simulink model "InverseKinematics_DirectionalController2018b"  (R2018b)
settings: Solver=VariableStepAuto  StartTime=0.0  StopTime=inf  RelTol=1e-3
undefined symbols (not defined in the file): f
libraries: instrumentlib x15, dspnetwork x6
(part 2 of 3)

== matlab function InverseKinematics_DirectionalController2018b/Inverse Kinematics ==
  data: p input; q1 output size=[1 1]; R input; q2 output size=[1 1]; q3 output size=[1 1]; q4 output size=[1 1]; q5 output size=[1 1]; q6 output size=[1 1]; t input
function [q1,q2,q3,q4,q5,q6] = ik_jaco(p,R,t)
%%INPUT 

%Position values from Example 7.1 research paper
%p=[x(1);y(1);z(1)];
%R=[1,0,0;0,0,-1;0,1,0]; %in the simulink model input this as a constant orientation

% ik_jaco determines the inverse kinematics of first version the 6-dof Jaco Robot 
%   The input parameters are the vector p and the matrix R. The procedure
%   taken to determine the joint angles q1,q2,q3,q4,q5,q6 is based on the
%   Polynomial Inverse Kinematic Solution of the Jaco Robot presented by
%   Clément Gosselin from the Université Laval.
% Input Arguments:
% p -> the vector position of the end-efector. p = [x,y,z]
% R -> the rotation matrix representing the orientation of the end-efector

%% Jaco Robot parameters based on the Forward Kinematic
% The following parameters are based on the paper Polynomial Inverse
% Kinematic Solution of the Jaco Robot. The below parameters can be
% changed to meet the parameters of the Jaco Robot that we have at the lab.
b__1 = 0.2755;  %Base to shoulder
a__2 = 0.2900;  %Upper arm length (shoulder to elbow)
b__3 = -0.0070; %Joint 3-4 lateral offset
b__4 = -0.1661; %Distance from elbow to first sub-segment of the first wrist 
%semgment
b__5 = -0.0856; %Distance from end of the first sub-segment to of the first
% wrist segment to end of the first sub-segment of the second wrist segment
b__6 = -0.2028; % Distance from the end of the first sub-segment of the 
% second wrist segment to the center of the hand.
s__r4 = sind(60); %55 degrees is the angle of curvature first wrist segment
s__r5 = sind(60); %55 degrees is the angle of curvature first wrist segment
c__r4 = cosd(60); %55 degrees is the angle of curvature second wrist segment
c__r5 = cosd(60); %55 degrees is the angle of curvature second wrist segment
%% Getting the end-efector orientation and position for later substitution

q__11 = R(1,1);
q__12 = R(1,2);
q__13 = R(1,3);
q__21 = R(2,1);
q__22 = R(2,2);
q__23 = R(2,3);
q__31 = R(3,1);
q__32 = R(3,2);
q__33 = R(3,3);
r__1 = p(1)+(b__6)*q__13;
r__2 = p(2)+(b__6)*q__23;
r__3 = p(3)+(b__6)*q__33;

%% V and W equations, only depends on the robot parameters and end-efector position and orientation
v__1 = -0.4e1 * ((c__r4 + 1) ^ 2) * ((q__13 * q__33 * r__1 ^ 4) + ...
    (((b__1 - r__3) * q__13 ^ 2 + 4 * q__33 * q__23 * r__2 + ...
    (b__1 - r__3) * q__23 ^ 2 + 2 * c__r5 * q__33 * b__5 - 2 * ...
    q__33 ^ 2 * b__1 + 2 * q__33 ^ 2 * r__3) * r__1 ^ 3) + ...
    (q__13 * (-6 * q__33 * r__2 ^ 2 - 3 * q__33 * b__1 ^ 2 + ...
    (2 * c__r5 * b__5 + 6 * q__33 * r__3) * b__1 - 3 * q__33 * ...
    r__3 ^ 2 - 2 * c__r5 * b__5 * r__3 + q__33 * (a__2 ^ 2 + ...
    b__3 ^ 2 - b__4 ^ 2 + b__5 ^ 2)) * r__1 ^ 2) + (((b__1 - ...
    r__3) * (a__2 ^ 2 - b__1 ^ 2 + 2 * r__3 * b__1 + b__3 ^ 2 - ...
    b__4 ^ 2 + b__5 ^ 2 - 3 * r__2 ^ 2 - r__3 ^ 2) * q__13 ^ 2 - ...
    4 * q__23 * q__33 * r__2 ^ 3 + ((-3 * b__1 + 3 * r__3) * ...
    q__23 ^ 2 - 6 * c__r5 * q__33 * b__5 + 6 * q__33 ^ 2 * b__1 - ...
    6 * q__33 ^ 2 * r__3) * r__2 ^ 2 - 2 * q__23 * (-3 * q__33 * ...
    b__1 ^ 2 + (2 * c__r5 * b__5 + 6 * q__33 * r__3) * b__1 - 3 *...
    q__33 * r__3 ^ 2 - 2 * c__r5 * b__5 * r__3 + q__33 * (a__2 ^ 2 ...
    + b__3 ^ 2 - b__4 ^ 2 + b__5 ^ 2)) * r__2 - q__23 ^ 2 * (b__1 -...
    r__3) * (a__2 ^ 2 - b__1 ^ 2 + 2 * r__3 * b__1 + b__3 ^ 2 - ...
    b__4 ^ 2 + b__5 ^ 2 - r__3 ^ 2)) * r__1) - 0.2e1 * (-(q__33 * r__2 ^ 3) ...
    / 0.2e1 + (-0.3e1 / 0.2e1 * q__33 * (b__1 ^ 2) + ((c__r5 * b__5 + 3 * q__33 * r__3)...
    * b__1) - 0.3e1 / 0.2e1 * q__33 * (r__3 ^ 2) - (c__r5 * b__5 * r__3) + ...
    (q__33 * (a__2 ^ 2 + b__3 ^ 2 - b__4 ^ 2 + b__5 ^ 2)) / 0.2e1) * r__2 +...
    (q__23 * (b__1 - r__3) * (a__2 ^ 2 - b__1 ^ 2 + 2 * r__3 * b__1 + b__3 ^ 2 -...
    b__4 ^ 2 + b__5 ^ 2 - r__3 ^ 2))) * q__13 * r__2) * b__4 * ((c__r4 - 1) ^ 2) / s__r4 ^ 3 / b__5;

v__2 = -0.4e1 * ((c__r4 + 1) ^ 2) * b__4 * (-(q__23 * q__33 * r__2 ^ 4) + ...
    (((r__3 - b__1) * q__23 ^ 2 - 4 * q__33 * r__1 * q__13 + (r__3 - b__1) ...
    * q__13 ^ 2 - 2 * c__r5 * q__33 * b__5 + 2 * q__33 ^ 2 * b__1 - 2 * ...
    q__33 ^ 2 * r__3) * r__2 ^ 3) - ((-6 * q__33 * r__1 ^ 2 - 3 * q__33 * ...
    b__1 ^ 2 + (2 * c__r5 * b__5 + 6 * q__33 * r__3) * b__1 - 3 * q__33 * ...
    r__3 ^ 2 - 2 * c__r5 * b__5 * r__3 + q__33 * (a__2 ^ 2 + b__3 ^ 2 - ...
    b__4 ^ 2 + b__5 ^ 2)) * q__23 * r__2 ^ 2) + ((-(b__1 - r__3) * ...
    (a__2 ^ 2 - b__1 ^ 2 + 2 * r__3 * b__1 + b__3 ^ 2 - b__4 ^ 2 + ...
    b__5 ^ 2 - 3 * r__1 ^ 2 - r__3 ^ 2) * q__23 ^ 2 + 4 * r__1 ^ 3 * ...
    q__13 * q__33 + ((3 * b__1 - 3 * r__3) * q__13 ^ 2 + 6 * c__r5 * ...
    q__33 * b__5 - 6 * q__33 ^ 2 * b__1 + 6 * q__33 ^ 2 * r__3) * r__1 ^ 2 ...
    + 2 * q__13 * (-3 * q__33 * b__1 ^ 2 + (2 * c__r5 * b__5 + ...
    6 * q__33 * r__3) * b__1 - 3 * q__33 * r__3 ^ 2 - 2 * c__r5 * b__5 * ...
    r__3 + q__33 * (a__2 ^ 2 + b__3 ^ 2 - b__4 ^ 2 + b__5 ^ 2)) * r__1 + ...
    q__13 ^ 2 * (b__1 - r__3) * (a__2 ^ 2 - b__1 ^ 2 + 2 * r__3 * b__1 + ...
    b__3 ^ 2 - b__4 ^ 2 + b__5 ^ 2 - r__3 ^ 2)) * r__2) + 0.2e1 * r__1 * ...
    (-(q__33 * r__1 ^ 3) / 0.2e1 + (-0.3e1 / 0.2e1 * q__33 * (b__1 ^ 2) + ...
    ((c__r5 * b__5 + 3 * q__33 * r__3) * b__1) - 0.3e1 / 0.2e1 * q__33 * ...
    (r__3 ^ 2) - (c__r5 * b__5 * r__3) + (q__33 * (a__2 ^ 2 + b__3 ^ 2 - ...
    b__4 ^ 2 + b__5 ^ 2)) / 0.2e1) * r__1 + (q__13 * (b__1 - r__3) * ...
    (a__2 ^ 2 - b__1 ^ 2 + 2 * r__3 * b__1 + b__3 ^ 2 - b__4 ^ 2 + b__5 ^ 2 ...
    - r__3 ^ 2))) * q__23) * ((c__r4 - 1) ^ 2) / s__r4 ^ 3 / b__5;

v__3 = -0.8e1 * ((c__r4 + 1) ^ 2) * ((2 * r__1 * r__2 * (b__1 - r__3) * ...
    q__13 ^ 2) + (((b__1 - r__3) * (-2 * b__4 * b__5 * c__r4 + a__2 ^ 2 -...
    b__1 ^ 2 + 2 * r__3 * b__1 + b__3 ^ 2 - b__4 ^ 2 - b__5 ^ 2 + r__1 ^ 2 ...
    + r__2 ^ 2 - r__3 ^ 2) * q__23) + (((-2 * b__4 * b__5 * c__r4 + a__2 ^ 2 -...
    5 * b__1 ^ 2 + 10 * r__3 * b__1 + b__3 ^ 2 - b__4 ^ 2 - b__5 ^ 2 + 7 * r__1 ^ 2 ...
    - r__2 ^ 2 - 5 * r__3 ^ 2) * q__33 + 2 * c__r5 * b__5 * (b__1 - r__3)) * ...
    r__2) / 0.2e1) * q__13 + (r__1 * (4 * r__2 * (b__1 - r__3) * q__23 ^ 2 + ...
    ((-2 * b__4 * b__5 * c__r4 + a__2 ^ 2 - 5 * b__1 ^ 2 + 10 * r__3 * b__1 +...
    b__3 ^ 2 - b__4 ^ 2 - b__5 ^ 2 - r__1 ^ 2 + 7 * r__2 ^ 2 - 5 * r__3 ^ 2) ...
    * q__33 + 2 * c__r5 * b__5 * (b__1 - r__3)) * q__23 + 4 * q__33 * ((-2 *...
    b__1 + 2 * r__3) * q__33 + c__r5 * b__5) * r__2)) / 0.2e1) * b__4 * b__3 ...
    * ((c__r4 - 1) ^ 2) / s__r4 ^ 3 / b__5;

v__4 = 4 * (c__r4 + 1) ^ 2 * b__4 * ((b__1 - r__3) * (-2 * b__4 * b__5 *...
    c__r4 + a__2 ^ 2 - b__1 ^ 2 + 2 * r__3 * b__1 + b__3 ^ 2 - b__4 ^ 2 ...
    - b__5 ^ 2 + 3 * r__1 ^ 2 - r__2 ^ 2 - r__3 ^ 2) * q__13 ^ 2 + ...
    (-5 * q__33 * b__1 ^ 2 + (2 * c__r5 * b__5 + 10 * q__33 * r__3) * b__1 ...
    - 5 * q__33 * r__3 ^ 2 - 2 * c__r5 * b__5 * r__3 + q__33 * (-2 * b__4 * ...
    b__5 * c__r4 + a__2 ^ 2 + b__3 ^ 2 - b__4 ^ 2 - b__5 ^ 2 + 3 * r__1 ^ 2 ...
    - 5 * r__2 ^ 2)) * r__1 * q__13 - (b__1 - r__3) * (-2 * b__4 * b__5 * ...
    c__r4 + a__2 ^ 2 - b__1 ^ 2 + 2 * r__3 * b__1 + b__3 ^ 2 - b__4 ^ 2 - ...
    b__5 ^ 2 - r__1 ^ 2 + 3 * r__2 ^ 2 - r__3 ^ 2) * q__23 ^ 2 - ...
    (-5 * q__33 * b__1 ^ 2 + (2 * c__r5 * b__5 + 10 * q__33 * r__3) * b__1 -...
    5 * q__33 * r__3 ^ 2 - 2 * c__r5 * b__5 * r__3 + q__33 * (-2 * b__4 * ...
    b__5 * c__r4 + a__2 ^ 2 + b__3 ^ 2 - b__4 ^ 2 - b__5 ^ 2 - 5 * r__1 ^ 2 + ...
    3 * r__2 ^ 2)) * r__2 * q__23 + 2 * q__33 * (r__1 - r__2) * (r__1 + r__2) ...
    * (-2 * q__33 * b__1 + c__r5 * b__5 + 2 * q__33 * r__3)) * b__3 * ...
    (c__r4 - 1) ^ 2 / s__r4 ^ 3 / b__5;

v__5 = 0.4e1 * ((c__r4 + 1) ^ 2) * ((r__1 * (b__1 - r__3) * (-2 * b__4 * ...
    b__5 * c__r4 + a__2 ^ 2 - b__1 ^ 2 + 2 * r__3 * b__1 + 3 * b__3 ^ 2 - ...
    b__4 ^ 2 - b__5 ^ 2 + r__1 ^ 2 - r__2 ^ 2 - r__3 ^ 2) * q__13 ^ 2) + ...
    ((q__33 * r__1 ^ 4) + ((-3 * q__33 * b__1 ^ 2 + (c__r5 * b__5 - ...
    r__2 * q__23 + 6 * q__33 * r__3) * b__1 - 3 * q__33 * r__3 ^ 2 + ...
    (-c__r5 * b__5 + r__2 * q__23) * r__3 + q__33 * (-2 * b__4 * b__5 ...
    * c__r4 + a__2 ^ 2 + 3 * b__3 ^ 2 - b__4 ^ 2 - b__5 ^ 2 - 4 * r__2 ^ 2))...
    * r__1 ^ 2) + ((-c__r5 * b__5 + r__2 * q__23) * b__1 ^ 3) + ...
    (((3 * c__r5 * b__5 - 3 * r__2 * q__23) * r__3) - 0.2e1 * q__33 * ...
    (-(b__4 * b__5 * c__r4) + (b__3 ^ 2) - (b__5 ^ 2) - (r__2 ^ 2) / 0.2e1)) ...
    * (b__1 ^ 2) + (((-3 * c__r5 * b__5 + 3 * r__2 * q__23) * r__3 ^ 2) + ...
    0.4e1 * q__33 * (-(b__4 * b__5 * c__r4) + (b__3 ^ 2) - (b__5 ^ 2) - ...
    (r__2 ^ 2) / 0.2e1) * r__3 - (c__r5 * b__5 ^ 3) + ((-2 * c__r4 * c__r5 * ...
    b__4 - 3 * r__2 * q__23) * b__5 ^ 2) + ((-c__r5 * r__2 ^ 2 - 2 * q__23 * ...
    b__4 * c__r4 * r__2 + c__r5 * (a__2 ^ 2 + b__3 ^ 2 - b__4 ^ 2)) * b__5) -...
    (q__23 * r__2 * (a__2 ^ 2 - b__3 ^ 2 - b__4 ^ 2 - r__2 ^ 2))) * b__1 + ...
    ((c__r5 * b__5 - r__2 * q__23) * r__3 ^ 3) - 0.2e1 * q__33 * (-(b__4 * ...
    b__5 * c__r4) + (b__3 ^ 2) - (b__5 ^ 2) - (r__2 ^ 2) / 0.2e1) * (r__3 ^ 2) ...
    + ((c__r5 * b__5 ^ 3 + (2 * c__r4 * c__r5 * b__4 + 3 * r__2 * q__23) * ...
    b__5 ^ 2 + (c__r5 * r__2 ^ 2 + 2 * q__23 * b__4 * c__r4 * r__2 - c__r5 * ...
    (a__2 ^ 2 + b__3 ^ 2 - b__4 ^ 2)) * b__5 + q__23 * r__2 * (a__2 ^ 2 - ...
    b__3 ^ 2 - b__4 ^ 2 - r__2 ^ 2)) * r__3) - (q__33 * r__2 ^ 2 * (a__2 ^ 2 ...
    + b__3 ^ 2 - b__4 ^ 2 + b__5 ^ 2 - r__2 ^ 2))) * q__13 + (r__1 * (((q__23 ^ 2 - ...
    2 * q__33 ^ 2) * b__1 + (-q__23 ^ 2 + 2 * q__33 ^ 2) * r__3 + q__33 * ...
    (c__r5 * b__5 + 3 * r__2 * q__23)) * r__1 ^ 2 + q__23 ^ 2 * b__1 ^ 3 + ...
    (-3 * q__23 ^ 2 * r__3 - q__33 * (c__r5 * b__5 - 5 * r__2 * q__23)) * ...
    b__1 ^ 2 + (3 * r__3 ^ 2 * q__23 ^ 2 + 2 * q__33 * (c__r5 * b__5 - 5 * ...
    r__2 * q__23) * r__3 + (2 * b__4 * b__5 * c__r4 - 2 * b__3 ^ 2 + 2 * ...
    b__5 ^ 2 + 4 * r__2 ^ 2) * q__33 ^ 2 - (q__23 * b__5 ^ 2 + 4 * c__r5 * ...
    r__2 * b__5 + q__23 * (a__2 ^ 2 + b__3 ^ 2 - b__4 ^ 2 + 3 * r__2 ^ 2)) ...
    * q__23) * b__1 - q__23 ^ 2 * r__3 ^ 3 - q__33 * (c__r5 * b__5 - 5 * r__2...
    * q__23) * r__3 ^ 2 + ((-2 * b__4 * b__5 * c__r4 + 2 * b__3 ^ 2 - 2 * ...
    b__5 ^ 2 - 4 * r__2 ^ 2) * q__33 ^ 2 + (q__23 * b__5 ^ 2 + 4 * c__r5 *...
    r__2 * b__5 + q__23 * (a__2 ^ 2 + b__3 ^ 2 - b__4 ^ 2 + 3 * r__2 ^ 2))...
    * q__23) * r__3 + (-c__r5 * b__5 ^ 3 + (-2 * c__r4 * c__r5 * b__4 - 3 ...
    * r__2 * q__23) * b__5 ^ 2 + (-5 * c__r5 * r__2 ^ 2 - 2 * q__23 * b__4...
    * c__r4 * r__2 + c__r5 * (a__2 ^ 2 + b__3 ^ 2 - b__4 ^ 2)) * b__5 - ...
    q__23 * r__2 * (a__2 ^ 2 - b__3 ^ 2 - b__4 ^ 2 + 3 * r__2 ^ 2)) * ...
    q__33))) * b__4 * ((c__r4 - 1) ^ 2) / s__r4 ^ 3 / b__5;

v__6 =4 * (c__r4 + 1) ^ 2 * ((b__1 - r__3) * q__23 + q__33 * r__2) * ...
    b__4 * (c__r4 - 1) ^ 2 * (2 * r__2 * (-b__4 * b__5 * c__r4 + b__3 ^ 2 ...
    - b__5 ^ 2 + r__1 ^ 2) * q__23 - c__r5 * b__5 ^ 3 + ((2 * b__1 - 2 * r__3)...
    * q__33 - 2 * c__r4 * c__r5 * b__4 - r__1 * q__13) * b__5 ^ 2 + ...
    (2 * q__33 * c__r4 * (b__1 - r__3) * b__4 - c__r5 * r__2 ^ 2 - c__r5 * ...
    b__1 ^ 2 + 2 * b__1 * c__r5 * r__3 - c__r5 * r__3 ^ 2 + c__r5 * r__1 ^ 2 ...
    - 2 * q__13 * b__4 * r__1 * c__r4 + c__r5 * (a__2 ^ 2 + b__3 ^ 2 - b__4 ^ 2))...
    * b__5 - 2 * (b__3 ^ 2 + r__1 ^ 2) * (b__1 - r__3) * q__33 + q__13 * r__1 * ...
    (a__2 ^ 2 - b__1 ^ 2 + 2 * r__3 * b__1 + 3 * b__3 ^ 2 - b__4 ^ 2 + r__1 ^ 2 ...
    - r__2 ^ 2 - r__3 ^ 2)) / s__r4 ^ 3 / b__5;

v__7 = 4 * (c__r4 + 1) ^ 2 * ((b__1 - r__3) * q__23 + q__33 * r__2) * ...
    ((-2 * b__4 * b__5 * c__r4 + a__2 ^ 2 - b__1 ^ 2 + 2 * r__3 * b__1 + ...
    b__3 ^ 2 - b__4 ^ 2 - b__5 ^ 2 + 3 * r__1 ^ 2 - r__2 ^ 2 - r__3 ^ 2) *...
    q__13 + 2 * r__1 * (2 * r__2 * q__23 + (-2 * b__1 + 2 * r__3) * q__33 +...
    c__r5 * b__5)) * b__4 * b__3 * (c__r4 - 1) ^ 2 / s__r4 ^ 3 / b__5;

w__1 = -(c__r4 + 1) ^ 3 * ((q__13 ^ 2 - q__23 ^ 2) * r__1 ^ 6 + 4 * q__13 ...
    * (-q__33 * b__1 + c__r5 * b__5 + 3 * r__2 * q__23 + q__33 * r__3) * ...
    r__1 ^ 5 + ((-15 * q__13 ^ 2 + 15 * q__23 ^ 2) * r__2 ^ 2 + 20 * q__23 ...
    * (-q__33 * b__1 + c__r5 * b__5 + q__33 * r__3) * r__2 + (-2 * a__2 ^ 2 ...
    - 2 * b__1 ^ 2 + 4 * r__3 * b__1 - 2 * b__3 ^ 2 - 2 * b__4 ^ 2 + 2 * b__5 ^ 2 ...
    - 2 * r__3 ^ 2) * q__13 ^ 2 + (-2 * a__2 ^ 2 - 2 * b__1 ^ 2 + ...
    4 * r__3 * b__1 - 2 * b__3 ^ 2 - 2 * b__4 ^ 2 + 2 * b__5 ^ 2 - ...
    2 * r__3 ^ 2) * q__23 ^ 2 + 4 * b__1 ^ 2 * q__33 ^ 2 + (-8 * ...
    c__r5 * q__33 * b__5 - 8 * q__33 ^ 2 * r__3) * b__1 + 4 * q__33 ^ 2 ...
    * r__3 ^ 2 + 8 * c__r5 * q__33 * b__5 * r__3 + 4 * c__r5 ^ 2 * b__5 ^ 2 ...
    - 4 * q__33 ^ 2 * (a__2 ^ 2 + b__3 ^ 2 - b__4 ^ 2)) * r__1 ^ 4 - 4 * ...
    (10 * r__2 ^ 3 * q__23 + (-10 * q__33 * b__1 + 10 * c__r5 * b__5 + ...
    10 * q__33 * r__3) * r__2 ^ 2 - b__1 ^ 3 * q__33 + (c__r5 * b__5 + 3 ...
    * q__33 * r__3) * b__1 ^ 2 + (-3 * q__33 * r__3 ^ 2 - 2 * c__r5 * b__5 ...
    * r__3 + q__33 * (a__2 ^ 2 + b__3 ^ 2 - 3 * b__4 ^ 2 + b__5 ^ 2)) * ...
    b__1 + q__33 * r__3 ^ 3 + c__r5 * b__5 * r__3 ^ 2 - q__33 * (a__2 ^ 2 ...
    + b__3 ^ 2 - 3 * b__4 ^ 2 + b__5 ^ 2) * r__3 + c__r5 * b__5 * (a__2 ^ 2 ...
    + b__3 ^ 2 + b__4 ^ 2 - b__5 ^ 2)) * q__13 * r__1 ^ 3 + ((15 * q__13 ^ 2 - ...
    15 * q__23 ^ 2) * r__2 ^ 4 - 40 * q__23 * (-q__33 * b__1 + c__r5 * b__5 ...
    + q__33 * r__3) * r__2 ^ 3 + ((12 * a__2 ^ 2 + 12 * b__1 ^ 2 - 24 * ...
    r__3 * b__1 + 12 * b__3 ^ 2 + 12 * b__4 ^ 2 - 12 * b__5 ^ 2 + 12 * ...
    r__3 ^ 2) * q__13 ^ 2 + (12 * a__2 ^ 2 + 12 * b__1 ^ 2 - 24 * r__3 * ...
    b__1 + 12 * b__3 ^ 2 + 12 * b__4 ^ 2 - 12 * b__5 ^ 2 + 12 * r__3 ^ 2) ...
    * q__23 ^ 2 - 24 * b__1 ^ 2 * q__33 ^ 2 + (48 * c__r5 * q__33 * b__5 + ...
    48 * q__33 ^ 2 * r__3) * b__1 - 24 * q__33 ^ 2 * r__3 ^ 2 - 48 * c__r5 ...
    * q__33 * b__5 * r__3 - 24 * c__r5 ^ 2 * b__5 ^ 2 + 24 * q__33 ^ 2 * ...
    (a__2 ^ 2 + b__3 ^ 2 - b__4 ^ 2)) * r__2 ^ 2 + 12 * (-b__1 ^ 3 * q__33 ...
    + (c__r5 * b__5 + 3 * q__33 * r__3) * b__1 ^ 2 + (-3 * q__33 * r__3 ^ 2 ...
    - 2 * c__r5 * b__5 * r__3 + q__33 * (a__2 ^ 2 + b__3 ^ 2 - 3 * b__4 ^ 2 +...
    b__5 ^ 2)) * b__1 + q__33 * r__3 ^ 3 + c__r5 * b__5 * r__3 ^ 2 - q__33 * ...
    (a__2 ^ 2 + b__3 ^ 2 - 3 * b__4 ^ 2 + b__5 ^ 2) * r__3 + c__r5 * b__5 * ...
    (a__2 ^ 2 + b__3 ^ 2 + b__4 ^ 2 - b__5 ^ 2)) * q__23 * r__2 + (b__1 ^ 4 ...
    - 4 * r__3 * b__1 ^ 3 + (-2 * a__2 ^ 2 - 2 * b__3 ^ 2 + 6 * b__4 ^ 2 - ...
    2 * b__5 ^ 2 + 6 * r__3 ^ 2) * b__1 ^ 2 + 4 * r__3 * (a__2 ^ 2 + b__3 ^ ...
    2 - 3 * b__4 ^ 2 + b__5 ^ 2 - r__3 ^ 2) * b__1 + r__3 ^ 4 + (-2 * a__2 ^ ...
    2 - 2 * b__3 ^ 2 + 6 * b__4 ^ 2 - 2 * b__5 ^ 2) * r__3 ^ 2 + (a__2 ^ 2 + ...
    b__3 ^ 2 - b__4 ^ 2 + 2 * b__4 * b__5 - b__5 ^ 2) * (a__2 ^ 2 + b__3 ^ 2 ...
    - b__4 ^ 2 - 2 * b__4 * b__5 - b__5 ^ 2)) * (q__13 - q__23) * (q__13 + ...
    q__23)) * r__1 ^ 2 - 4 * q__13 * (-3 * r__2 ^ 4 * q__23 + (5 * q__33 * ...
    b__1 - 5 * c__r5 * b__5 - 5 * q__33 * r__3) * r__2 ^ 3 + (3 * b__1 ^ 3 ...
    * q__33 + (-3 * c__r5 * b__5 - 9 * q__33 * r__3) * b__1 ^ 2 + (9 * q__33...
    * r__3 ^ 2 + 6 * c__r5 * b__5 * r__3 - 3 * q__33 * (a__2 ^ 2 + b__3 ^ 2 ...
    - 3 * b__4 ^ 2 + b__5 ^ 2)) * b__1 - 3 * q__33 * r__3 ^ 3 - 3 * c__r5 * ...
    b__5 * r__3 ^ 2 + 3 * q__33 * (a__2 ^ 2 + b__3 ^ 2 - 3 * b__4 ^ 2 + ...
    b__5 ^ 2) * r__3 - 3 * c__r5 * b__5 * (a__2 ^ 2 + b__3 ^ 2 + b__4 ^ 2 ...
    - b__5 ^ 2)) * r__2 + (b__1 ^ 4 - 4 * r__3 * b__1 ^ 3 + (-2 * a__2 ^ 2 ...
    - 2 * b__3 ^ 2 + 6 * b__4 ^ 2 - 2 * b__5 ^ 2 + 6 * r__3 ^ 2) * b__1 ^ 2 ...
    + 4 * r__3 * (a__2 ^ 2 + b__3 ^ 2 - 3 * b__4 ^ 2 + b__5 ^ 2 - r__3 ^ 2) ...
    * b__1 + r__3 ^ 4 + (-2 * a__2 ^ 2 - 2 * b__3 ^ 2 + 6 * b__4 ^ 2 - 2 *...
    b__5 ^ 2) * r__3 ^ 2 + (a__2 ^ 2 + b__3 ^ 2 - b__4 ^ 2 + 2 * b__4 * b__5 ...
    - b__5 ^ 2) * (a__2 ^ 2 + b__3 ^ 2 - b__4 ^ 2 - 2 * b__4 * b__5 - b__5 ^ 2))...
    * q__23) * r__2 * r__1 - r__2 ^ 2 * ((q__13 ^ 2 - q__23 ^ 2) * r__2 ^ 4 -...
    4 * q__23 * (-q__33 * b__1 + c__r5 * b__5 + q__33 * r__3) * r__2 ^ 3 + ...
    ((2 * a__2 ^ 2 + 2 * b__1 ^ 2 - 4 * r__3 * b__1 + 2 * b__3 ^ 2 + 2 * ...
    b__4 ^ 2 - 2 * b__5 ^ 2 + 2 * r__3 ^ 2) * q__13 ^ 2 + (2 * a__2 ^ 2 + ...
    2 * b__1 ^ 2 - 4 * r__3 * b__1 + 2 * b__3 ^ 2 + 2 * b__4 ^ 2 - 2 * b__5 ^ 2 ...
    + 2 * r__3 ^ 2) * q__23 ^ 2 - 4 * b__1 ^ 2 * q__33 ^ 2 + (8 * c__r5 * q__33 ...
    * b__5 + 8 * q__33 ^ 2 * r__3) * b__1 - 4 * q__33 ^ 2 * r__3 ^ 2 - 8 * ...
    c__r5 * q__33 * b__5 * r__3 - 4 * c__r5 ^ 2 * b__5 ^ 2 + 4 * q__33 ^ 2 * ...
    (a__2 ^ 2 + b__3 ^ 2 - b__4 ^ 2)) * r__2 ^ 2 + 4 * (-b__1 ^ 3 * q__33 + ...
    (c__r5 * b__5 + 3 * q__33 * r__3) * b__1 ^ 2 + (-3 * q__33 * r__3 ^ 2 - ...
    2 * c__r5 * b__5 * r__3 + q__33 * (a__2 ^ 2 + b__3 ^ 2 - 3 * b__4 ^ 2 + ...
    b__5 ^ 2)) * b__1 + q__33 * r__3 ^ 3 + c__r5 * b__5 * r__3 ^ 2 - q__33 * ...
    (a__2 ^ 2 + b__3 ^ 2 - 3 * b__4 ^ 2 + b__5 ^ 2) * r__3 + c__r5 * b__5 * ...
    (a__2 ^ 2 + b__3 ^ 2 + b__4 ^ 2 - b__5 ^ 2)) * q__23 * r__2 + (b__1 ^ 4 ...
    - 4 * r__3 * b__1 ^ 3 + (-2 * a__2 ^ 2 - 2 * b__3 ^ 2 + 6 * b__4 ^ 2 - 2 ...
    * b__5 ^ 2 + 6 * r__3 ^ 2) * b__1 ^ 2 + 4 * r__3 * (a__2 ^ 2 + b__3 ^ 2 ...
    - 3 * b__4 ^ 2 + b__5 ^ 2 - r__3 ^ 2) * b__1 + r__3 ^ 4 + (-2 * a__2 ^ 2 ...
    - 2 * b__3 ^ 2 + 6 * b__4 ^ 2 - 2 * b__5 ^ 2) * r__3 ^ 2 + (a__2 ^ 2 + ...
    b__3 ^ 2 - b__4 ^ 2 + 2 * b__4 * b__5 - b__5 ^ 2) * (a__2 ^ 2 + b__3 ^ 2 ...
    - b__4 ^ 2 - 2 * b__4 * b__5 - b__5 ^ 2)) * (q__13 - q__23) * (q__13 + q__23)))...
    * (c__r4 - 1) ^ 3 / s__r4 ^ 6 / b__5 ^ 2;

w__2 =-0.2e1 * ((c__r4 + 1) ^ 3) * (-(q__13 * q__23 * r__1 ^ 6) + ...
    (((3 * q__13 ^ 2 - 3 * q__23 ^ 2) * r__2 - 2 * q__23 * (-q__33 *...
    b__1 + c__r5 * b__5 + q__33 * r__3)) * r__1 ^ 5) + 0.10e2 * q__13 * ...
    ((c__r5 * b__5) + 0.3e1 / 0.2e1 * r__2 * q__23 - (q__33 * b__1) + ...
    (q__33 * r__3)) * r__2 * (r__1 ^ 4) + (((-10 * q__13 ^ 2 + 10 * ...
    q__23 ^ 2) * r__2 ^ 3 + 20 * q__23 * (-q__33 * b__1 + c__r5 * b__5 + ...
    q__33 * r__3) * r__2 ^ 2 + ((-4 * a__2 ^ 2 - 4 * b__1 ^ 2 + 8 * r__3 * ...
    b__1 - 4 * b__3 ^ 2 - 4 * b__4 ^ 2 + 4 * b__5 ^ 2 - 4 * r__3 ^ 2) * ...
    q__13 ^ 2 + (-4 * a__2 ^ 2 - 4 * b__1 ^ 2 + 8 * r__3 * b__1 - 4 *...
    b__3 ^ 2 - 4 * b__4 ^ 2 + 4 * b__5 ^ 2 - 4 * r__3 ^ 2) * q__23 ^ 2 + ...
    8 * b__1 ^ 2 * q__33 ^ 2 + (-16 * c__r5 * q__33 * b__5 - 16 * q__33 ^ 2 ...
    * r__3) * b__1 + 8 * q__33 ^ 2 * r__3 ^ 2 + 16 * c__r5 * q__33 * b__5 *...
    r__3 + 8 * c__r5 ^ 2 * b__5 ^ 2 - 8 * q__33 ^ 2 * (a__2 ^ 2 + b__3 ^ 2 ...
    - b__4 ^ 2)) * r__2 - 2 * (-b__1 ^ 3 * q__33 + (c__r5 * b__5 + 3 * ...
    q__33 * r__3) * b__1 ^ 2 + (-3 * q__33 * r__3 ^ 2 - 2 * c__r5 * b__5 * ...
    r__3 + q__33 * (a__2 ^ 2 + b__3 ^ 2 - 3 * b__4 ^ 2 + b__5 ^ 2)) * b__1 +...
    q__33 * r__3 ^ 3 + c__r5 * b__5 * r__3 ^ 2 - q__33 * (a__2 ^ 2 + ...
    b__3 ^ 2 - 3 * b__4 ^ 2 + b__5 ^ 2) * r__3 + c__r5 * b__5 * (a__2 ^ 2 +...
    b__3 ^ 2 + b__4 ^ 2 - b__5 ^ 2)) * q__23) * r__1 ^ 3) + ((-15 * r__2 ^ 4 ...
    * q__23 + (20 * q__33 * b__1 - 20 * c__r5 * b__5 - 20 * q__33 * r__3) * ...
    r__2 ^ 3 + (6 * b__1 ^ 3 * q__33 + (-6 * c__r5 * b__5 - 18 * q__33 * r__3) ...
    * b__1 ^ 2 + (18 * q__33 * r__3 ^ 2 + 12 * c__r5 * b__5 * r__3 - 6 * q__33 ...
    * (a__2 ^ 2 + b__3 ^ 2 - 3 * b__4 ^ 2 + b__5 ^ 2)) * b__1 - 6 * q__33 * ...
    r__3 ^ 3 - 6 * c__r5 * b__5 * r__3 ^ 2 + 6 * q__33 * (a__2 ^ 2 + b__3 ^ 2 ...
    - 3 * b__4 ^ 2 + b__5 ^ 2) * r__3 - 6 * c__r5 * b__5 * (a__2 ^ 2 + b__3 ^ 2 ...
    + b__4 ^ 2 - b__5 ^ 2)) * r__2 + (b__1 ^ 4 - 4 * r__3 * b__1 ^ 3 + ...
    (-2 * a__2 ^ 2 - 2 * b__3 ^ 2 + 6 * b__4 ^ 2 - 2 * b__5 ^ 2 + 6 * r__3 ^ 2)...
    * b__1 ^ 2 + 4 * r__3 * (a__2 ^ 2 + b__3 ^ 2 - 3 * b__4 ^ 2 + b__5 ^ 2 - ...
    r__3 ^ 2) * b__1 + r__3 ^ 4 + (-2 * a__2 ^ 2 - 2 * b__3 ^ 2 + 6 * b__4 ^ 2 ...
    - 2 * b__5 ^ 2) * r__3 ^ 2 + (a__2 ^ 2 + b__3 ^ 2 - b__4 ^ 2 + 2 * b__4 * ...
    b__5 - b__5 ^ 2) * (a__2 ^ 2 + b__3 ^ 2 - b__4 ^ 2 - 2 * b__4 * b__5 - ...
    b__5 ^ 2)) * q__23) * q__13 * r__1 ^ 2) + (r__2 * ((3 * q__13 ^ 2 - 3 * ...
    q__23 ^ 2) * r__2 ^ 4 - 10 * q__23 * (-q__33 * b__1 + c__r5 * b__5 + ...
    q__33 * r__3) * r__2 ^ 3 + ((4 * a__2 ^ 2 + 4 * b__1 ^ 2 - 8 * r__3 * ...
    b__1 + 4 * b__3 ^ 2 + 4 * b__4 ^ 2 - 4 * b__5 ^ 2 + 4 * r__3 ^ 2) * ...
    q__13 ^ 2 + (4 * a__2 ^ 2 + 4 * b__1 ^ 2 - 8 * r__3 * b__1 + 4 * b__3 ^ 2 ...
    + 4 * b__4 ^ 2 - 4 * b__5 ^ 2 + 4 * r__3 ^ 2) * q__23 ^ 2 - 8 * b__1 ^ 2 *...
    q__33 ^ 2 + (16 * c__r5 * q__33 * b__5 + 16 * q__33 ^ 2 * r__3) * b__1 - ...
    8 * q__33 ^ 2 * r__3 ^ 2 - 16 * c__r5 * q__33 * b__5 * r__3 - 8 * c__r5 ^ 2 ...
    * b__5 ^ 2 + 8 * q__33 ^ 2 * (a__2 ^ 2 + b__3 ^ 2 - b__4 ^ 2)) * r__2 ^ 2 + ...
    6 * (-b__1 ^ 3 * q__33 + (c__r5 * b__5 + 3 * q__33 * r__3) * b__1 ^ 2 + ...
    (-3 * q__33 * r__3 ^ 2 - 2 * c__r5 * b__5 * r__3 + q__33 * (a__2 ^ 2 + ...
    b__3 ^ 2 - 3 * b__4 ^ 2 + b__5 ^ 2)) * b__1 + q__33 * r__3 ^ 3 + c__r5 *...
    b__5 * r__3 ^ 2 - q__33 * (a__2 ^ 2 + b__3 ^ 2 - 3 * b__4 ^ 2 + b__5 ^ 2) ...
    * r__3 + c__r5 * b__5 * (a__2 ^ 2 + b__3 ^ 2 + b__4 ^ 2 - b__5 ^ 2)) * ...
    q__23 * r__2 + (b__1 ^ 4 - 4 * r__3 * b__1 ^ 3 + (-2 * a__2 ^ 2 - 2 * ...
    b__3 ^ 2 + 6 * b__4 ^ 2 - 2 * b__5 ^ 2 + 6 * r__3 ^ 2) * b__1 ^ 2 + ...
    4 * r__3 * (a__2 ^ 2 + b__3 ^ 2 - 3 * b__4 ^ 2 + b__5 ^ 2 - r__3 ^ 2) ...
    * b__1 + r__3 ^ 4 + (-2 * a__2 ^ 2 - 2 * b__3 ^ 2 + 6 * b__4 ^ 2 - 2 *...
    b__5 ^ 2) * r__3 ^ 2 + (a__2 ^ 2 + b__3 ^ 2 - b__4 ^ 2 + 2 * b__4 * ...
    b__5 - b__5 ^ 2) * (a__2 ^ 2 + b__3 ^ 2 - b__4 ^ 2 - 2 * b__4 * b__5 -...
    b__5 ^ 2)) * (q__13 - q__23) * (q__13 + q__23)) * r__1) - (q__13 * ...
    (-r__2 ^ 4 * q__23 + (2 * q__33 * b__1 - 2 * c__r5 * b__5 - 2 * ...
    q__33 * r__3) * r__2 ^ 3 + (2 * b__1 ^ 3 * q__33 + (-2 * c__r5 * b__5 ...
    - 6 * q__33 * r__3) * b__1 ^ 2 + (6 * q__33 * r__3 ^ 2 + 4 * c__r5 * ...
    b__5 * r__3 - 2 * q__33 * (a__2 ^ 2 + b__3 ^ 2 - 3 * b__4 ^ 2 + b__5 ^ 2)) ...
    * b__1 - 2 * q__33 * r__3 ^ 3 - 2 * c__r5 * b__5 * r__3 ^ 2 + 2 * q__33 * ...
    (a__2 ^ 2 + b__3 ^ 2 - 3 * b__4 ^ 2 + b__5 ^ 2) * r__3 - 2 * c__r5 * b__5 *...
    (a__2 ^ 2 + b__3 ^ 2 + b__4 ^ 2 - b__5 ^ 2)) * r__2 + (b__1 ^ 4 - 4 * r__3 *...
    b__1 ^ 3 + (-2 * a__2 ^ 2 - 2 * b__3 ^ 2 + 6 * b__4 ^ 2 - 2 * b__5 ^ 2 + 6 *...
    r__3 ^ 2) * b__1 ^ 2 + 4 * r__3 * (a__2 ^ 2 + b__3 ^ 2 - 3 * b__4 ^ 2 + b__5 ^ 2 ...
    - r__3 ^ 2) * b__1 + r__3 ^ 4 + (-2 * a__2 ^ 2 - 2 * b__3 ^ 2 + 6 * b__4 ^ 2 - ...
    2 * b__5 ^ 2) * r__3 ^ 2 + (a__2 ^ 2 + b__3 ^ 2 - b__4 ^ 2 + 2 * b__4 * b__5 - ...
    b__5 ^ 2) * (a__2 ^ 2 + b__3 ^ 2 - b__4 ^ 2 - 2 * b__4 * b__5 - b__5 ^ 2)) *...
    q__23) * r__2 ^ 2)) * ((c__r4 - 1) ^ 3) / s__r4 ^ 6 / (b__5 ^ 2);

w__3 =-0.2e1 * ((c__r4 + 1) ^ 3) * b__3 * ((c__r4 - 1) ^ 3) * (((3 * q__13 ^ 2 - q__23 ^ 2 + 2 * q__33 ^ 2) * r__2 ^ 5) - 0.4e1 * ((5 * r__1 * q__13) + c__r5 * b__5 - 0.5e1 / 0.2e1 * q__33 * (b__1 - r__3)) * q__23 * (r__2 ^ 4) + ((-0.2e1 * b__4 * b__5 * c__r4 + (2 * a__2 ^ 2) + (6 * b__1 ^ 2) - (12 * r__3 * b__1) + (2 * b__3 ^ 2) + 0.2e1 * b__4 ^ 2 - 0.2e1 * b__5 ^ 2 + (18 * r__1 ^ 2) + (6 * r__3 ^ 2)) * (q__23 ^ 2) + ((-22 * q__13 ^ 2 - 4 * q__33 ^ 2) * r__1 ^ 2) - 0.28e2 * q__13 * (c__r5 * b__5 - (q__33 * (b__1 - r__3))) * r__1 + (-0.2e1 * b__4 * b__5 * c__r4 + (4 * a__2 ^ 2) + (4 * b__1 ^ 2) - (8 * r__3 * b__1) + (4 * b__3 ^ 2) - 0.4e1 * b__5 ^ 2 + (4 * r__3 ^ 2)) * (q__13 ^ 2) + (-0.4e1 * c__r5 ^ 2 - (2 * q__33 ^ 2)) * b__5 ^ 2 + 0.12e2 * q__33 * (-c__r4 * q__33 * b__4 / 0.3e1 + c__r5 * b__1 - c__r5 * r__3) * b__5 + 0.6e1 * (q__33 ^ 2) * ((a__2 ^ 2) - (b__1 ^ 2) + (2 * r__3 * b__1) + (b__3 ^ 2) - b__4 ^ 2 - (r__3 ^ 2))) * (r__2 ^ 3) + 0.4e1 * ((10 * q__13 * r__1 ^ 3) + (0.9e1 * c__r5 * b__5 - (12 * q__33 * (b__1 - r__3))) * (r__1 ^ 2) + q__13 * ((a__2 ^ 2) - (b__1 ^ 2) + (2 * r__3 * b__1) + (b__3 ^ 2) - b__4 ^ 2 - b__5 ^ 2 - (r__3 ^ 2)) * r__1 / 0.2e1 - c__r5 * b__5 ^ 3 + ((q__33 * b__1) / 0.2e1 - (q__33 * r__3) / 0.2e1 - c__r4 * c__r5 * b__4) * b__5 ^ 2 + (0.2e1 * c__r5 * (b__1 ^ 2) + (-c__r4 * q__33 * b__4 - 0.4e1 * c__r5 * r__3) * b__1 + 0.2e1 * c__r5 * (r__3 ^ 2) + q__33 * b__4 * r__3 * c__r4 + c__r5 * (a__2 ^ 2 + b__3 ^ 2)) * b__5 + 0.3e1 / 0.2e1 * q__33 * ((a__2 ^ 2) - (b__1 ^ 2) + (2 * r__3 * b__1) + (b__3 ^ 2) - 0.7e1 / 0.3e1 * b__4 ^ 2 - (r__3 ^ 2)) * (b__1 - r__3)) * q__23 * (r__2 ^ 2) + ((-(13 * r__1 ^ 4) + (0.6e1 * b__4 * b__5 * c__r4 - (10 * a__2 ^ 2) - (14 * b__1 ^ 2) + (28 * r__3 * b__1) - (10 * b__3 ^ 2) - 0.2e1 * b__4 ^ 2 + 0.10e2 * b__5 ^ 2 - (14 * r__3 ^ 2)) * (r__1 ^ 2) - b__5 ^ 4 - 0.2e1 * b__4 * c__r4 * b__5 ^ 3 + ((2 * a__2 ^ 2) + (2 * b__1 ^ 2) - (4 * r__3 * b__1) + (2 * b__3 ^ 2) - 0.2e1 * b__4 ^ 2 + (2 * r__3 ^ 2)) * b__5 ^ 2 + 0.2e1 * b__4 * c__r4 * ((a__2 ^ 2) - (b__1 ^ 2) + (2 * r__3 * b__1) + (b__3 ^ 2) - b__4 ^ 2 - (r__3 ^ 2)) * b__5 - (b__1 ^ 4) + (4 * r__3 * b__1 ^ 3) + ((2 * a__2 ^ 2) + (2 * b__3 ^ 2) - 0.6e1 * b__4 ^ 2 - (6 * r__3 ^ 2)) * (b__1 ^ 2) - 0.4e1 * r__3 * ((a__2 ^ 2) + (b__3 ^ 2) - 0.3e1 * b__4 ^ 2 - (r__3 ^ 2)) * b__1 - (r__3 ^ 4) + ((2 * a__2 ^ 2) + (2 * b__3 ^ 2) - 0.6e1 * b__4 ^ 2) * (r__3 ^ 2) - ((a__2 ^ 2) + (b__3 ^ 2) - b__4 ^ 2) ^ 2) * (q__23 ^ 2) + ((7 * q__13 ^ 2 - 6 * q__33 ^ 2) * r__1 ^ 4) + 0.20e2 * q__13 * (c__r5 * b__5 - 0.9e1 / 0.5e1 * q__33 * (b__1 - r__3)) * (r__1 ^ 3) + ((0.6e1 * b__4 * b__5 * c__r4 - (8 * a__2 ^ 2) - (16 * b__1 ^ 2) + (32 * r__3 * b__1) - (8 * b__3 ^ 2) - 0.4e1 * b__4 ^ 2 + 0.8e1 * b__5 ^ 2 - (16 * r__3 ^ 2)) * (q__13 ^ 2) + (0.12e2 * c__r5 ^ 2 + (6 * q__33 ^ 2)) * b__5 ^ 2 - 0.36e2 * q__33 * (-c__r4 * q__33 * b__4 / 0.3e1 + c__r5 * b__1 - c__r5 * r__3) * b__5 - 0.18e2 * (q__33 ^ 2) * ((a__2 ^ 2) - (b__1 ^ 2) + (2 * r__3 * b__1) + (b__3 ^ 2) - b__4 ^ 2 - (r__3 ^ 2))) * (r__1 ^ 2) - 0.8e1 * q__13 * (-c__r5 * b__5 ^ 3 + ((q__33 * b__1) / 0.2e1 - (q__33 * r__3) / 0.2e1 - c__r4 * c__r5 * b__4) * b__5 ^ 2 + (0.2e1 * c__r5 * (b__1 ^ 2) + (-c__r4 * q__33 * b__4 - 0.4e1 * c__r5 * r__3) * b__1 + 0.2e1 * c__r5 * (r__3 ^ 2) + q__33 * b__4 * r__3 * c__r4 + c__r5 * (a__2 ^ 2 + b__3 ^ 2)) * b__5 + 0.3e1 / 0.2e1 * q__33 * ((a__2 ^ 2) - (b__1 ^ 2) + (2 * r__3 * b__1) + (b__3 ^ 2) - 0.7e1 / 0.3e1 * b__4 ^ 2 - (r__3 ^ 2)) * (b__1 - r__3)) * r__1 + (q__13 ^ 2) * (b__5 ^ 4 + 0.2e1 * b__4 * c__r4 * b__5 ^ 3 + (-(2 * a__2 ^ 2) - (2 * b__1 ^ 2) + (4 * r__3 * b__1) - (2 * b__3 ^ 2) + 0.2e1 * b__4 ^ 2 - (2 * r__3 ^ 2)) * b__5 ^ 2 - 0.2e1 * b__4 * c__r4 * ((a__2 ^ 2) - (b__1 ^ 2) + (2 * r__3 * b__1) + (b__3 ^ 2) - b__4 ^ 2 - (r__3 ^ 2)) * b__5 + (b__1 ^ 4) - (4 * r__3 * b__1 ^ 3) + (-(2 * a__2 ^ 2) - (2 * b__3 ^ 2) + 0.6e1 * b__4 ^ 2 + (6 * r__3 ^ 2)) * (b__1 ^ 2) + 0.4e1 * r__3 * ((a__2 ^ 2) + (b__3 ^ 2) - 0.3e1 * b__4 ^ 2 - (r__3 ^ 2)) * b__1 + (r__3 ^ 4) + (-(2 * a__2 ^ 2) - (2 * b__3 ^ 2) + 0.6e1 * b__4 ^ 2) * (r__3 ^ 2) + ((a__2 ^ 2) + (b__3 ^ 2) - b__4 ^ 2) ^ 2)) * r__2 + 0.2e1 * r__1 * (-(2 * q__13 * r__1 ^ 4) + (-0.4e1 * c__r5 * b__5 + (3 * q__33 * (b__1 - r__3))) * (r__1 ^ 3) + q__13 * ((a__2 ^ 2) - (b__1 ^ 2) + (2 * r__3 * b__1) + (b__3 ^ 2) - b__4 ^ 2 - b__5 ^ 2 - (r__3 ^ 2)) * (r__1 ^ 2) + (0.2e1 * c__r5 * b__5 ^ 3 + (0.2e1 * c__r4 * c__r5 * b__4 - (q__33 * b__1) + (q__33 * r__3)) * b__5 ^ 2 + (-0.4e1 * c__r5 * (b__1 ^ 2) + (0.2e1 * c__r4 * q__33 * b__4 + 0.8e1 * c__r5 * r__3) * b__1 - 0.4e1 * c__r5 * (r__3 ^ 2) - 0.2e1 * q__33 * b__4 * r__3 * c__r4 - 0.2e1 * c__r5 * (a__2 ^ 2 + b__3 ^ 2)) * b__5 - 0.3e1 * q__33 * ((a__2 ^ 2) - (b__1 ^ 2) + (2 * r__3 * b__1) + (b__3 ^ 2) - 0.7e1 / 0.3e1 * b__4 ^ 2 - (r__3 ^ 2)) * (b__1 - r__3)) * r__1 + q__13 * (b__5 ^ 4 + 0.2e1 * b__4 * c__r4 * b__5 ^ 3 + (-(2 * a__2 ^ 2) - (2 * b__1 ^ 2) + (4 * r__3 * b__1) - (2 * b__3 ^ 2) + 0.2e1 * b__4 ^ 2 - (2 * r__3 ^ 2)) * b__5 ^ 2 - 0.2e1 * b__4 * c__r4 * ((a__2 ^ 2) - (b__1 ^ 2) + (2 * r__3 * b__1) + (b__3 ^ 2) - b__4 ^ 2 - (r__3 ^ 2)) * b__5 + (b__1 ^ 4) - (4 * r__3 * b__1 ^ 3) + (-(2 * a__2 ^ 2) - (2 * b__3 ^ 2) + 0.6e1 * b__4 ^ 2 + (6 * r__3 ^ 2)) * (b__1 ^ 2) + 0.4e1 * r__3 * ((a__2 ^ 2) + (b__3 ^ 2) - 0.3e1 * b__4 ^ 2 - (r__3 ^ 2)) * b__1 + (r__3 ^ 4) + (-(2 * a__2 ^ 2) - (2 * b__3 ^ 2) + 0.6e1 * b__4 ^ 2) * (r__3 ^ 2) + ((a__2 ^ 2) + (b__3 ^ 2) - b__4 ^ 2) ^ 2)) * q__23) / s__r4 ^ 6 / b__5 ^ 2;

w__4 =0.2e1 * ((c__r4 + 1) ^ 3) * (((q__13 ^ 2 - 3 * q__23 ^ 2 - 2 * q__33 ^ 2) * r__1 ^ 5) + 0.4e1 * q__13 * ((5 * r__2 * q__23) + c__r5 * b__5 - 0.5e1 / 0.2e1 * q__33 * (b__1 - r__3)) * (r__1 ^ 4) + ((0.2e1 * b__4 * b__5 * c__r4 - (2 * a__2 ^ 2) - (6 * b__1 ^ 2) + (12 * r__3 * b__1) - (2 * b__3 ^ 2) - 0.2e1 * b__4 ^ 2 + 0.2e1 * b__5 ^ 2 - (18 * r__2 ^ 2) - (6 * r__3 ^ 2)) * (q__13 ^ 2) + ((22 * q__23 ^ 2 + 4 * q__33 ^ 2) * r__2 ^ 2) + 0.28e2 * (c__r5 * b__5 - (q__33 * (b__1 - r__3))) * q__23 * r__2 + (0.2e1 * b__4 * b__5 * c__r4 - (4 * a__2 ^ 2) - (4 * b__1 ^ 2) + (8 * r__3 * b__1) - (4 * b__3 ^ 2) + 0.4e1 * b__5 ^ 2 - (4 * r__3 ^ 2)) * (q__23 ^ 2) + (0.4e1 * c__r5 ^ 2 + (2 * q__33 ^ 2)) * b__5 ^ 2 - 0.12e2 * q__33 * (-c__r4 * q__33 * b__4 / 0.3e1 + c__r5 * b__1 - c__r5 * r__3) * b__5 - 0.6e1 * (q__33 ^ 2) * ((a__2 ^ 2) - (b__1 ^ 2) + (2 * r__3 * b__1) + (b__3 ^ 2) - b__4 ^ 2 - (r__3 ^ 2))) * (r__1 ^ 3) - 0.4e1 * ((10 * r__2 ^ 3 * q__23) + (0.9e1 * c__r5 * b__5 - (12 * q__33 * (b__1 - r__3))) * (r__2 ^ 2) + q__23 * ((a__2 ^ 2) - (b__1 ^ 2) + (2 * r__3 * b__1) + (b__3 ^ 2) - b__4 ^ 2 - b__5 ^ 2 - (r__3 ^ 2)) * r__2 / 0.2e1 - c__r5 * b__5 ^ 3 + ((q__33 * b__1) / 0.2e1 - (q__33 * r__3) / 0.2e1 - c__r4 * c__r5 * b__4) * b__5 ^ 2 + (0.2e1 * c__r5 * (b__1 ^ 2) + (-c__r4 * q__33 * b__4 - 0.4e1 * c__r5 * r__3) * b__1 + 0.2e1 * c__r5 * (r__3 ^ 2) + q__33 * b__4 * r__3 * c__r4 + c__r5 * (a__2 ^ 2 + b__3 ^ 2)) * b__5 + 0.3e1 / 0.2e1 * q__33 * ((a__2 ^ 2) - (b__1 ^ 2) + (2 * r__3 * b__1) + (b__3 ^ 2) - 0.7e1 / 0.3e1 * b__4 ^ 2 - (r__3 ^ 2)) * (b__1 - r__3)) * q__13 * (r__1 ^ 2) + (((13 * r__2 ^ 4) + (-0.6e1 * b__4 * b__5 * c__r4 + (10 * a__2 ^ 2) + (14 * b__1 ^ 2) - (28 * r__3 * b__1) + (10 * b__3 ^ 2) + 0.2e1 * b__4 ^ 2 - 0.10e2 * b__5 ^ 2 + (14 * r__3 ^ 2)) * (r__2 ^ 2) + b__5 ^ 4 + 0.2e1 * b__4 * c__r4 * b__5 ^ 3 + (-(2 * a__2 ^ 2) - (2 * b__1 ^ 2) + (4 * r__3 * b__1) - (2 * b__3 ^ 2) + 0.2e1 * b__4 ^ 2 - (2 * r__3 ^ 2)) * b__5 ^ 2 - 0.2e1 * b__4 * c__r4 * ((a__2 ^ 2) - (b__1 ^ 2) + (2 * r__3 * b__1) + (b__3 ^ 2) - b__4 ^ 2 - (r__3 ^ 2)) * b__5 + (b__1 ^ 4) - (4 * r__3 * b__1 ^ 3) + (-(2 * a__2 ^ 2) - (2 * b__3 ^ 2) + 0.6e1 * b__4 ^ 2 + (6 * r__3 ^ 2)) * (b__1 ^ 2) + 0.4e1 * r__3 * ((a__2 ^ 2) + (b__3 ^ 2) - 0.3e1 * b__4 ^ 2 - (r__3 ^ 2)) * b__1 + (r__3 ^ 4) + (-(2 * a__2 ^ 2) - (2 * b__3 ^ 2) + 0.6e1 * b__4 ^ 2) * (r__3 ^ 2) + ((a__2 ^ 2) + (b__3 ^ 2) - b__4 ^ 2) ^ 2) * (q__13 ^ 2) + ((-7 * q__23 ^ 2 + 6 * q__33 ^ 2) * r__2 ^ 4) - 0.20e2 * (c__r5 * b__5 - 0.9e1 / 0.5e1 * q__33 * (b__1 - r__3)) * q__23 * (r__2 ^ 3) + ((-0.6e1 * b__4 * b__5 * c__r4 + (8 * a__2 ^ 2) + (16 * b__1 ^ 2) - (32 * r__3 * b__1) + (8 * b__3 ^ 2) + 0.4e1 * b__4 ^ 2 - 0.8e1 * b__5 ^ 2 + (16 * r__3 ^ 2)) * (q__23 ^ 2) + (-0.12e2 * c__r5 ^ 2 - (6 * q__33 ^ 2)) * b__5 ^ 2 + 0.36e2 * q__33 * (-c__r4 * q__33 * b__4 / 0.3e1 + c__r5 * b__1 - c__r5 * r__3) * b__5 + 0.18e2 * (q__33 ^ 2) * ((a__2 ^ 2) - (b__1 ^ 2) + (2 * r__3 * b__1) + (b__3 ^ 2) - b__4 ^ 2 - (r__3 ^ 2))) * (r__2 ^ 2) + 0.8e1 * (-c__r5 * b__5 ^ 3 + ((q__33 * b__1) / 0.2e1 - (q__33 * r__3) / 0.2e1 - c__r4 * c__r5 * b__4) * b__5 ^ 2 + (0.2e1 * c__r5 * (b__1 ^ 2) + (-c__r4 * q__33 * b__4 - 0.4e1 * c__r5 * r__3) * b__1 + 0.2e1 * c__r5 * (r__3 ^ 2) + q__33 * b__4 * r__3 * c__r4 + c__r5 * (a__2 ^ 2 + b__3 ^ 2)) * b__5 + 0.3e1 / 0.2e1 * q__33 * ((a__2 ^ 2) - (b__1 ^ 2) + (2 * r__3 * b__1) + (b__3 ^ 2) - 0.7e1 / 0.3e1 * b__4 ^ 2 - (r__3 ^ 2)) * (b__1 - r__3)) * q__23 * r__2 - (b__5 ^ 4 + 0.2e1 * b__4 * c__r4 * b__5 ^ 3 + (-(2 * a__2 ^ 2) - (2 * b__1 ^ 2) + (4 * r__3 * b__1) - (2 * b__3 ^ 2) + 0.2e1 * b__4 ^ 2 - (2 * r__3 ^ 2)) * b__5 ^ 2 - 0.2e1 * b__4 * c__r4 * ((a__2 ^ 2) - (b__1 ^ 2) + (2 * r__3 * b__1) + (b__3 ^ 2) - b__4 ^ 2 - (r__3 ^ 2)) * b__5 + (b__1 ^ 4) - (4 * r__3 * b__1 ^ 3) + (-(2 * a__2 ^ 2) - (2 * b__3 ^ 2) + 0.6e1 * b__4 ^ 2 + (6 * r__3 ^ 2)) * (b__1 ^ 2) + 0.4e1 * r__3 * ((a__2 ^ 2) + (b__3 ^ 2) - 0.3e1 * b__4 ^ 2 - (r__3 ^ 2)) * b__1 + (r__3 ^ 4) + (-(2 * a__2 ^ 2) - (2 * b__3 ^ 2) + 0.6e1 * b__4 ^ 2) * (r__3 ^ 2) + ((a__2 ^ 2) + (b__3 ^ 2) - b__4 ^ 2) ^ 2) * (q__23 ^ 2)) * r__1 - 0.2e1 * q__13 * r__2 * (-(2 * r__2 ^ 4 * q__23) + (-0.4e1 * c__r5 * b__5 + (3 * q__33 * (b__1 - r__3))) * (r__2 ^ 3) + q__23 * ((a__2 ^ 2) - (b__1 ^ 2) + (2 * r__3 * b__1) + (b__3 ^ 2) - b__4 ^ 2 - b__5 ^ 2 - (r__3 ^ 2)) * (r__2 ^ 2) + (0.2e1 * c__r5 * b__5 ^ 3 + (0.2e1 * c__r4 * c__r5 * b__4 - (q__33 * b__1) + (q__33 * r__3)) * b__5 ^ 2 + (-0.4e1 * c__r5 * (b__1 ^ 2) + (0.2e1 * c__r4 * q__33 * b__4 + 0.8e1 * c__r5 * r__3) * b__1 - 0.4e1 * c__r5 * (r__3 ^ 2) - 0.2e1 * q__33 * b__4 * r__3 * c__r4 - 0.2e1 * c__r5 * (a__2 ^ 2 + b__3 ^ 2)) * b__5 - 0.3e1 * q__33 * ((a__2 ^ 2) - (b__1 ^ 2) + (2 * r__3 * b__1) + (b__3 ^ 2) - 0.7e1 / 0.3e1 * b__4 ^ 2 - (r__3 ^ 2)) * (b__1 - r__3)) * r__2 + (b__5 ^ 4 + 0.2e1 * b__4 * c__r4 * b__5 ^ 3 + (-(2 * a__2 ^ 2) - (2 * b__1 ^ 2) + (4 * r__3 * b__1) - (2 * b__3 ^ 2) + 0.2e1 * b__4 ^ 2 - (2 * r__3 ^ 2)) * b__5 ^ 2 - 0.2e1 * b__4 * c__r4 * ((a__2 ^ 2) - (b__1 ^ 2) + (2 * r__3 * b__1) + (b__3 ^ 2) - b__4 ^ 2 - (r__3 ^ 2)) * b__5 + (b__1 ^ 4) - (4 * r__3 * b__1 ^ 3) + (-(2 * a__2 ^ 2) - (2 * b__3 ^ 2) + 0.6e1 * b__4 ^ 2 + (6 * r__3 ^ 2)) * (b__1 ^ 2) + 0.4e1 * r__3 * ((a__2 ^ 2) + (b__3 ^ 2) - 0.3e1 * b__4 ^ 2 - (r__3 ^ 2)) * b__1 + (r__3 ^ 4) + (-(2 * a__2 ^ 2) - (2 * b__3 ^ 2) + 0.6e1 * b__4 ^ 2) * (r__3 ^ 2) + ((a__2 ^ 2) + (b__3 ^ 2) - b__4 ^ 2) ^ 2) * q__23)) * b__3 * ((c__r4 - 1) ^ 3) / s__r4 ^ 6 / b__5 ^ 2;

w__5 =((c__r4 + 1) ^ 3) * (((-q__13 ^ 2 + q__23 ^ 2) * b__5 ^ 6) + ((-4 * q__13 ^ 2 * b__4 * c__r4 + 4 * b__4 * c__r4 * q__23 ^ 2 - 4 * c__r5 * q__13 * r__1 + 4 * c__r5 * q__23 * r__2) * b__5 ^ 5) + (((-4 * c__r5 ^ 2 - q__13 ^ 2 - 4 * q__23 ^ 2 - q__33 ^ 2) * r__1 ^ 2) - 0.12e2 * q__13 * ((c__r4 * c__r5 * b__4) + (r__2 * q__23) / 0.3e1 - (q__33 * b__1) / 0.3e1 + (q__33 * r__3) / 0.3e1) * r__1 + ((4 * c__r5 ^ 2 + 2 * q__13 ^ 2 + 3 * q__23 ^ 2 + q__33 ^ 2) * r__2 ^ 2) + 0.12e2 * ((c__r4 * c__r5 * b__4) - (q__33 * b__1) / 0.3e1 + (q__33 * r__3) / 0.3e1) * q__23 * r__2 + 0.2e1 * ((b__1 ^ 2) - (2 * r__3 * b__1) + (r__3 ^ 2) + ((-2 * c__r4 ^ 2 - 1) * b__4 ^ 2) + a__2 ^ 2 + 0.3e1 / 0.2e1 * b__3 ^ 2) * (q__13 - q__23) * (q__13 + q__23)) * (b__5 ^ 4) + ((-(28 * c__r5 * q__23 * r__2) - (8 * b__4 * c__r4 * q__23 ^ 2) - (4 * q__13 ^ 2 * b__4 * c__r4) + (12 * c__r5 * q__33 * b__1) - (12 * c__r5 * q__33 * r__3) - 0.8e1 * b__4 * c__r4 * ((c__r5 ^ 2) + (q__33 ^ 2) / 0.2e1)) * (r__1 ^ 2) + 0.4e1 * q__13 * ((c__r5 * r__2 ^ 2) + (c__r5 * b__1 ^ 2) + ((c__r4 * q__33 * b__4 - 2 * c__r5 * r__3) * b__1) + (c__r5 * r__3 ^ 2) - (q__33 * b__4 * r__3 * c__r4) + (((-2 * c__r4 ^ 2 - 1) * b__4 ^ 2) + a__2 ^ 2 + 0.2e1 * b__3 ^ 2) * c__r5) * r__1 + (8 * c__r5 * q__23 * r__2 ^ 3) + ((4 * b__4 * c__r4 * q__23 ^ 2) + (8 * q__13 ^ 2 * b__4 * c__r4) - (12 * c__r5 * q__33 * b__1) + (12 * c__r5 * q__33 * r__3) + 0.8e1 * b__4 * c__r4 * ((c__r5 ^ 2) + (q__33 ^ 2) / 0.2e1)) * (r__2 ^ 2) - 0.4e1 * ((c__r5 * b__1 ^ 2) + ((c__r4 * q__33 * b__4 - 2 * c__r5 * r__3) * b__1) + (c__r5 * r__3 ^ 2) - (q__33 * b__4 * r__3 * c__r4) + (((-2 * c__r4 ^ 2 - 1) * b__4 ^ 2) + a__2 ^ 2 + 0.2e1 * b__3 ^ 2) * c__r5) * q__23 * r__2 + 0.4e1 * b__4 * c__r4 * (q__13 - q__23) * (q__13 + q__23) * (a__2 ^ 2 + (b__1 ^ 2) - (2 * r__3 * b__1) + 0.2e1 * b__3 ^ 2 - (b__4 ^ 2) + (r__3 ^ 2))) * (b__5 ^ 3) + (((4 * c__r5 ^ 2 + q__13 ^ 2 + 5 * q__23 ^ 2 + 2 * q__33 ^ 2) * r__1 ^ 4) - (4 * q__13 * (c__r4 * c__r5 * b__4 - q__33 * b__1 + 3 * r__2 * q__23 + q__33 * r__3) * r__1 ^ 3) + (((-24 * c__r5 ^ 2 - 4 * q__13 ^ 2 - 20 * q__23 ^ 2) * r__2 ^ 2) - 0.28e2 * ((c__r4 * c__r5 * b__4) - 0.8e1 / 0.7e1 * q__33 * b__1 + 0.8e1 / 0.7e1 * q__33 * r__3) * q__23 * r__2 + ((6 * b__1 ^ 2) - (12 * r__3 * b__1) + (6 * r__3 ^ 2) + ((-4 * c__r4 ^ 2 - 2) * b__4 ^ 2) + 0.6e1 * a__2 ^ 2 + 0.16e2 * b__3 ^ 2) * (q__23 ^ 2) + (-(4 * b__4 ^ 2 * c__r4 ^ 2) + 0.2e1 * b__3 ^ 2) * (q__13 ^ 2) + ((-4 * c__r5 ^ 2 - 6 * q__33 ^ 2) * b__1 ^ 2) + (((8 * c__r5 ^ 2 + 12 * q__33 ^ 2) * r__3 + 16 * c__r5 * q__33 * b__4 * c__r4) * b__1) + ((-4 * c__r5 ^ 2 - 6 * q__33 ^ 2) * r__3 ^ 2) - (16 * c__r5 * q__33 * b__4 * r__3 * c__r4) + ((-4 * c__r5 ^ 2 - 6 * q__33 ^ 2) * b__4 ^ 2) + (0.6e1 * a__2 ^ 2 + 0.14e2 * b__3 ^ 2) * (q__33 ^ 2) + 0.4e1 * (c__r5 ^ 2) * b__3 ^ 2) * (r__1 ^ 2) + 0.4e1 * q__13 * ((3 * r__2 ^ 3 * q__23) + ((7 * c__r4 * c__r5 * b__4 - 2 * q__33 * b__1 + 2 * q__33 * r__3) * r__2 ^ 2) + 0.2e1 * q__23 * (a__2 ^ 2 + (b__1 ^ 2) - (2 * r__3 * b__1) + b__3 ^ 2 + (b__4 ^ 2) + (r__3 ^ 2)) * r__2 - (b__1 ^ 3 * q__33) + ((3 * c__r4 * c__r5 * b__4 + 3 * q__33 * r__3) * b__1 ^ 2) + (-(3 * q__33 * r__3 ^ 2) - (6 * c__r5 * b__4 * c__r4 * r__3) + q__33 * (((2 * c__r4 ^ 2 - 3) * b__4 ^ 2) + a__2 ^ 2 + 0.2e1 * b__3 ^ 2)) * b__1 + (q__33 * r__3 ^ 3) + (3 * c__r5 * b__4 * c__r4 * r__3 ^ 2) - q__33 * (((2 * c__r4 ^ 2 - 3) * b__4 ^ 2) + a__2 ^ 2 + 0.2e1 * b__3 ^ 2) * r__3 + c__r5 * b__4 * c__r4 * (a__2 ^ 2 + 0.3e1 * b__3 ^ 2 - (b__4 ^ 2))) * r__1 + ((4 * c__r5 ^ 2 - q__13 ^ 2 + 3 * q__23 ^ 2 - 2 * q__33 ^ 2) * r__2 ^ 4) + (4 * q__23 * (c__r4 * c__r5 * b__4 - 3 * q__33 * b__1 + 3 * q__33 * r__3) * r__2 ^ 3) + ((-(4 * b__1 ^ 2) + (8 * r__3 * b__1) - (4 * r__3 ^ 2) + ((4 * c__r4 ^ 2 - 4) * b__4 ^ 2) - 0.4e1 * a__2 ^ 2 - 0.6e1 * b__3 ^ 2) * (q__23 ^ 2) + (-(2 * b__1 ^ 2) + (4 * r__3 * b__1) - (2 * r__3 ^ 2) + ((4 * c__r4 ^ 2 + 6) * b__4 ^ 2) - 0.2e1 * a__2 ^ 2 - 0.12e2 * b__3 ^ 2) * (q__13 ^ 2) + ((4 * c__r5 ^ 2 + 6 * q__33 ^ 2) * b__1 ^ 2) + (((-8 * c__r5 ^ 2 - 12 * q__33 ^ 2) * r__3 - 16 * c__r5 * q__33 * b__4 * c__r4) * b__1) + ((4 * c__r5 ^ 2 + 6 * q__33 ^ 2) * r__3 ^ 2) + (16 * c__r5 * q__33 * b__4 * r__3 * c__r4) + ((4 * c__r5 ^ 2 + 6 * q__33 ^ 2) * b__4 ^ 2) + (-0.6e1 * a__2 ^ 2 - 0.14e2 * b__3 ^ 2) * (q__33 ^ 2) - 0.4e1 * (c__r5 ^ 2) * b__3 ^ 2) * (r__2 ^ 2) - 0.4e1 * (-(b__1 ^ 3 * q__33) + ((3 * c__r4 * c__r5 * b__4 + 3 * q__33 * r__3) * b__1 ^ 2) + (-(3 * q__33 * r__3 ^ 2) - (6 * c__r5 * b__4 * c__r4 * r__3) + q__33 * (((2 * c__r4 ^ 2 - 3) * b__4 ^ 2) + a__2 ^ 2 + 0.2e1 * b__3 ^ 2)) * b__1 + (q__33 * r__3 ^ 3) + (3 * c__r5 * b__4 * c__r4 * r__3 ^ 2) - q__33 * (((2 * c__r4 ^ 2 - 3) * b__4 ^ 2) + a__2 ^ 2 + 0.2e1 * b__3 ^ 2) * r__3 + c__r5 * b__4 * c__r4 * (a__2 ^ 2 + 0.3e1 * b__3 ^ 2 - (b__4 ^ 2))) * q__23 * r__2 - ((b__1 ^ 4) - (4 * r__3 * b__1 ^ 3) + ((6 * r__3 ^ 2) + ((-4 * c__r4 ^ 2 + 2) * b__4 ^ 2) - 0.2e1 * a__2 ^ 2) * (b__1 ^ 2) + 0.4e1 * r__3 * (-(r__3 ^ 2) + ((2 * c__r4 ^ 2 - 1) * b__4 ^ 2) + a__2 ^ 2) * b__1 + (r__3 ^ 4) + (((-4 * c__r4 ^ 2 + 2) * b__4 ^ 2) - 0.2e1 * a__2 ^ 2) * (r__3 ^ 2) + (b__4 ^ 4) + ((-4 * c__r4 ^ 2 - 4) * b__3 ^ 2 - 0.2e1 * a__2 ^ 2) * (b__4 ^ 2) + a__2 ^ 4 + 0.4e1 * a__2 ^ 2 * b__3 ^ 2 + 0.3e1 * b__3 ^ 4) * (q__13 - q__23) * (q__13 + q__23)) * (b__5 ^ 2) + ((4 * c__r5 * q__13 * r__1 ^ 5) + ((24 * c__r5 * q__23 * r__2) + (4 * b__4 * c__r4 * q__23 ^ 2) - 0.12e2 * q__33 * (-(c__r4 * q__33 * b__4) / 0.3e1 + (c__r5 * b__1) - (c__r5 * r__3))) * (r__1 ^ 4) - 0.4e1 * q__13 * ((11 * c__r5 * r__2 ^ 2) + (4 * q__23 * b__4 * c__r4 * r__2) + (3 * c__r5 * b__1 ^ 2) + ((-3 * c__r4 * q__33 * b__4 - 6 * c__r5 * r__3) * b__1) + (3 * c__r5 * r__3 ^ 2) + (3 * q__33 * b__4 * r__3 * c__r4) + c__r5 * (a__2 ^ 2 + (b__4 ^ 2))) * (r__1 ^ 3) + (-(36 * c__r5 * q__23 * r__2 ^ 3) + ((-12 * b__4 * c__r4 * q__23 ^ 2 + 12 * q__13 ^ 2 * b__4 * c__r4 + 48 * c__r5 * q__33 * (b__1 - r__3)) * r__2 ^ 2) + 0.16e2 * ((c__r5 * b__1 ^ 2) / 0.2e1 + (0.5e1 / 0.4e1 * c__r4 * q__33 * b__4 - (c__r5 * r__3)) * b__1 + (c__r5 * r__3 ^ 2) / 0.2e1 - 0.5e1 / 0.4e1 * q__33 * b__4 * r__3 * c__r4 + c__r5 * (a__2 ^ 2 + 0.15e2 / 0.4e1 * b__3 ^ 2)) * q__23 * r__2 + 0.4e1 * b__4 * c__r4 * (a__2 ^ 2 + (b__1 ^ 2) - (2 * r__3 * b__1) + 0.4e1 * b__3 ^ 2 - (b__4 ^ 2) + (r__3 ^ 2)) * (q__23 ^ 2) + 0.8e1 * ((b__1 ^ 2) - (2 * r__3 * b__1) + b__3 ^ 2 / 0.2e1 + (r__3 ^ 2)) * b__4 * c__r4 * (q__13 ^ 2) - 0.4e1 * (-(c__r5 * b__1 ^ 3) + ((c__r4 * q__33 * b__4 + 3 * c__r5 * r__3) * b__1 ^ 2) + (-(3 * c__r5 * r__3 ^ 2) - (2 * q__33 * b__4 * r__3 * c__r4) + c__r5 * (a__2 ^ 2 + 0.7e1 * b__3 ^ 2 - (b__4 ^ 2))) * b__1 + (c__r5 * r__3 ^ 3) + (q__33 * b__4 * c__r4 * r__3 ^ 2) - c__r5 * (a__2 ^ 2 + 0.7e1 * b__3 ^ 2 - (b__4 ^ 2)) * r__3 - q__33 * b__4 * c__r4 * (a__2 ^ 2 + 0.5e1 * b__3 ^ 2 - (b__4 ^ 2))) * q__33) * (r__1 ^ 2) - 0.4e1 * q__13 * (-(4 * c__r5 * r__2 ^ 4) - (4 * q__23 * b__4 * c__r4 * r__2 ^ 3) + (-(4 * c__r5 * b__1 ^ 2) + ((5 * c__r4 * q__33 * b__4 + 8 * c__r5 * r__3) * b__1) - (4 * c__r5 * r__3 ^ 2) - (5 * q__33 * b__4 * r__3 * c__r4) - 0.2e1 * (a__2 ^ 2 - 0.9e1 / 0.2e1 * b__3 ^ 2 + (3 * b__4 ^ 2)) * c__r5) * (r__2 ^ 2) + (q__33 * b__4 * c__r4 * b__1 ^ 3) + (-(3 * q__33 * b__4 * r__3 * c__r4) + 0.5e1 * b__3 ^ 2 * c__r5 - (2 * b__4 ^ 2 * c__r5)) * (b__1 ^ 2) + ((3 * q__33 * b__4 * c__r4 * r__3 ^ 2) + (-0.10e2 * b__3 ^ 2 * c__r5 + (4 * b__4 ^ 2 * c__r5)) * r__3 - q__33 * b__4 * c__r4 * (a__2 ^ 2 + 0.5e1 * b__3 ^ 2 - (b__4 ^ 2))) * b__1 - (q__33 * b__4 * c__r4 * r__3 ^ 3) + (0.5e1 * b__3 ^ 2 * c__r5 - (2 * b__4 ^ 2 * c__r5)) * (r__3 ^ 2) + q__33 * b__4 * c__r4 * (a__2 ^ 2 + 0.5e1 * b__3 ^ 2 - (b__4 ^ 2)) * r__3 + c__r5 * b__3 ^ 2 * (a__2 ^ 2 + b__3 ^ 2 - (b__4 ^ 2))) * r__1 + (4 * c__r5 * q__23 * r__2 ^ 5) + ((-4 * q__13 ^ 2 * b__4 * c__r4 - 4 * q__33 * (c__r4 * q__33 * b__4 + c__r5 * b__1 - c__r5 * r__3)) * r__2 ^ 4) - 0.4e1 * (-(c__r5 * b__1 ^ 2) + ((3 * c__r4 * q__33 * b__4 + 2 * c__r5 * r__3) * b__1) - (c__r5 * r__3 ^ 2) - (3 * q__33 * b__4 * r__3 * c__r4) + c__r5 * (a__2 ^ 2 + 0.2e1 * b__3 ^ 2 + (b__4 ^ 2))) * q__23 * (r__2 ^ 3) + (-0.8e1 * ((b__1 ^ 2) - (2 * r__3 * b__1) + b__3 ^ 2 / 0.2e1 + (r__3 ^ 2)) * b__4 * c__r4 * (q__23 ^ 2) - 0.4e1 * b__4 * c__r4 * (a__2 ^ 2 + (b__1 ^ 2) - (2 * r__3 * b__1) + 0.4e1 * b__3 ^ 2 - (b__4 ^ 2) + (r__3 ^ 2)) * (q__13 ^ 2) + 0.4e1 * (-(c__r5 * b__1 ^ 3) + ((c__r4 * q__33 * b__4 + 3 * c__r5 * r__3) * b__1 ^ 2) + (-(3 * c__r5 * r__3 ^ 2) - (2 * q__33 * b__4 * r__3 * c__r4) + c__r5 * (a__2 ^ 2 + 0.7e1 * b__3 ^ 2 - (b__4 ^ 2))) * b__1 + (c__r5 * r__3 ^ 3) + (q__33 * b__4 * c__r4 * r__3 ^ 2) - c__r5 * (a__2 ^ 2 + 0.7e1 * b__3 ^ 2 - (b__4 ^ 2)) * r__3 - q__33 * b__4 * c__r4 * (a__2 ^ 2 + 0.5e1 * b__3 ^ 2 - (b__4 ^ 2))) * q__33) * (r__2 ^ 2) + 0.4e1 * ((q__33 * b__4 * c__r4 * b__1 ^ 3) + (-(3 * q__33 * b__4 * r__3 * c__r4) + 0.5e1 * b__3 ^ 2 * c__r5 - (2 * b__4 ^ 2 * c__r5)) * (b__1 ^ 2) + ((3 * q__33 * b__4 * c__r4 * r__3 ^ 2) + (-0.10e2 * b__3 ^ 2 * c__r5 + (4 * b__4 ^ 2 * c__r5)) * r__3 - q__33 * b__4 * c__r4 * (a__2 ^ 2 + 0.5e1 * b__3 ^ 2 - (b__4 ^ 2))) * b__1 - (q__33 * b__4 * c__r4 * r__3 ^ 3) + (0.5e1 * b__3 ^ 2 * c__r5 - (2 * b__4 ^ 2 * c__r5)) * (r__3 ^ 2) + q__33 * b__4 * c__r4 * (a__2 ^ 2 + 0.5e1 * b__3 ^ 2 - (b__4 ^ 2)) * r__3 + c__r5 * b__3 ^ 2 * (a__2 ^ 2 + b__3 ^ 2 - (b__4 ^ 2))) * q__23 * r__2 - 0.4e1 * b__3 ^ 2 * b__4 * c__r4 * (q__13 - q__23) * (q__13 + q__23) * (a__2 ^ 2 - (b__1 ^ 2) + (2 * r__3 * b__1) + b__3 ^ 2 - (b__4 ^ 2) - (r__3 ^ 2))) * b__5 + ((q__13 ^ 2 - 2 * q__23 ^ 2 - q__33 ^ 2) * r__1 ^ 6) + 0.16e2 * q__13 * ((r__2 * q__23) - (q__33 * (b__1 - r__3)) / 0.2e1) * (r__1 ^ 5) + (((-18 * q__13 ^ 2 + 17 * q__23 ^ 2 - q__33 ^ 2) * r__2 ^ 2) - (28 * q__23 * q__33 * (b__1 - r__3) * r__2) + (-0.4e1 * a__2 ^ 2 - (4 * b__1 ^ 2) + (8 * r__3 * b__1) - 0.17e2 * b__3 ^ 2 - (4 * r__3 ^ 2)) * (q__23 ^ 2) + (-0.2e1 * a__2 ^ 2 - (6 * b__1 ^ 2) + (12 * r__3 * b__1) - b__3 ^ 2 - (2 * b__4 ^ 2) - (6 * r__3 ^ 2)) * (q__13 ^ 2) - 0.6e1 * (q__33 ^ 2) * (a__2 ^ 2 - (b__1 ^ 2) + (2 * r__3 * b__1) + 0.3e1 * b__3 ^ 2 - (b__4 ^ 2) - (r__3 ^ 2))) * (r__1 ^ 4) + 0.4e1 * (-(10 * r__2 ^ 3 * q__23) + (11 * q__33 * (b__1 - r__3) * r__2 ^ 2) + q__23 * (a__2 ^ 2 - (b__1 ^ 2) + (2 * r__3 * b__1) + 0.13e2 * b__3 ^ 2 - (b__4 ^ 2) - (r__3 ^ 2)) * r__2 - 0.2e1 * q__33 * (a__2 ^ 2 - (b__1 ^ 2) + (2 * r__3 * b__1) + 0.11e2 / 0.2e1 * b__3 ^ 2 - (2 * b__4 ^ 2) - (r__3 ^ 2)) * (b__1 - r__3)) * q__13 * (r__1 ^ 3) + (((13 * q__13 ^ 2 - 12 * q__23 ^ 2 + q__33 ^ 2) * r__2 ^ 4) + (36 * q__23 * q__33 * (b__1 - r__3) * r__2 ^ 3) + ((0.14e2 * a__2 ^ 2 + (10 * b__1 ^ 2) - (20 * r__3 * b__1) + 0.48e2 * b__3 ^ 2 + (10 * b__4 ^ 2) + (10 * r__3 ^ 2)) * (q__23 ^ 2) + (0.10e2 * a__2 ^ 2 + (14 * b__1 ^ 2) - (28 * r__3 * b__1) - 0.24e2 * b__3 ^ 2 + (14 * b__4 ^ 2) + (14 * r__3 ^ 2)) * (q__13 ^ 2) + 0.24e2 * (q__33 ^ 2) * (a__2 ^ 2 - (b__1 ^ 2) + (2 * r__3 * b__1) + b__3 ^ 2 - (b__4 ^ 2) - (r__3 ^ 2))) * (r__2 ^ 2) + 0.12e2 * q__33 * (a__2 ^ 2 - (b__1 ^ 2) + (2 * r__3 * b__1) - 0.4e1 * b__3 ^ 2 - 0.11e2 / 0.3e1 * (b__4 ^ 2) - (r__3 ^ 2)) * (b__1 - r__3) * q__23 * r__2 + (-(2 * b__1 ^ 4) + (8 * r__3 * b__1 ^ 3) + (0.4e1 * a__2 ^ 2 - 0.10e2 * b__3 ^ 2 - (8 * b__4 ^ 2) - (12 * r__3 ^ 2)) * (b__1 ^ 2) - 0.8e1 * r__3 * (a__2 ^ 2 - 0.5e1 / 0.2e1 * b__3 ^ 2 - (2 * b__4 ^ 2) - (r__3 ^ 2)) * b__1 - (2 * r__3 ^ 4) + (0.4e1 * a__2 ^ 2 - 0.10e2 * b__3 ^ 2 - (8 * b__4 ^ 2)) * (r__3 ^ 2) - (2 * b__4 ^ 4) + (0.4e1 * a__2 ^ 2 + 0.10e2 * b__3 ^ 2) * (b__4 ^ 2) - 0.2e1 * a__2 ^ 4 - 0.14e2 * a__2 ^ 2 * b__3 ^ 2 - 0.12e2 * b__3 ^ 4) * (q__23 ^ 2) + ((b__1 ^ 4) - (4 * r__3 * b__1 ^ 3) + (-0.2e1 * a__2 ^ 2 - 0.24e2 * b__3 ^ 2 + (10 * b__4 ^ 2) + (6 * r__3 ^ 2)) * (b__1 ^ 2) + 0.4e1 * r__3 * (a__2 ^ 2 + 0.12e2 * b__3 ^ 2 - (5 * b__4 ^ 2) - (r__3 ^ 2)) * b__1 + (r__3 ^ 4) + (-0.2e1 * a__2 ^ 2 - 0.24e2 * b__3 ^ 2 + (10 * b__4 ^ 2)) * (r__3 ^ 2) + (b__4 ^ 4) + (-0.2e1 * a__2 ^ 2 - 0.4e1 * b__3 ^ 2) * (b__4 ^ 2) + a__2 ^ 4 - b__3 ^ 4) * (q__13 ^ 2) - (q__33 ^ 2) * ((b__1 ^ 4) - (4 * r__3 * b__1 ^ 3) + (-0.2e1 * a__2 ^ 2 - 0.14e2 * b__3 ^ 2 - (2 * b__4 ^ 2) + (6 * r__3 ^ 2)) * (b__1 ^ 2) + 0.4e1 * r__3 * (a__2 ^ 2 + 0.7e1 * b__3 ^ 2 + (b__4 ^ 2) - (r__3 ^ 2)) * b__1 + (r__3 ^ 4) + (-0.2e1 * a__2 ^ 2 - 0.14e2 * b__3 ^ 2 - (2 * b__4 ^ 2)) * (r__3 ^ 2) + (a__2 ^ 2 + 0.13e2 * b__3 ^ 2 - (b__4 ^ 2)) * (a__2 ^ 2 + b__3 ^ 2 - (b__4 ^ 2)))) * (r__1 ^ 2) - 0.4e1 * q__13 * (-(2 * q__23 * r__2 ^ 5) + (3 * q__33 * (b__1 - r__3) * r__2 ^ 4) + q__23 * (a__2 ^ 2 - (b__1 ^ 2) + (2 * r__3 * b__1) + 0.13e2 * b__3 ^ 2 - (b__4 ^ 2) - (r__3 ^ 2)) * (r__2 ^ 3) - 0.3e1 * q__33 * (a__2 ^ 2 - (b__1 ^ 2) + (2 * r__3 * b__1) + 0.6e1 * b__3 ^ 2 - 0.7e1 / 0.3e1 * (b__4 ^ 2) - (r__3 ^ 2)) * (b__1 - r__3) * (r__2 ^ 2) + q__23 * ((b__1 ^ 4) - (4 * r__3 * b__1 ^ 3) + (-0.2e1 * a__2 ^ 2 - 0.2e1 * b__3 ^ 2 + (6 * b__4 ^ 2) + (6 * r__3 ^ 2)) * (b__1 ^ 2) + 0.4e1 * r__3 * (a__2 ^ 2 + b__3 ^ 2 - (3 * b__4 ^ 2) - (r__3 ^ 2)) * b__1 + (r__3 ^ 4) + (-0.2e1 * a__2 ^ 2 - 0.2e1 * b__3 ^ 2 + (6 * b__4 ^ 2)) * (r__3 ^ 2) + (a__2 ^ 2 + b__3 ^ 2 - (b__4 ^ 2)) ^ 2) * r__2 + 0.3e1 * q__33 * (a__2 ^ 2 - (b__1 ^ 2) + (2 * r__3 * b__1) + b__3 ^ 2 - 0.5e1 / 0.3e1 * (b__4 ^ 2) - (r__3 ^ 2)) * (b__1 - r__3) * b__3 ^ 2) * r__1 + ((q__23 ^ 2 + q__33 ^ 2) * r__2 ^ 6) + ((-0.2e1 * a__2 ^ 2 + (2 * b__1 ^ 2) - (4 * r__3 * b__1) - 0.3e1 * b__3 ^ 2 - (2 * b__4 ^ 2) + (2 * r__3 ^ 2)) * (q__23 ^ 2) + (0.13e2 * b__3 ^ 2 - (4 * b__4 ^ 2)) * (q__13 ^ 2) - 0.2e1 * (q__33 ^ 2) * (a__2 ^ 2 - (b__1 ^ 2) + (2 * r__3 * b__1) - 0.5e1 * b__3 ^ 2 - (b__4 ^ 2) - (r__3 ^ 2))) * (r__2 ^ 4) + 0.36e2 * (b__3 ^ 2 + 0.2e1 / 0.9e1 * (b__4 ^ 2)) * q__33 * (b__1 - r__3) * q__23 * (r__2 ^ 3) + (((b__1 ^ 4) - (4 * r__3 * b__1 ^ 3) + (-0.2e1 * a__2 ^ 2 + 0.20e2 * b__3 ^ 2 + (2 * b__4 ^ 2) + (6 * r__3 ^ 2)) * (b__1 ^ 2) + 0.4e1 * r__3 * (a__2 ^ 2 - 0.10e2 * b__3 ^ 2 - (b__4 ^ 2) - (r__3 ^ 2)) * b__1 + (r__3 ^ 4) + (-0.2e1 * a__2 ^ 2 + 0.20e2 * b__3 ^ 2 + (2 * b__4 ^ 2)) * (r__3 ^ 2) + a__2 ^ 4 + 0.4e1 * a__2 ^ 2 * b__3 ^ 2 - 0.2e1 * a__2 ^ 2 * (b__4 ^ 2) + 0.3e1 * b__3 ^ 4 + (b__4 ^ 4)) * (q__23 ^ 2) + ((0.14e2 * b__3 ^ 2 - (4 * b__4 ^ 2)) * (b__1 ^ 2) + (-0.28e2 * b__3 ^ 2 + (8 * b__4 ^ 2)) * r__3 * b__1 + (0.14e2 * b__3 ^ 2 - (4 * b__4 ^ 2)) * (r__3 ^ 2) + 0.10e2 * a__2 ^ 2 * b__3 ^ 2 + 0.10e2 * b__3 ^ 4 - 0.6e1 * b__3 ^ 2 * (b__4 ^ 2)) * (q__13 ^ 2) + (q__33 ^ 2) * ((b__1 ^ 4) - (4 * r__3 * b__1 ^ 3) + (-0.2e1 * a__2 ^ 2 - 0.14e2 * b__3 ^ 2 - (2 * b__4 ^ 2) + (6 * r__3 ^ 2)) * (b__1 ^ 2) + 0.4e1 * r__3 * (a__2 ^ 2 + 0.7e1 * b__3 ^ 2 + (b__4 ^ 2) - (r__3 ^ 2)) * b__1 + (r__3 ^ 4) + (-0.2e1 * a__2 ^ 2 - 0.14e2 * b__3 ^ 2 - (2 * b__4 ^ 2)) * (r__3 ^ 2) + (a__2 ^ 2 + 0.13e2 * b__3 ^ 2 - (b__4 ^ 2)) * (a__2 ^ 2 + b__3 ^ 2 - (b__4 ^ 2)))) * (r__2 ^ 2) + 0.12e2 * q__33 * (a__2 ^ 2 - (b__1 ^ 2) + (2 * r__3 * b__1) + b__3 ^ 2 - 0.5e1 / 0.3e1 * (b__4 ^ 2) - (r__3 ^ 2)) * (b__1 - r__3) * b__3 ^ 2 * q__23 * r__2 + (q__13 - q__23) * b__3 ^ 2 * ((b__1 ^ 4) - (4 * r__3 * b__1 ^ 3) + (-0.2e1 * a__2 ^ 2 - 0.2e1 * b__3 ^ 2 + (6 * b__4 ^ 2) + (6 * r__3 ^ 2)) * (b__1 ^ 2) + 0.4e1 * r__3 * (a__2 ^ 2 + b__3 ^ 2 - (3 * b__4 ^ 2) - (r__3 ^ 2)) * b__1 + (r__3 ^ 4) + (-0.2e1 * a__2 ^ 2 - 0.2e1 * b__3 ^ 2 + (6 * b__4 ^ 2)) * (r__3 ^ 2) + (a__2 ^ 2 + b__3 ^ 2 - (b__4 ^ 2)) ^ 2) * (q__13 + q__23)) * ((c__r4 - 1) ^ 3) / s__r4 ^ 6 / (b__5 ^ 2);

w__6 =0.2e1 * ((c__r4 + 1) ^ 3) * (-(q__13 * q__23 * r__1 ^ 6) + (((2 * q__13 ^ 2 - 3 * q__23 ^ 2 - q__33 ^ 2) * r__2 - 2 * (c__r5 * b__5 - q__33 * (b__1 - r__3)) * q__23) * r__1 ^ 5) + 0.6e1 * q__13 * (0.5e1 / 0.3e1 * q__23 * (r__2 ^ 2) + ((c__r5 * b__5) - 0.5e1 / 0.3e1 * q__33 * (b__1 - r__3)) * r__2 - 0.5e1 / 0.6e1 * (-0.2e1 / 0.5e1 * b__4 * b__5 * c__r4 + b__3 ^ 2 - (b__5 ^ 2) / 0.5e1) * q__23) * (r__1 ^ 4) + (((-6 * q__13 ^ 2 + 4 * q__23 ^ 2 - 2 * q__33 ^ 2) * r__2 ^ 3) + 0.10e2 * q__23 * ((c__r5 * b__5) - 0.7e1 / 0.5e1 * q__33 * (b__1 - r__3)) * (r__2 ^ 2) + (((4 * c__r5 ^ 2 + 6 * q__23 ^ 2 + 2 * q__33 ^ 2) * b__5 ^ 2) + ((6 * b__4 * c__r4 * q__23 ^ 2) - (2 * q__13 ^ 2 * b__4 * c__r4) - 0.12e2 * q__33 * (-(c__r4 * q__33 * b__4) / 0.3e1 + (c__r5 * (b__1 - r__3)))) * b__5 + (-(4 * a__2 ^ 2) - (4 * b__1 ^ 2) + (8 * r__3 * b__1) - 0.22e2 * b__3 ^ 2 - (4 * r__3 ^ 2)) * (q__23 ^ 2) + (-(2 * a__2 ^ 2) - (6 * b__1 ^ 2) + (12 * r__3 * b__1) + 0.4e1 * b__3 ^ 2 - (2 * b__4 ^ 2) - (6 * r__3 ^ 2)) * (q__13 ^ 2) - 0.6e1 * (q__33 ^ 2) * ((a__2 ^ 2) - (b__1 ^ 2) + (2 * r__3 * b__1) + 0.3e1 * b__3 ^ 2 - (b__4 ^ 2) - (r__3 ^ 2))) * r__2 - 0.2e1 * (-(2 * c__r5 * b__5 ^ 3) + ((-3 * c__r4 * c__r5 * b__4 + 2 * q__33 * (b__1 - r__3)) * b__5 ^ 2) + (-(b__4 ^ 2 * c__r5) + (q__33 * c__r4 * (b__1 - r__3) * b__4) + c__r5 * ((a__2 ^ 2) + (b__1 ^ 2) - (2 * r__3 * b__1) + 0.6e1 * b__3 ^ 2 + (r__3 ^ 2))) * b__5 + q__33 * (b__1 - r__3) * ((a__2 ^ 2) - (b__1 ^ 2) + (2 * r__3 * b__1) - 0.2e1 * b__3 ^ 2 - (3 * b__4 ^ 2) - (r__3 ^ 2))) * q__23) * (r__1 ^ 3) + q__13 * (-(5 * r__2 ^ 4 * q__23) + ((-10 * c__r5 * b__5 + 6 * q__33 * (b__1 - r__3)) * r__2 ^ 3) + 0.4e1 * (-(3 * b__4 * b__5 * c__r4) + (a__2 ^ 2) - (b__1 ^ 2) + (2 * r__3 * b__1) + 0.21e2 / 0.2e1 * b__3 ^ 2 - (b__4 ^ 2) - 0.5e1 / 0.2e1 * (b__5 ^ 2) - (r__3 ^ 2)) * q__23 * (r__2 ^ 2) + (-(4 * c__r5 * b__5 ^ 3) + ((-10 * c__r4 * c__r5 * b__4 + 8 * q__33 * (b__1 - r__3)) * b__5 ^ 2) + (-(6 * b__4 ^ 2 * c__r5) + (14 * q__33 * c__r4 * (b__1 - r__3) * b__4) - 0.2e1 * c__r5 * ((a__2 ^ 2) + (5 * b__1 ^ 2) - (10 * r__3 * b__1) - 0.6e1 * b__3 ^ 2 + (5 * r__3 ^ 2))) * b__5 - 0.6e1 * q__33 * ((a__2 ^ 2) - (b__1 ^ 2) + (2 * r__3 * b__1) + 0.8e1 * b__3 ^ 2 - 0.5e1 / 0.3e1 * (b__4 ^ 2) - (r__3 ^ 2)) * (b__1 - r__3)) * r__2 + ((b__5 ^ 4) + (2 * b__4 * c__r4 * b__5 ^ 3) + (-(2 * a__2 ^ 2) - (2 * b__1 ^ 2) + (4 * r__3 * b__1) - 0.6e1 * b__3 ^ 2 + (2 * b__4 ^ 2) - (2 * r__3 ^ 2)) * (b__5 ^ 2) - 0.2e1 * b__4 * c__r4 * ((a__2 ^ 2) - (b__1 ^ 2) + (2 * r__3 * b__1) + 0.3e1 * b__3 ^ 2 - (b__4 ^ 2) - (r__3 ^ 2)) * b__5 + (b__4 ^ 4) + (-(2 * a__2 ^ 2) + (6 * b__1 ^ 2) - (12 * r__3 * b__1) - 0.6e1 * b__3 ^ 2 + (6 * r__3 ^ 2)) * (b__4 ^ 2) + ((a__2 ^ 2) - (b__1 ^ 2) + (2 * r__3 * b__1) + 0.5e1 * b__3 ^ 2 - (r__3 ^ 2)) * ((a__2 ^ 2) - (b__1 ^ 2) + (2 * r__3 * b__1) + b__3 ^ 2 - (r__3 ^ 2))) * q__23) * (r__1 ^ 2) + (((-q__23 ^ 2 - q__33 ^ 2) * r__2 ^ 5) - (4 * b__5 * c__r5 * q__23 * r__2 ^ 4) + (((-4 * c__r5 ^ 2 + 2 * q__13 ^ 2 - 4 * q__23 ^ 2 + 2 * q__33 ^ 2) * b__5 ^ 2) + ((-2 * b__4 * c__r4 * q__23 ^ 2 + 6 * q__13 ^ 2 * b__4 * c__r4 + 4 * q__33 * (c__r4 * q__33 * b__4 + c__r5 * (b__1 - r__3))) * b__5) + ((2 * a__2 ^ 2) - (2 * b__1 ^ 2) + (4 * r__3 * b__1) + 0.8e1 * b__3 ^ 2 + (2 * b__4 ^ 2) - (2 * r__3 ^ 2)) * (q__23 ^ 2) + (-0.18e2 * b__3 ^ 2 + (4 * b__4 ^ 2)) * (q__13 ^ 2) + 0.2e1 * (q__33 ^ 2) * ((a__2 ^ 2) - (b__1 ^ 2) + (2 * r__3 * b__1) - 0.5e1 * b__3 ^ 2 - (b__4 ^ 2) - (r__3 ^ 2))) * (r__2 ^ 3) + 0.4e1 * (-0.5e1 / 0.2e1 * c__r5 * (b__5 ^ 3) + (-0.5e1 / 0.2e1 * c__r4 * c__r5 * b__4 + 0.7e1 / 0.2e1 * q__33 * (b__1 - r__3)) * (b__5 ^ 2) + (0.7e1 / 0.2e1 * q__33 * c__r4 * (b__1 - r__3) * b__4 + c__r5 * ((a__2 ^ 2) - (b__1 ^ 2) + (2 * r__3 * b__1) + 0.9e1 / 0.2e1 * b__3 ^ 2 - (r__3 ^ 2))) * b__5 - 0.21e2 / 0.2e1 * (b__3 ^ 2 + 0.4e1 / 0.21e2 * (b__4 ^ 2)) * q__33 * (b__1 - r__3)) * q__23 * (r__2 ^ 2) + (((-4 * c__r5 ^ 2 - 2 * q__13 ^ 2 - 3 * q__23 ^ 2 - q__33 ^ 2) * b__5 ^ 4) + ((-6 * b__4 * c__r4 * q__23 ^ 2 - 6 * q__13 ^ 2 * b__4 * c__r4 + (-8 * c__r4 * c__r5 ^ 2 - 4 * c__r4 * q__33 ^ 2) * b__4 + 12 * c__r5 * q__33 * (b__1 - r__3)) * b__5 ^ 3) + ((-(4 * b__4 ^ 2 * c__r4 ^ 2) + (4 * a__2 ^ 2) + (4 * b__1 ^ 2) - (8 * r__3 * b__1) + 0.10e2 * b__3 ^ 2 + (4 * r__3 ^ 2)) * (q__23 ^ 2) + (((-4 * c__r4 ^ 2 - 2) * b__4 ^ 2) + (2 * a__2 ^ 2) + (2 * b__1 ^ 2) - (4 * r__3 * b__1) + 0.8e1 * b__3 ^ 2 + (2 * r__3 ^ 2)) * (q__13 ^ 2) + ((-4 * c__r5 ^ 2 - 6 * q__33 ^ 2) * b__4 ^ 2) + (16 * c__r5 * q__33 * c__r4 * (b__1 - r__3) * b__4) + ((-4 * c__r5 ^ 2 - 6 * q__33 ^ 2) * b__1 ^ 2) + ((8 * c__r5 ^ 2 + 12 * q__33 ^ 2) * r__3 * b__1) + ((-4 * c__r5 ^ 2 - 6 * q__33 ^ 2) * r__3 ^ 2) + ((6 * a__2 ^ 2) + 0.14e2 * b__3 ^ 2) * (q__33 ^ 2) + 0.4e1 * (c__r5 ^ 2) * b__3 ^ 2) * (b__5 ^ 2) + (0.2e1 * b__4 * c__r4 * ((a__2 ^ 2) + (3 * b__1 ^ 2) - (6 * r__3 * b__1) + 0.5e1 * b__3 ^ 2 - (b__4 ^ 2) + (3 * r__3 ^ 2)) * (q__23 ^ 2) + 0.2e1 * b__4 * c__r4 * ((a__2 ^ 2) + (3 * b__1 ^ 2) - (6 * r__3 * b__1) + 0.5e1 * b__3 ^ 2 - (b__4 ^ 2) + (3 * r__3 ^ 2)) * (q__13 ^ 2) - 0.4e1 * ((q__33 * c__r4 * b__4 ^ 3) - (c__r5 * b__4 ^ 2 * (b__1 - r__3)) - q__33 * c__r4 * ((a__2 ^ 2) - (b__1 ^ 2) + (2 * r__3 * b__1) + 0.5e1 * b__3 ^ 2 - (r__3 ^ 2)) * b__4 + c__r5 * (b__1 - r__3) * ((a__2 ^ 2) - (b__1 ^ 2) + (2 * r__3 * b__1) + 0.7e1 * b__3 ^ 2 - (r__3 ^ 2))) * q__33) * b__5 + (-(b__4 ^ 4) + ((2 * a__2 ^ 2) - (2 * b__1 ^ 2) + (4 * r__3 * b__1) + 0.4e1 * b__3 ^ 2 - (2 * r__3 ^ 2)) * (b__4 ^ 2) - (b__1 ^ 4) + (4 * r__3 * b__1 ^ 3) + ((2 * a__2 ^ 2) - 0.16e2 * b__3 ^ 2 - (6 * r__3 ^ 2)) * (b__1 ^ 2) - 0.4e1 * r__3 * ((a__2 ^ 2) - 0.8e1 * b__3 ^ 2 - (r__3 ^ 2)) * b__1 - (r__3 ^ 4) + ((2 * a__2 ^ 2) - 0.16e2 * b__3 ^ 2) * (r__3 ^ 2) - (a__2 ^ 4) - 0.8e1 * (a__2 ^ 2) * b__3 ^ 2 - 0.7e1 * b__3 ^ 4) * (q__23 ^ 2) + (((4 * b__1 ^ 2) - (8 * r__3 * b__1) + 0.2e1 * b__3 ^ 2 + (4 * r__3 ^ 2)) * (b__4 ^ 2) - 0.6e1 * b__3 ^ 2 * ((a__2 ^ 2) + (3 * b__1 ^ 2) - (6 * r__3 * b__1) + b__3 ^ 2 + (3 * r__3 ^ 2))) * (q__13 ^ 2) - (q__33 ^ 2) * ((b__4 ^ 4) + (-(2 * a__2 ^ 2) - (2 * b__1 ^ 2) + (4 * r__3 * b__1) - 0.14e2 * b__3 ^ 2 - (2 * r__3 ^ 2)) * (b__4 ^ 2) + ((a__2 ^ 2) - (b__1 ^ 2) + (2 * r__3 * b__1) + 0.13e2 * b__3 ^ 2 - (r__3 ^ 2)) * ((a__2 ^ 2) - (b__1 ^ 2) + (2 * r__3 * b__1) + b__3 ^ 2 - (r__3 ^ 2)))) * r__2 - 0.2e1 * q__23 * ((c__r5 * b__5 ^ 5) + ((3 * c__r4 * c__r5 * b__4 - q__33 * (b__1 - r__3)) * b__5 ^ 4) + (((2 * c__r4 ^ 2 * c__r5 + c__r5) * b__4 ^ 2) - (q__33 * c__r4 * (b__1 - r__3) * b__4) - c__r5 * ((a__2 ^ 2) + (b__1 ^ 2) - (2 * r__3 * b__1) + 0.2e1 * b__3 ^ 2 + (r__3 ^ 2))) * (b__5 ^ 3) + ((c__r4 * c__r5 * b__4 ^ 3) - 0.2e1 * q__33 * (b__1 - r__3) * ((c__r4 ^ 2) - 0.3e1 / 0.2e1) * (b__4 ^ 2) - c__r5 * c__r4 * ((a__2 ^ 2) + (3 * b__1 ^ 2) - (6 * r__3 * b__1) + 0.3e1 * b__3 ^ 2 + (3 * r__3 ^ 2)) * b__4 - q__33 * (b__1 - r__3) * ((a__2 ^ 2) - (b__1 ^ 2) + (2 * r__3 * b__1) + 0.2e1 * b__3 ^ 2 - (r__3 ^ 2))) * (b__5 ^ 2) + ((c__r4 * q__33 * (b__1 - r__3) * b__4 ^ 3) - 0.2e1 * ((b__1 ^ 2) - (2 * r__3 * b__1) + b__3 ^ 2 / 0.2e1 + (r__3 ^ 2)) * c__r5 * (b__4 ^ 2) - q__33 * c__r4 * (b__1 - r__3) * ((a__2 ^ 2) - (b__1 ^ 2) + (2 * r__3 * b__1) + 0.5e1 * b__3 ^ 2 - (r__3 ^ 2)) * b__4 + c__r5 * b__3 ^ 2 * ((a__2 ^ 2) + (5 * b__1 ^ 2) - (10 * r__3 * b__1) + b__3 ^ 2 + (5 * r__3 ^ 2))) * b__5 + 0.3e1 * q__33 * ((a__2 ^ 2) - (b__1 ^ 2) + (2 * r__3 * b__1) + b__3 ^ 2 - 0.5e1 / 0.3e1 * (b__4 ^ 2) - (r__3 ^ 2)) * (b__1 - r__3) * b__3 ^ 2)) * r__1 + (-0.5e1 * (-0.2e1 / 0.5e1 * b__4 * b__5 * c__r4 + b__3 ^ 2 - (b__5 ^ 2) / 0.5e1) * q__23 * (r__2 ^ 4) + ((2 * c__r5 * b__5 ^ 3) + ((6 * c__r4 * c__r5 * b__4 - 2 * q__33 * (b__1 - r__3)) * b__5 ^ 2) + ((4 * b__4 ^ 2 * c__r5) - (2 * q__33 * c__r4 * (b__1 - r__3) * b__4) - 0.10e2 * b__3 ^ 2 * c__r5) * b__5 + 0.6e1 * q__33 * b__3 ^ 2 * (b__1 - r__3)) * (r__2 ^ 3) + 0.4e1 * ((b__4 * c__r4 * b__5 ^ 3) / 0.2e1 + (-b__3 ^ 2 + (b__4 ^ 2)) * (b__5 ^ 2) - b__4 * c__r4 * ((a__2 ^ 2) - (b__1 ^ 2) + (2 * r__3 * b__1) + 0.3e1 * b__3 ^ 2 - (b__4 ^ 2) - (r__3 ^ 2)) * b__5 / 0.2e1 + b__3 ^ 2 * ((a__2 ^ 2) - (b__1 ^ 2) + (2 * r__3 * b__1) + b__3 ^ 2 - (b__4 ^ 2) - (r__3 ^ 2))) * q__23 * (r__2 ^ 2) + (-(2 * c__r5 * b__5 ^ 5) + ((-6 * c__r4 * c__r5 * b__4 + 2 * q__33 * (b__1 - r__3)) * b__5 ^ 4) + (((-4 * c__r4 ^ 2 * c__r5 - 2 * c__r5) * b__4 ^ 2) + (2 * q__33 * c__r4 * (b__1 - r__3) * b__4) + 0.2e1 * c__r5 * ((a__2 ^ 2) + (b__1 ^ 2) - (2 * r__3 * b__1) + 0.2e1 * b__3 ^ 2 + (r__3 ^ 2))) * (b__5 ^ 3) + (-(2 * c__r4 * c__r5 * b__4 ^ 3) + 0.4e1 * q__33 * (b__1 - r__3) * ((c__r4 ^ 2) - 0.3e1 / 0.2e1) * (b__4 ^ 2) + 0.2e1 * c__r5 * c__r4 * ((a__2 ^ 2) + (3 * b__1 ^ 2) - (6 * r__3 * b__1) + 0.3e1 * b__3 ^ 2 + (3 * r__3 ^ 2)) * b__4 + 0.2e1 * q__33 * (b__1 - r__3) * ((a__2 ^ 2) - (b__1 ^ 2) + (2 * r__3 * b__1) + 0.2e1 * b__3 ^ 2 - (r__3 ^ 2))) * (b__5 ^ 2) + (-(2 * c__r4 * q__33 * (b__1 - r__3) * b__4 ^ 3) + 0.4e1 * ((b__1 ^ 2) - (2 * r__3 * b__1) + b__3 ^ 2 / 0.2e1 + (r__3 ^ 2)) * c__r5 * (b__4 ^ 2) + 0.2e1 * q__33 * c__r4 * (b__1 - r__3) * ((a__2 ^ 2) - (b__1 ^ 2) + (2 * r__3 * b__1) + 0.5e1 * b__3 ^ 2 - (r__3 ^ 2)) * b__4 - 0.2e1 * c__r5 * b__3 ^ 2 * ((a__2 ^ 2) + (5 * b__1 ^ 2) - (10 * r__3 * b__1) + b__3 ^ 2 + (5 * r__3 ^ 2))) * b__5 - 0.6e1 * q__33 * ((a__2 ^ 2) - (b__1 ^ 2) + (2 * r__3 * b__1) + b__3 ^ 2 - 0.5e1 / 0.3e1 * (b__4 ^ 2) - (r__3 ^ 2)) * (b__1 - r__3) * b__3 ^ 2) * r__2 + (-(b__5 ^ 6) - (4 * b__4 * b__5 ^ 5 * c__r4) + (((-4 * c__r4 ^ 2 - 2) * b__4 ^ 2) + (2 * a__2 ^ 2) + (2 * b__1 ^ 2) - (4 * r__3 * b__1) + 0.3e1 * b__3 ^ 2 + (2 * r__3 ^ 2)) * (b__5 ^ 4) + 0.4e1 * b__4 * c__r4 * ((a__2 ^ 2) + (b__1 ^ 2) - (2 * r__3 * b__1) + 0.2e1 * b__3 ^ 2 - (b__4 ^ 2) + (r__3 ^ 2)) * (b__5 ^ 3) + (-(b__4 ^ 4) + (((4 * c__r4 ^ 2 - 2) * b__1 ^ 2) + ((-8 * c__r4 ^ 2 + 4) * r__3 * b__1) + ((4 * c__r4 ^ 2 - 2) * r__3 ^ 2) + (4 * c__r4 ^ 2 + 4) * b__3 ^ 2 + (2 * a__2 ^ 2)) * (b__4 ^ 2) - (b__1 ^ 4) + (4 * r__3 * b__1 ^ 3) + ((2 * a__2 ^ 2 - 6 * r__3 ^ 2) * b__1 ^ 2) + ((-4 * a__2 ^ 2 * r__3 + 4 * r__3 ^ 3) * b__1) - (a__2 ^ 4) - 0.4e1 * (a__2 ^ 2) * b__3 ^ 2 + (2 * a__2 ^ 2 * r__3 ^ 2) - 0.3e1 * b__3 ^ 4 - (r__3 ^ 4)) * (b__5 ^ 2) - 0.4e1 * b__3 ^ 2 * b__4 * c__r4 * ((a__2 ^ 2) - (b__1 ^ 2) + (2 * r__3 * b__1) + b__3 ^ 2 - (b__4 ^ 2) - (r__3 ^ 2)) * b__5 + b__3 ^ 2 * ((b__4 ^ 4) + (-(2 * a__2 ^ 2) + (6 * b__1 ^ 2) - (12 * r__3 * b__1) - 0.2e1 * b__3 ^ 2 + (6 * r__3 ^ 2)) * (b__4 ^ 2) + ((a__2 ^ 2) - (b__1 ^ 2) + (2 * r__3 * b__1) + b__3 ^ 2 - (r__3 ^ 2)) ^ 2)) * q__23) * q__13) * ((c__r4 - 1) ^ 3) / s__r4 ^ 6 / (b__5 ^ 2);

w__7 =0.4e1 * ((c__r4 + 1) ^ 3) * ((-q__23 ^ 2 / 0.2e1 - q__33 ^ 2 / 0.2e1) * r__2 ^ 5 + (-2 * c__r5 * b__5 - 5 * r__1 * q__13) * q__23 * r__2 ^ 4 + ((-b__4 * b__5 * c__r4 + a__2 ^ 2 - b__1 ^ 2 + 2 * r__3 * b__1 + b__3 ^ 2 + b__4 ^ 2 - b__5 ^ 2 + 5 * r__1 ^ 2 - r__3 ^ 2) * q__23 ^ 2 + (-(2 * c__r5 ^ 2) + (q__13 ^ 2) + 0.2e1 * q__33 ^ 2) * (b__5 ^ 2) + (0.2e1 * c__r4 * b__4 * q__33 ^ 2 + 0.2e1 * c__r5 * q__33 * (b__1 - r__3) + (3 * q__13 ^ 2 * b__4 * c__r4) - (10 * c__r5 * q__13 * r__1)) * b__5 + (a__2 ^ 2 - b__1 ^ 2 + 2 * r__3 * b__1 - 2 * b__3 ^ 2 - b__4 ^ 2 - 4 * r__1 ^ 2 - r__3 ^ 2) * q__33 ^ 2 + 0.6e1 * q__33 * r__1 * (b__1 - r__3) * q__13 - 0.3e1 * ((b__3 ^ 2) - 0.2e1 / 0.3e1 * (b__4 ^ 2) + (3 * r__1 ^ 2)) * (q__13 ^ 2)) * r__2 ^ 3 + 0.2e1 * (-(c__r5 * b__5 ^ 3) + (q__33 * (0.7e1 / 0.2e1 * b__1 - 0.7e1 / 0.2e1 * r__3) - 0.7e1 / 0.2e1 * r__1 * q__13 - (c__r4 * c__r5 * b__4)) * (b__5 ^ 2) + (0.7e1 / 0.2e1 * q__33 * c__r4 * (b__1 - r__3) * b__4 + (6 * c__r5 * r__1 ^ 2) - 0.9e1 / 0.2e1 * q__13 * b__4 * r__1 * c__r4 + (c__r5 * (a__2 ^ 2 - b__1 ^ 2 + 2 * r__3 * b__1 + b__3 ^ 2 - r__3 ^ 2))) * b__5 - 0.7e1 / 0.2e1 * ((b__3 ^ 2) + 0.4e1 / 0.7e1 * (b__4 ^ 2) + (3 * r__1 ^ 2)) * (b__1 - r__3) * q__33 + 0.2e1 * r__1 * ((a__2 ^ 2) - (b__1 ^ 2) + (2 * r__3 * b__1) + 0.11e2 / 0.4e1 * (b__3 ^ 2) - (b__4 ^ 2) + 0.17e2 / 0.4e1 * (r__1 ^ 2) - (r__3 ^ 2)) * q__13) * q__23 * r__2 ^ 2 + ((-(b__5 ^ 4) / 0.2e1 - (b__4 * c__r4 * b__5 ^ 3) + ((a__2 ^ 2 + 3 * b__1 ^ 2 - 6 * r__3 * b__1 + b__3 ^ 2 - b__4 ^ 2 + 7 * r__1 ^ 2 + 3 * r__3 ^ 2) * b__5 ^ 2) + (b__4 * c__r4 * (a__2 ^ 2 + 3 * b__1 ^ 2 - 6 * r__3 * b__1 + b__3 ^ 2 - b__4 ^ 2 + 7 * r__1 ^ 2 + 3 * r__3 ^ 2) * b__5) - 0.13e2 / 0.2e1 * (r__1 ^ 4) + ((-5 * a__2 ^ 2 - 7 * b__1 ^ 2 + 14 * r__3 * b__1 - 9 * b__3 ^ 2 + b__4 ^ 2 - 7 * r__3 ^ 2) * r__1 ^ 2) - (b__1 ^ 4) / 0.2e1 + (2 * r__3 * b__1 ^ 3) + ((a__2 ^ 2 - 3 * b__3 ^ 2 - b__4 ^ 2 - 3 * r__3 ^ 2) * b__1 ^ 2) - (2 * r__3 * (a__2 ^ 2 - 3 * b__3 ^ 2 - b__4 ^ 2 - r__3 ^ 2) * b__1) - (r__3 ^ 4) / 0.2e1 + ((a__2 ^ 2 - 3 * b__3 ^ 2 - b__4 ^ 2) * r__3 ^ 2) - ((a__2 ^ 2 + b__3 ^ 2 - b__4 ^ 2) ^ 2) / 0.2e1) * q__23 ^ 2 + (-(q__13 ^ 2) - 0.3e1 / 0.2e1 * q__33 ^ 2) * (b__5 ^ 4) + (-0.4e1 * c__r4 * b__4 * q__33 ^ 2 + 0.4e1 * c__r5 * q__33 * (b__1 - r__3) - (3 * q__13 ^ 2 * b__4 * c__r4)) * (b__5 ^ 3) + ((5 * r__1 ^ 2 - 2 * b__1 ^ 2 + 4 * r__3 * b__1 - 2 * r__3 ^ 2 + (-2 * c__r4 ^ 2 - 2) * b__4 ^ 2 + 2 * a__2 ^ 2 + 3 * b__3 ^ 2) * q__33 ^ 2 + 0.6e1 * (b__1 - r__3) * (c__r4 * c__r5 * b__4 + r__1 * q__13) * q__33 + ((4 * c__r5 ^ 2 + 2 * q__13 ^ 2) * r__1 ^ 2) - (2 * r__1 * q__13 * c__r4 * c__r5 * b__4) + ((-2 * c__r5 ^ 2 + q__13 ^ 2) * b__1 ^ 2) + ((4 * c__r5 ^ 2 - 2 * q__13 ^ 2) * r__3 * b__1) + ((-2 * c__r5 ^ 2 + q__13 ^ 2) * r__3 ^ 2) + (q__13 ^ 2 * ((-2 * c__r4 ^ 2 - 1) * b__4 ^ 2 + a__2 ^ 2 + 2 * b__3 ^ 2))) * (b__5 ^ 2) + (0.2e1 * b__4 * c__r4 * (a__2 ^ 2 - b__1 ^ 2 + 2 * r__3 * b__1 + 2 * b__3 ^ 2 - b__4 ^ 2 + 4 * r__1 ^ 2 - r__3 ^ 2) * q__33 ^ 2 - 0.2e1 * (b__1 - r__3) * (8 * c__r5 * r__1 ^ 2 - 6 * q__13 * b__4 * r__1 * c__r4 + c__r5 * (a__2 ^ 2 - b__1 ^ 2 + 2 * r__3 * b__1 + 2 * b__3 ^ 2 - b__4 ^ 2 - r__3 ^ 2)) * q__33 - 0.2e1 * q__13 * (-(4 * c__r5 * r__1 ^ 3) - (q__13 * b__4 * r__1 ^ 2 * c__r4) / 0.2e1 + (c__r5 * (a__2 ^ 2 + 5 * b__1 ^ 2 - 10 * r__3 * b__1 + b__4 ^ 2 + 5 * r__3 ^ 2) * r__1) - (q__13 * b__4 * c__r4 * (a__2 ^ 2 + 3 * b__1 ^ 2 - 6 * r__3 * b__1 + 3 * b__3 ^ 2 - b__4 ^ 2 + 3 * r__3 ^ 2)) / 0.2e1)) * b__5 + (-0.7e1 / 0.2e1 * (r__1 ^ 4) + ((-8 * a__2 ^ 2 + 8 * b__1 ^ 2 - 16 * r__3 * b__1 - 11 * b__3 ^ 2 + 8 * b__4 ^ 2 + 8 * r__3 ^ 2) * r__1 ^ 2) - (b__1 ^ 4) / 0.2e1 + (2 * r__3 * b__1 ^ 3) + ((a__2 ^ 2 + 2 * b__3 ^ 2 + b__4 ^ 2 - 3 * r__3 ^ 2) * b__1 ^ 2) - (2 * r__3 * (a__2 ^ 2 + 2 * b__3 ^ 2 + b__4 ^ 2 - r__3 ^ 2) * b__1) - (r__3 ^ 4) / 0.2e1 + ((a__2 ^ 2 + 2 * b__3 ^ 2 + b__4 ^ 2) * r__3 ^ 2) - ((a__2 ^ 2 + 3 * b__3 ^ 2 - b__4 ^ 2) * (a__2 ^ 2 + b__3 ^ 2 - b__4 ^ 2)) / 0.2e1) * q__33 ^ 2 - 0.6e1 * r__1 * q__13 * (b__1 - r__3) * ((a__2 ^ 2) - (b__1 ^ 2) + (2 * r__3 * b__1) + 0.7e1 / 0.3e1 * (b__3 ^ 2) - 0.5e1 / 0.3e1 * (b__4 ^ 2) + (3 * r__1 ^ 2) - (r__3 ^ 2)) * q__33 - (q__13 ^ 2 * (-3 * r__1 ^ 4 + (3 * a__2 ^ 2 + 9 * b__1 ^ 2 - 18 * r__3 * b__1 + 2 * b__3 ^ 2 + b__4 ^ 2 + 9 * r__3 ^ 2) * r__1 ^ 2 + (3 * b__3 ^ 2 - 2 * b__4 ^ 2) * b__1 ^ 2 + (-6 * b__3 ^ 2 + 4 * b__4 ^ 2) * r__3 * b__1 + (3 * b__3 ^ 2 - 2 * b__4 ^ 2) * r__3 ^ 2 + b__3 ^ 2 * (a__2 ^ 2 + b__3 ^ 2 - b__4 ^ 2)))) * r__2 + (((r__3 - b__1) * q__33 + (2 * r__1 * q__13)) * (b__5 ^ 4) + (-0.3e1 * q__33 * c__r4 * (b__1 - r__3) * b__4 + (4 * c__r5 * r__1 ^ 2) + (5 * q__13 * b__4 * r__1 * c__r4) + (2 * c__r5 * (b__1 - r__3) ^ 2)) * (b__5 ^ 3) + ((b__1 - r__3) * (-2 * r__1 ^ 2 - b__1 ^ 2 + 2 * r__3 * b__1 - r__3 ^ 2 + (-2 * c__r4 ^ 2 - 1) * b__4 ^ 2 + a__2 ^ 2 + 2 * b__3 ^ 2) * q__33 + (6 * c__r5 * b__4 * r__1 ^ 2 * c__r4) - 0.3e1 * q__13 * ((b__1 ^ 2) / 0.3e1 - 0.2e1 / 0.3e1 * r__3 * b__1 + (r__3 ^ 2) / 0.3e1 + (-0.2e1 / 0.3e1 * (c__r4 ^ 2) - 0.1e1) * (b__4 ^ 2) + (a__2 ^ 2) + 0.4e1 / 0.3e1 * (b__3 ^ 2)) * r__1 + (4 * c__r5 * b__4 * c__r4 * (b__1 - r__3) ^ 2)) * (b__5 ^ 2) + (b__4 * c__r4 * (b__1 - r__3) * (a__2 ^ 2 - b__1 ^ 2 + 2 * r__3 * b__1 + 3 * b__3 ^ 2 - b__4 ^ 2 + r__1 ^ 2 - r__3 ^ 2) * q__33 - (4 * c__r5 * r__1 ^ 4) + (q__13 * b__4 * r__1 ^ 3 * c__r4) - (2 * c__r5 * (a__2 ^ 2 + 2 * b__1 ^ 2 - 4 * r__3 * b__1 + 2 * b__3 ^ 2 - b__4 ^ 2 + 2 * r__3 ^ 2) * r__1 ^ 2) - 0.3e1 * q__13 * b__4 * ((a__2 ^ 2) - (b__1 ^ 2) + (2 * r__3 * b__1) + 0.5e1 / 0.3e1 * (b__3 ^ 2) - (b__4 ^ 2) - (r__3 ^ 2)) * c__r4 * r__1 - (2 * c__r5 * (b__3 - b__4) * (b__3 + b__4) * (b__1 - r__3) ^ 2)) * b__5 - (-3 * r__1 ^ 4 + (3 * a__2 ^ 2 - 3 * b__1 ^ 2 + 6 * r__3 * b__1 + 2 * b__3 ^ 2 - 7 * b__4 ^ 2 - 3 * r__3 ^ 2) * r__1 ^ 2 + b__3 ^ 2 * (a__2 ^ 2 - b__1 ^ 2 + 2 * r__3 * b__1 + b__3 ^ 2 - b__4 ^ 2 - r__3 ^ 2)) * (b__1 - r__3) * q__33 + r__1 * q__13 * (-(2 * r__1 ^ 4) + ((a__2 ^ 2 - b__1 ^ 2 + 2 * r__3 * b__1 - b__4 ^ 2 - r__3 ^ 2) * r__1 ^ 2) + (b__1 ^ 4) - (4 * r__3 * b__1 ^ 3) + ((-2 * a__2 ^ 2 - 3 * b__3 ^ 2 + 6 * b__4 ^ 2 + 6 * r__3 ^ 2) * b__1 ^ 2) + 0.4e1 * r__3 * ((a__2 ^ 2) + 0.3e1 / 0.2e1 * (b__3 ^ 2) - (3 * b__4 ^ 2) - (r__3 ^ 2)) * b__1 + (r__3 ^ 4) + ((-2 * a__2 ^ 2 - 3 * b__3 ^ 2 + 6 * b__4 ^ 2) * r__3 ^ 2) + ((a__2 ^ 2 + 2 * b__3 ^ 2 - b__4 ^ 2) * (a__2 ^ 2 + b__3 ^ 2 - b__4 ^ 2)))) * q__23) * b__3 * ((c__r4 - 1) ^ 3) / s__r4 ^ 6 / (b__5 ^ 2);

w__8 =0.2e1 * ((c__r4 + 1) ^ 3) * (((3 * q__23 ^ 2 + 3 * q__33 ^ 2) * r__1 ^ 5) - (10 * ((r__3 - b__1) * q__33 + r__2 * q__23) * q__13 * r__1 ^ 4) + (((-6 * q__23 ^ 2 - 6 * q__33 ^ 2) * b__5 ^ 2) + ((-8 * c__r4 * b__4 * q__33 ^ 2 + 8 * c__r5 * q__33 * (b__1 - r__3) - 8 * b__4 * c__r4 * q__23 ^ 2 - 8 * c__r5 * q__23 * r__2) * b__5) + ((4 * a__2 ^ 2 - 4 * b__1 ^ 2 + 8 * r__3 * b__1 + 10 * b__3 ^ 2 - 4 * b__4 ^ 2 + 4 * r__2 ^ 2 - 4 * r__3 ^ 2) * q__33 ^ 2) + (16 * q__23 * q__33 * (b__1 - r__3) * r__2) + ((8 * b__1 ^ 2 - 16 * r__3 * b__1 + 8 * r__2 ^ 2 + 8 * r__3 ^ 2) * q__13 ^ 2) + 0.4e1 * ((a__2 ^ 2) + (b__1 ^ 2) - (2 * r__3 * b__1) + 0.5e1 / 0.2e1 * (b__3 ^ 2) - (b__4 ^ 2) - (r__2 ^ 2) + (r__3 ^ 2)) * (q__23 ^ 2)) * (r__1 ^ 3) - 0.6e1 * q__13 * ((((2 * b__1 - 2 * r__3) * q__33 - 2 * r__2 * q__23) * b__5 ^ 2) + ((3 * q__33 * c__r4 * (b__1 - r__3) * b__4 - 3 * q__23 * b__4 * c__r4 * r__2 - 2 * c__r5 * b__1 ^ 2 + 4 * b__1 * c__r5 * r__3 - 2 * c__r5 * r__2 ^ 2 - 2 * c__r5 * r__3 ^ 2) * b__5) + ((r__3 - b__1) * q__33 + r__2 * q__23) * ((a__2 ^ 2) - (b__1 ^ 2) + (2 * r__3 * b__1) + 0.10e2 / 0.3e1 * (b__3 ^ 2) - (b__4 ^ 2) - (r__2 ^ 2) - (r__3 ^ 2))) * (r__1 ^ 2) + (((3 * q__23 ^ 2 + 3 * q__33 ^ 2) * b__5 ^ 4) + ((8 * c__r4 * b__4 * q__33 ^ 2 - 8 * c__r5 * q__33 * (b__1 - r__3) + 8 * b__4 * c__r4 * q__23 ^ 2 + 8 * c__r5 * q__23 * r__2) * b__5 ^ 3) + (((4 * b__1 ^ 2 - 8 * r__3 * b__1 + 4 * r__3 ^ 2 + (4 * c__r4 ^ 2 + 4) * b__4 ^ 2 - 4 * a__2 ^ 2 - 6 * b__3 ^ 2 - 4 * r__2 ^ 2) * q__33 ^ 2) - 0.12e2 * ((c__r4 * c__r5 * b__4) + 0.4e1 / 0.3e1 * r__2 * q__23) * (b__1 - r__3) * q__33 + ((-4 * b__1 ^ 2 + 8 * r__3 * b__1 - 4 * r__2 ^ 2 - 4 * r__3 ^ 2) * q__13 ^ 2) + ((4 * c__r5 ^ 2 - 4 * q__23 ^ 2) * b__1 ^ 2) + ((-8 * c__r5 ^ 2 + 8 * q__23 ^ 2) * r__3 * b__1) + ((4 * c__r5 ^ 2 - 4 * q__23 ^ 2) * r__3 ^ 2) + (((4 * c__r4 ^ 2 + 4) * b__4 ^ 2 - 4 * a__2 ^ 2 - 6 * b__3 ^ 2 + 4 * r__2 ^ 2) * q__23 ^ 2) + (12 * r__2 * q__23 * c__r4 * c__r5 * b__4) + (4 * c__r5 ^ 2 * r__2 ^ 2)) * (b__5 ^ 2) + ((-4 * b__4 * c__r4 * (a__2 ^ 2 - b__1 ^ 2 + 2 * r__3 * b__1 + 2 * b__3 ^ 2 - b__4 ^ 2 + r__2 ^ 2 - r__3 ^ 2) * q__33 ^ 2 + 4 * (-c__r5 * b__1 ^ 2 + 2 * b__1 * c__r5 * r__3 - c__r5 * r__3 ^ 2 - 4 * q__23 * b__4 * c__r4 * r__2 + c__r5 * (a__2 ^ 2 + 2 * b__3 ^ 2 - b__4 ^ 2 - r__2 ^ 2)) * (b__1 - r__3) * q__33 - 8 * b__4 * c__r4 * (b__1 ^ 2 - 2 * r__3 * b__1 + r__2 ^ 2 + r__3 ^ 2) * q__13 ^ 2 - 4 * ((b__4 * c__r4 * q__23 - c__r5 * r__2) * b__1 ^ 2 + 2 * r__3 * (-b__4 * c__r4 * q__23 + c__r5 * r__2) * b__1 + (b__4 * c__r4 * q__23 - c__r5 * r__2) * r__3 ^ 2 + (a__2 ^ 2 + 2 * b__3 ^ 2 - b__4 ^ 2 - r__2 ^ 2) * (b__4 * c__r4 * q__23 + c__r5 * r__2)) * q__23) * b__5) + ((b__1 ^ 4 - 4 * r__3 * b__1 ^ 3 + (-2 * a__2 ^ 2 - 4 * b__3 ^ 2 - 2 * b__4 ^ 2 + 2 * r__2 ^ 2 + 6 * r__3 ^ 2) * b__1 ^ 2 + 4 * r__3 * (a__2 ^ 2 + 2 * b__3 ^ 2 + b__4 ^ 2 - r__2 ^ 2 - r__3 ^ 2) * b__1 + r__3 ^ 4 + (-2 * a__2 ^ 2 - 4 * b__3 ^ 2 - 2 * b__4 ^ 2 + 2 * r__2 ^ 2) * r__3 ^ 2 + b__4 ^ 4 + (-2 * a__2 ^ 2 - 4 * b__3 ^ 2 + 2 * r__2 ^ 2) * b__4 ^ 2 + r__2 ^ 4 + (-2 * a__2 ^ 2 + 4 * b__3 ^ 2) * r__2 ^ 2 + a__2 ^ 4 + 4 * a__2 ^ 2 * b__3 ^ 2 + 3 * b__3 ^ 4) * q__33 ^ 2) + 0.16e2 * r__2 * ((b__3 ^ 2) + (b__4 ^ 2) / 0.2e1) * (b__1 - r__3) * q__23 * q__33 + 0.8e1 * (b__1 ^ 2 - 2 * r__3 * b__1 + r__2 ^ 2 + r__3 ^ 2) * ((b__3 ^ 2) - (b__4 ^ 2) / 0.2e1) * (q__13 ^ 2) + (q__23 ^ 2 * (b__1 ^ 4 - 4 * r__3 * b__1 ^ 3 + (-2 * a__2 ^ 2 + 4 * b__3 ^ 2 + 2 * b__4 ^ 2 + 2 * r__2 ^ 2 + 6 * r__3 ^ 2) * b__1 ^ 2 + 4 * r__3 * (a__2 ^ 2 - 2 * b__3 ^ 2 - b__4 ^ 2 - r__2 ^ 2 - r__3 ^ 2) * b__1 + r__3 ^ 4 + (-2 * a__2 ^ 2 + 4 * b__3 ^ 2 + 2 * b__4 ^ 2 + 2 * r__2 ^ 2) * r__3 ^ 2 + b__4 ^ 4 + (-2 * a__2 ^ 2 - 4 * b__3 ^ 2 - 2 * r__2 ^ 2) * b__4 ^ 2 + (a__2 ^ 2 + 3 * b__3 ^ 2 - r__2 ^ 2) * (a__2 ^ 2 + b__3 ^ 2 - r__2 ^ 2)))) * r__1 - 0.2e1 * ((((r__3 - b__1) * q__33 + r__2 * q__23) * b__5 ^ 4) + ((-3 * q__33 * c__r4 * (b__1 - r__3) * b__4 + 3 * q__23 * b__4 * c__r4 * r__2 + 2 * c__r5 * b__1 ^ 2 - 4 * b__1 * c__r5 * r__3 + 2 * c__r5 * r__2 ^ 2 + 2 * c__r5 * r__3 ^ 2) * b__5 ^ 3) + (((b__1 - r__3) * (-b__1 ^ 2 + 2 * r__3 * b__1 - r__3 ^ 2 + (-2 * c__r4 ^ 2 - 1) * b__4 ^ 2 + a__2 ^ 2 + 2 * b__3 ^ 2 - r__2 ^ 2) * q__33 + (4 * c__r4 * c__r5 * b__4 + r__2 * q__23) * b__1 ^ 2 + (-8 * c__r4 * c__r5 * b__4 - 2 * r__2 * q__23) * r__3 * b__1 + (4 * c__r4 * c__r5 * b__4 + r__2 * q__23) * r__3 ^ 2 - (((-2 * c__r4 ^ 2 - 1) * b__4 ^ 2 + a__2 ^ 2 + 2 * b__3 ^ 2 - r__2 ^ 2) * q__23 - 4 * c__r5 * b__4 * r__2 * c__r4) * r__2) * b__5 ^ 2) + ((b__4 * c__r4 * (b__1 - r__3) * (a__2 ^ 2 - b__1 ^ 2 + 2 * r__3 * b__1 + 3 * b__3 ^ 2 - b__4 ^ 2 - r__2 ^ 2 - r__3 ^ 2) * q__33) + ((q__23 * b__4 * c__r4 * r__2 - 2 * b__3 ^ 2 * c__r5 + 2 * b__4 ^ 2 * c__r5) * b__1 ^ 2) + 0.4e1 * (-(q__23 * b__4 * c__r4 * r__2) / 0.2e1 + (b__3 ^ 2 * c__r5) - (b__4 ^ 2 * c__r5)) * r__3 * b__1 + ((q__23 * b__4 * c__r4 * r__2 - 2 * b__3 ^ 2 * c__r5 + 2 * b__4 ^ 2 * c__r5) * r__3 ^ 2) - (r__2 * (b__4 * c__r4 * (a__2 ^ 2 + 3 * b__3 ^ 2 - b__4 ^ 2 - r__2 ^ 2) * q__23 + 2 * c__r5 * r__2 * (b__3 - b__4) * (b__3 + b__4)))) * b__5 + (((r__3 - b__1) * q__33 + r__2 * q__23) * (a__2 ^ 2 - b__1 ^ 2 + 2 * r__3 * b__1 + b__3 ^ 2 - b__4 ^ 2 - r__2 ^ 2 - r__3 ^ 2) * b__3 ^ 2)) * q__13) * b__3 * ((c__r4 - 1) ^ 3) / s__r4 ^ 6 / (b__5 ^ 2);

w__9 =((c__r4 + 1) ^ 3) * (((-q__23 ^ 2 - q__33 ^ 2) * b__5 ^ 6) + ((-4 * c__r4 * b__4 * q__33 ^ 2 + 4 * c__r5 * q__33 * (b__1 - r__3) - 4 * b__4 * c__r4 * q__23 ^ 2 - 4 * c__r5 * q__23 * r__2) * b__5 ^ 5) + (((3 * q__23 ^ 2 + 3 * q__33 ^ 2) * r__1 ^ 2) - (4 * ((r__3 - b__1) * q__33 + r__2 * q__23) * q__13 * r__1) + ((-2 * b__1 ^ 2 + 4 * r__3 * b__1 - 2 * r__3 ^ 2 + (-4 * c__r4 ^ 2 - 2) * b__4 ^ 2 + 2 * a__2 ^ 2 + 3 * b__3 ^ 2 + 2 * r__2 ^ 2) * q__33 ^ 2) + 0.12e2 * ((c__r4 * c__r5 * b__4) + 0.2e1 / 0.3e1 * r__2 * q__23) * (b__1 - r__3) * q__33 + ((-4 * c__r5 ^ 2 + 2 * q__23 ^ 2) * b__1 ^ 2) + ((8 * c__r5 ^ 2 - 4 * q__23 ^ 2) * r__3 * b__1) + ((-4 * c__r5 ^ 2 + 2 * q__23 ^ 2) * r__3 ^ 2) + (((-4 * c__r4 ^ 2 - 2) * b__4 ^ 2 + 2 * a__2 ^ 2 + 3 * b__3 ^ 2 - 2 * r__2 ^ 2) * q__23 ^ 2) - (12 * r__2 * q__23 * c__r4 * c__r5 * b__4) - (4 * c__r5 ^ 2 * r__2 ^ 2)) * (b__5 ^ 4) + (((8 * c__r4 * b__4 * q__33 ^ 2 - 8 * c__r5 * q__33 * (b__1 - r__3) + 8 * b__4 * c__r4 * q__23 ^ 2 + 8 * c__r5 * q__23 * r__2) * r__1 ^ 2) - 0.8e1 * q__13 * (-0.3e1 / 0.2e1 * q__33 * c__r4 * (b__1 - r__3) * b__4 + 0.3e1 / 0.2e1 * q__23 * b__4 * c__r4 * r__2 + (c__r5 * b__1 ^ 2) - (2 * b__1 * c__r5 * r__3) + (c__r5 * r__2 ^ 2) + (c__r5 * r__3 ^ 2)) * r__1 + (4 * b__4 * c__r4 * (a__2 ^ 2 - b__1 ^ 2 + 2 * r__3 * b__1 + 2 * b__3 ^ 2 - b__4 ^ 2 + r__2 ^ 2 - r__3 ^ 2) * q__33 ^ 2) - (4 * (-c__r5 * b__1 ^ 2 + 2 * b__1 * c__r5 * r__3 - c__r5 * r__3 ^ 2 - 4 * q__23 * b__4 * c__r4 * r__2 + ((-2 * c__r4 ^ 2 - 1) * b__4 ^ 2 + a__2 ^ 2 + 2 * b__3 ^ 2 - r__2 ^ 2) * c__r5) * (b__1 - r__3) * q__33) + ((-8 * c__r4 * b__4 * c__r5 ^ 2 + 4 * b__4 * c__r4 * q__23 ^ 2 - 4 * c__r5 * q__23 * r__2) * b__1 ^ 2) + 0.16e2 * r__3 * ((c__r4 * b__4 * c__r5 ^ 2) - (b__4 * c__r4 * q__23 ^ 2) / 0.2e1 + (c__r5 * q__23 * r__2) / 0.2e1) * b__1 + ((-8 * c__r4 * b__4 * c__r5 ^ 2 + 4 * b__4 * c__r4 * q__23 ^ 2 - 4 * c__r5 * q__23 * r__2) * r__3 ^ 2) + (4 * (b__4 * c__r4 * q__23 + c__r5 * r__2) * ((a__2 ^ 2 + 2 * b__3 ^ 2 - b__4 ^ 2 - r__2 ^ 2) * q__23 - 2 * c__r5 * b__4 * r__2 * c__r4))) * (b__5 ^ 3) + (((-3 * q__23 ^ 2 - 3 * q__33 ^ 2) * r__1 ^ 4) + (8 * ((r__3 - b__1) * q__33 + r__2 * q__23) * q__13 * r__1 ^ 3) + (((4 * b__1 ^ 2 - 8 * r__3 * b__1 + 4 * r__3 ^ 2 + (4 * c__r4 ^ 2 + 4) * b__4 ^ 2 - 4 * a__2 ^ 2 - 18 * b__3 ^ 2 - 4 * r__2 ^ 2) * q__33 ^ 2) - 0.12e2 * ((c__r4 * c__r5 * b__4) + 0.4e1 / 0.3e1 * r__2 * q__23) * (b__1 - r__3) * q__33 + ((4 * c__r5 ^ 2 - 4 * q__13 ^ 2 - 4 * q__23 ^ 2) * b__1 ^ 2) - (8 * r__3 * (c__r5 ^ 2 - q__13 ^ 2 - q__23 ^ 2) * b__1) + ((4 * c__r5 ^ 2 - 4 * q__13 ^ 2 - 4 * q__23 ^ 2) * r__3 ^ 2) + (((4 * c__r4 ^ 2 + 4) * b__4 ^ 2 - 4 * a__2 ^ 2 - 18 * b__3 ^ 2 + 4 * r__2 ^ 2) * q__23 ^ 2) + (12 * r__2 * q__23 * c__r4 * c__r5 * b__4) + ((4 * c__r5 ^ 2 - 4 * q__13 ^ 2) * r__2 ^ 2)) * (r__1 ^ 2) + (4 * (-(b__1 - r__3) * (-b__1 ^ 2 + 2 * r__3 * b__1 - r__3 ^ 2 + (-2 * c__r4 ^ 2 - 1) * b__4 ^ 2 + a__2 ^ 2 + 6 * b__3 ^ 2 - r__2 ^ 2) * q__33 + (-4 * c__r4 * c__r5 * b__4 - r__2 * q__23) * b__1 ^ 2 + (8 * c__r4 * c__r5 * b__4 + 2 * r__2 * q__23) * r__3 * b__1 + (-4 * c__r4 * c__r5 * b__4 - r__2 * q__23) * r__3 ^ 2 + r__2 * (((-2 * c__r4 ^ 2 - 1) * b__4 ^ 2 + a__2 ^ 2 + 6 * b__3 ^ 2 - r__2 ^ 2) * q__23 - 4 * c__r5 * b__4 * r__2 * c__r4)) * q__13 * r__1) + ((-b__1 ^ 4 + 4 * r__3 * b__1 ^ 3 + (-6 * r__3 ^ 2 + (-4 * c__r4 ^ 2 + 2) * b__4 ^ 2 + 2 * a__2 ^ 2 + 4 * b__3 ^ 2 - 2 * r__2 ^ 2) * b__1 ^ 2 - 4 * r__3 * (-r__3 ^ 2 + (-2 * c__r4 ^ 2 + 1) * b__4 ^ 2 + a__2 ^ 2 + 2 * b__3 ^ 2 - r__2 ^ 2) * b__1 - r__3 ^ 4 + ((-4 * c__r4 ^ 2 + 2) * b__4 ^ 2 + 2 * a__2 ^ 2 + 4 * b__3 ^ 2 - 2 * r__2 ^ 2) * r__3 ^ 2 - b__4 ^ 4 + ((4 * c__r4 ^ 2 + 4) * b__3 ^ 2 + (4 * c__r4 ^ 2 - 2) * r__2 ^ 2 + 2 * a__2 ^ 2) * b__4 ^ 2 - 3 * b__3 ^ 4 + (-4 * a__2 ^ 2 - 4 * r__2 ^ 2) * b__3 ^ 2 - (a__2 - r__2) ^ 2 * (a__2 + r__2) ^ 2) * q__33 ^ 2) - 0.4e1 * (-(c__r5 * b__1 ^ 2 * b__4 * c__r4) + (2 * c__r5 * b__1 * b__4 * r__3 * c__r4) - (c__r5 * b__4 * c__r4 * r__3 ^ 2) + 0.4e1 * ((-(c__r4 ^ 2) + 0.1e1 / 0.2e1) * (b__4 ^ 2) + (b__3 ^ 2)) * r__2 * q__23 + (c__r5 * b__4 * c__r4 * (a__2 ^ 2 + 3 * b__3 ^ 2 - b__4 ^ 2 - r__2 ^ 2))) * (b__1 - r__3) * q__33 - (q__23 ^ 2 * b__1 ^ 4) + (4 * q__23 ^ 2 * r__3 * b__1 ^ 3) + ((-6 * r__3 ^ 2 * q__23 ^ 2 + ((4 * c__r4 ^ 2 - 2) * b__4 ^ 2 + 2 * a__2 ^ 2 - 4 * b__3 ^ 2 - 2 * r__2 ^ 2) * q__23 ^ 2 - 4 * r__2 * q__23 * c__r4 * c__r5 * b__4 - 4 * c__r5 ^ 2 * b__4 ^ 2 + (4 * c__r5 ^ 2 - 4 * q__13 ^ 2) * b__3 ^ 2) * b__1 ^ 2) - (4 * r__3 * (-r__3 ^ 2 * q__23 ^ 2 + ((2 * c__r4 ^ 2 - 1) * b__4 ^ 2 + a__2 ^ 2 - 2 * b__3 ^ 2 - r__2 ^ 2) * q__23 ^ 2 - 2 * r__2 * q__23 * c__r4 * c__r5 * b__4 - 2 * c__r5 ^ 2 * b__4 ^ 2 + (2 * c__r5 ^ 2 - 2 * q__13 ^ 2) * b__3 ^ 2) * b__1) - (q__23 ^ 2 * r__3 ^ 4) + ((((4 * c__r4 ^ 2 - 2) * b__4 ^ 2 + 2 * a__2 ^ 2 - 4 * b__3 ^ 2 - 2 * r__2 ^ 2) * q__23 ^ 2 - 4 * r__2 * q__23 * c__r4 * c__r5 * b__4 - 4 * c__r5 ^ 2 * b__4 ^ 2 + (4 * c__r5 ^ 2 - 4 * q__13 ^ 2) * b__3 ^ 2) * r__3 ^ 2) + ((-b__4 ^ 4 + ((4 * c__r4 ^ 2 + 4) * b__3 ^ 2 + (-4 * c__r4 ^ 2 + 2) * r__2 ^ 2 + 2 * a__2 ^ 2) * b__4 ^ 2 - (a__2 ^ 2 + 3 * b__3 ^ 2 - r__2 ^ 2) * (a__2 ^ 2 + b__3 ^ 2 - r__2 ^ 2)) * q__23 ^ 2) + (4 * c__r5 * b__4 * r__2 * c__r4 * (a__2 ^ 2 + 3 * b__3 ^ 2 - b__4 ^ 2 - r__2 ^ 2) * q__23) + (4 * (-c__r5 ^ 2 * b__4 ^ 2 + b__3 ^ 2 * (c__r5 ^ 2 - q__13 ^ 2)) * r__2 ^ 2)) * (b__5 ^ 2) + (((-4 * c__r4 * b__4 * q__33 ^ 2 + 4 * c__r5 * q__33 * (b__1 - r__3) - 4 * b__4 * c__r4 * q__23 ^ 2 - 4 * c__r5 * q__23 * r__2) * r__1 ^ 4) + 0.8e1 * q__13 * (-0.3e1 / 0.2e1 * q__33 * c__r4 * (b__1 - r__3) * b__4 + 0.3e1 / 0.2e1 * q__23 * b__4 * c__r4 * r__2 + (c__r5 * b__1 ^ 2) - (2 * b__1 * c__r5 * r__3) + (c__r5 * r__2 ^ 2) + (c__r5 * r__3 ^ 2)) * (r__1 ^ 3) + ((-4 * b__4 * c__r4 * (a__2 ^ 2 - b__1 ^ 2 + 2 * r__3 * b__1 + 6 * b__3 ^ 2 - b__4 ^ 2 + r__2 ^ 2 - r__3 ^ 2) * q__33 ^ 2 + 4 * (b__1 - r__3) * (-c__r5 * b__1 ^ 2 + 2 * b__1 * c__r5 * r__3 - c__r5 * r__3 ^ 2 - 4 * q__23 * b__4 * c__r4 * r__2 + c__r5 * (a__2 ^ 2 + 6 * b__3 ^ 2 - b__4 ^ 2 - r__2 ^ 2)) * q__33 + (-8 * q__13 ^ 2 * b__4 * c__r4 - 4 * b__4 * c__r4 * q__23 ^ 2 + 4 * c__r5 * q__23 * r__2) * b__1 ^ 2 - 8 * r__3 * (-2 * q__13 ^ 2 * b__4 * c__r4 - b__4 * c__r4 * q__23 ^ 2 + c__r5 * q__23 * r__2) * b__1 + (-8 * q__13 ^ 2 * b__4 * c__r4 - 4 * b__4 * c__r4 * q__23 ^ 2 + 4 * c__r5 * q__23 * r__2) * r__3 ^ 2 - 4 * b__4 * c__r4 * (a__2 ^ 2 + 6 * b__3 ^ 2 - b__4 ^ 2 - r__2 ^ 2) * q__23 ^ 2 - 4 * c__r5 * r__2 * (a__2 ^ 2 + 6 * b__3 ^ 2 - b__4 ^ 2 - r__2 ^ 2) * q__23 - 8 * q__13 ^ 2 * b__4 * r__2 ^ 2 * c__r4) * r__1 ^ 2) + 0.4e1 * q__13 * (-(b__4 * c__r4 * (b__1 - r__3) * (a__2 ^ 2 - b__1 ^ 2 + 2 * r__3 * b__1 + 9 * b__3 ^ 2 - b__4 ^ 2 - r__2 ^ 2 - r__3 ^ 2) * q__33) + ((-q__23 * b__4 * c__r4 * r__2 + 6 * b__3 ^ 2 * c__r5 - 2 * b__4 ^ 2 * c__r5) * b__1 ^ 2) - 0.12e2 * r__3 * (-(q__23 * b__4 * c__r4 * r__2) / 0.6e1 + ((b__3 ^ 2) - (b__4 ^ 2) / 0.3e1) * c__r5) * b__1 + ((-q__23 * b__4 * c__r4 * r__2 + 6 * b__3 ^ 2 * c__r5 - 2 * b__4 ^ 2 * c__r5) * r__3 ^ 2) + r__2 * ((b__4 * c__r4 * (a__2 ^ 2 + 9 * b__3 ^ 2 - b__4 ^ 2 - r__2 ^ 2) * q__23) + 0.6e1 * r__2 * ((b__3 ^ 2) - (b__4 ^ 2) / 0.3e1) * c__r5)) * r__1 - (4 * (b__4 * c__r4 * (a__2 ^ 2 - b__1 ^ 2 + 2 * r__3 * b__1 + b__3 ^ 2 - b__4 ^ 2 + r__2 ^ 2 - r__3 ^ 2) * q__33 ^ 2 - (-c__r5 * b__1 ^ 2 + 2 * b__1 * c__r5 * r__3 - c__r5 * r__3 ^ 2 - 4 * q__23 * b__4 * c__r4 * r__2 + c__r5 * (a__2 ^ 2 + b__3 ^ 2 - b__4 ^ 2 - r__2 ^ 2)) * (b__1 - r__3) * q__33 + (2 * q__13 ^ 2 * b__4 * c__r4 + b__4 * c__r4 * q__23 ^ 2 - c__r5 * q__23 * r__2) * b__1 ^ 2 + 2 * r__3 * (-2 * q__13 ^ 2 * b__4 * c__r4 - b__4 * c__r4 * q__23 ^ 2 + c__r5 * q__23 * r__2) * b__1 + (2 * q__13 ^ 2 * b__4 * c__r4 + b__4 * c__r4 * q__23 ^ 2 - c__r5 * q__23 * r__2) * r__3 ^ 2 + b__4 * c__r4 * (a__2 ^ 2 + b__3 ^ 2 - b__4 ^ 2 - r__2 ^ 2) * q__23 ^ 2 + c__r5 * r__2 * (a__2 ^ 2 + b__3 ^ 2 - b__4 ^ 2 - r__2 ^ 2) * q__23 + 2 * q__13 ^ 2 * b__4 * r__2 ^ 2 * c__r4) * b__3 ^ 2)) * b__5 + ((q__23 ^ 2 + q__33 ^ 2) * r__1 ^ 6) - (4 * ((r__3 - b__1) * q__33 + r__2 * q__23) * q__13 * r__1 ^ 5) + (((2 * a__2 ^ 2 - 2 * b__1 ^ 2 + 4 * r__3 * b__1 + 15 * b__3 ^ 2 - 2 * b__4 ^ 2 + 2 * r__2 ^ 2 - 2 * r__3 ^ 2) * q__33 ^ 2 + 8 * q__23 * q__33 * (b__1 - r__3) * r__2 + (4 * q__13 ^ 2 + 2 * q__23 ^ 2) * b__1 ^ 2 + (-8 * q__13 ^ 2 - 4 * q__23 ^ 2) * r__3 * b__1 + (4 * q__13 ^ 2 + 2 * q__23 ^ 2) * r__3 ^ 2 + (2 * a__2 ^ 2 + 15 * b__3 ^ 2 - 2 * b__4 ^ 2 - 2 * r__2 ^ 2) * q__23 ^ 2 + 4 * q__13 ^ 2 * r__2 ^ 2) * r__1 ^ 4) - (4 * ((r__3 - b__1) * q__33 + r__2 * q__23) * (a__2 ^ 2 - b__1 ^ 2 + 2 * r__3 * b__1 + 10 * b__3 ^ 2 - b__4 ^ 2 - r__2 ^ 2 - r__3 ^ 2) * q__13 * r__1 ^ 3) + (((b__1 ^ 4 - 4 * r__3 * b__1 ^ 3 + (-2 * a__2 ^ 2 - 12 * b__3 ^ 2 - 2 * b__4 ^ 2 + 2 * r__2 ^ 2 + 6 * r__3 ^ 2) * b__1 ^ 2 + 4 * r__3 * (a__2 ^ 2 + 6 * b__3 ^ 2 + b__4 ^ 2 - r__2 ^ 2 - r__3 ^ 2) * b__1 + r__3 ^ 4 + (-2 * a__2 ^ 2 - 12 * b__3 ^ 2 - 2 * b__4 ^ 2 + 2 * r__2 ^ 2) * r__3 ^ 2 + b__4 ^ 4 + (-2 * a__2 ^ 2 - 12 * b__3 ^ 2 + 2 * r__2 ^ 2) * b__4 ^ 2 + 15 * b__3 ^ 4 + (12 * a__2 ^ 2 + 12 * r__2 ^ 2) * b__3 ^ 2 + (a__2 - r__2) ^ 2 * (a__2 + r__2) ^ 2) * q__33 ^ 2) + 0.48e2 * r__2 * (b__1 - r__3) * q__23 * ((b__3 ^ 2) + (b__4 ^ 2) / 0.6e1) * q__33 + (q__23 ^ 2 * b__1 ^ 4) - (4 * q__23 ^ 2 * r__3 * b__1 ^ 3) + ((6 * r__3 ^ 2 * q__23 ^ 2 + (-2 * a__2 ^ 2 + 12 * b__3 ^ 2 + 2 * b__4 ^ 2 + 2 * r__2 ^ 2) * q__23 ^ 2 + 24 * b__3 ^ 2 * q__13 ^ 2 - 4 * q__13 ^ 2 * b__4 ^ 2) * b__1 ^ 2) + (4 * r__3 * (-r__3 ^ 2 * q__23 ^ 2 + (a__2 ^ 2 - 6 * b__3 ^ 2 - b__4 ^ 2 - r__2 ^ 2) * q__23 ^ 2 - 12 * b__3 ^ 2 * q__13 ^ 2 + 2 * q__13 ^ 2 * b__4 ^ 2) * b__1) + (q__23 ^ 2 * r__3 ^ 4) + (((-2 * a__2 ^ 2 + 12 * b__3 ^ 2 + 2 * b__4 ^ 2 + 2 * r__2 ^ 2) * q__23 ^ 2 + 24 * b__3 ^ 2 * q__13 ^ 2 - 4 * q__13 ^ 2 * b__4 ^ 2) * r__3 ^ 2) + ((b__4 ^ 4 + (-2 * a__2 ^ 2 - 12 * b__3 ^ 2 - 2 * r__2 ^ 2) * b__4 ^ 2 + 15 * b__3 ^ 4 + (12 * a__2 ^ 2 - 12 * r__2 ^ 2) * b__3 ^ 2 + (a__2 - r__2) ^ 2 * (a__2 + r__2) ^ 2) * q__23 ^ 2) + 0.24e2 * ((b__3 ^ 2) - (b__4 ^ 2) / 0.6e1) * (q__13 ^ 2) * (r__2 ^ 2)) * (r__1 ^ 2) - 0.12e2 * ((r__3 - b__1) * q__33 + r__2 * q__23) * ((a__2 ^ 2) - (b__1 ^ 2) + (2 * r__3 * b__1) + 0.5e1 / 0.3e1 * (b__3 ^ 2) - (b__4 ^ 2) - (r__2 ^ 2) - (r__3 ^ 2)) * q__13 * (b__3 ^ 2) * r__1 + (b__3 ^ 2 * ((b__1 ^ 4 - 4 * r__3 * b__1 ^ 3 + (-2 * a__2 ^ 2 - 2 * b__3 ^ 2 - 2 * b__4 ^ 2 + 2 * r__2 ^ 2 + 6 * r__3 ^ 2) * b__1 ^ 2 + 4 * r__3 * (a__2 ^ 2 + b__3 ^ 2 + b__4 ^ 2 - r__2 ^ 2 - r__3 ^ 2) * b__1 + r__3 ^ 4 + (-2 * a__2 ^ 2 - 2 * b__3 ^ 2 - 2 * b__4 ^ 2 + 2 * r__2 ^ 2) * r__3 ^ 2 + b__4 ^ 4 + (-2 * a__2 ^ 2 - 2 * b__3 ^ 2 + 2 * r__2 ^ 2) * b__4 ^ 2 + (b__3 ^ 2 + (a__2 - r__2) ^ 2) * (b__3 ^ 2 + (a__2 + r__2) ^ 2)) * q__33 ^ 2 + 8 * q__23 * r__2 * (b__3 ^ 2 + b__4 ^ 2) * (b__1 - r__3) * q__33 + q__23 ^ 2 * b__1 ^ 4 - 4 * q__23 ^ 2 * r__3 * b__1 ^ 3 + (6 * r__3 ^ 2 * q__23 ^ 2 + (-2 * a__2 ^ 2 + 2 * b__3 ^ 2 + 2 * b__4 ^ 2 + 2 * r__2 ^ 2) * q__23 ^ 2 + 4 * b__3 ^ 2 * q__13 ^ 2 - 4 * q__13 ^ 2 * b__4 ^ 2) * b__1 ^ 2 + 4 * r__3 * (-r__3 ^ 2 * q__23 ^ 2 + (a__2 ^ 2 - b__3 ^ 2 - b__4 ^ 2 - r__2 ^ 2) * q__23 ^ 2 - 2 * b__3 ^ 2 * q__13 ^ 2 + 2 * q__13 ^ 2 * b__4 ^ 2) * b__1 + q__23 ^ 2 * r__3 ^ 4 + ((-2 * a__2 ^ 2 + 2 * b__3 ^ 2 + 2 * b__4 ^ 2 + 2 * r__2 ^ 2) * q__23 ^ 2 + 4 * b__3 ^ 2 * q__13 ^ 2 - 4 * q__13 ^ 2 * b__4 ^ 2) * r__3 ^ 2 + (a__2 ^ 2 + b__3 ^ 2 - b__4 ^ 2 + 2 * b__4 * r__2 - r__2 ^ 2) * (a__2 ^ 2 + b__3 ^ 2 - b__4 ^ 2 - 2 * b__4 * r__2 - r__2 ^ 2) * q__23 ^ 2 + 4 * q__13 ^ 2 * r__2 ^ 2 * (b__3 - b__4) * (b__3 + b__4)))) * ((c__r4 - 1) ^ 3) / s__r4 ^ 6 / (b__5 ^ 2);



%% Equations from maple for the 16-degree poly


e_0 = b__5 ^ 2 * (w__5 + w__7 + w__9 + v__1 + v__3 + v__5 + v__7 +...
    w__1 + w__3) * (w__5 + w__7 + w__9 - v__1 - v__3 - v__5 - v__7 +...
    w__1 + w__3) * s__r4 ^ 2 + (v__7 + v__1 + v__3 + v__5) ^ 2 *...
    (b__3 - r__2) ^ 2;

e_1 = (4 * (v__7 + v__1 + v__3 + v__5) * (v__6 + v__2 + v__4) * b__3 ^ 2)...
    - 0.8e1 * (((v__6 + v__2 + v__4) * r__2) - (r__1 * (v__7 + v__1 + v__3...
    + v__5)) / 0.2e1) * (v__7 + v__1 + v__3 + v__5) * b__3 + (4 * (v__7 +...
    v__1 + v__3 + v__5) * (v__6 + v__2 + v__4) * r__2 ^ 2) - (4 * r__1 *...
    (v__7 + v__1 + v__3 + v__5) ^ 2 * r__2) - (4 * ((v__6 + v__2 + v__4) *...
    v__1 + (v__6 + v__2 + v__4) * v__3 + (v__6 + v__2 + v__4) * v__5 +...
    (v__6 + v__2 + v__4) * v__7 - (w__2 + w__4 + w__6 + w__8) *...
    (w__1 + w__3 + w__5 + w__7 + w__9)) * b__5 ^ 2 * s__r4 ^ 2);

e_2 = (8 * v__7 ^ 2 + (4 * v__1 + 8 * v__3 + 12 * v__5) * v__7...
    - 4 * v__1 ^ 2 - 4 * v__1 * v__3 + 4 * v__3 * v__5 + 4 *...
    v__5 ^ 2 + 4 * (v__6 + v__2 + v__4) ^ 2) * b__3 ^ 2 +...
    ((-12 * v__7 ^ 2 + (-8 * v__3 - 16 * v__5) * v__7 +...
    12 * v__1 ^ 2 + (16 * v__3 + 8 * v__5) * v__1 + 4 * v__3 ^ 2 ...
    - 4 * v__5 ^ 2 - 8 * (v__6 + v__2 + v__4) ^ 2) * r__2 + ...
    16 * r__1 * (v__7 + v__1 + v__3 + v__5) * (v__6 + v__2 + v__4))...
    * b__3 + (4 * v__7 ^ 2 + (-4 * v__1 + 4 * v__5) * v__7 -...
    8 * v__1 ^ 2 + (-12 * v__3 - 8 * v__5) * v__1 - 4 * v__3 ^ 2 -...
    4 * v__3 * v__5 + 4 * (v__6 + v__2 + v__4) ^ 2) * r__2 ^ 2 -...
    16 * r__1 * (v__7 + v__1 + v__3 + v__5) * (v__6 + v__2 + v__4) * r__2...
    - 4 * (-v__1 * v__3 - v__1 ^ 2 + v__2 ^ 2 + v__6 ^ 2 - w__8 ^ 2 +...
    v__3 * v__5 - w__4 ^ 2 - w__6 ^ 2 + v__4 ^ 2 + w__3 ^ 2 - w__7 ^ 2 ...
    - 2 * w__9 ^ 2 + v__5 ^ 2 + 2 * v__7 ^ 2 + 2 * w__1 ^ 2 - w__2 ^ 2 +...
    (-w__7 - 2 * w__9) * w__5 + (-2 * w__4 - 2 * w__6 - 2 * w__8) * w__2...
    + (w__5 - w__9) * w__3 + (-2 * w__6 - 2 * w__8) * w__4 + (3 * w__3 +...
    2 * w__5 + w__7) * w__1 + (v__1 + 2 * v__3 + 3 * v__5) * v__7 - 2 *...
    w__6 * w__8 + 2 * v__6 * v__4 + (2 * v__6 + 2 * v__4) * v__2 - 3 * ...
    w__7 * w__9) * b__5 ^ 2 * s__r4 ^ 2 + 4 * r__1 ^ 2 * (v__7 + v__1 + v__3 + v__5) ^ 2;

e_3 = (16 * (v__7 + v__1 + v__3 + v__5) * (v__6 + v__2 + v__4) * r__1 ^ 2)...
    + (((16 * v__2 ^ 2) + ((32 * v__6 + 32 * v__4) * v__2) + (16 * v__4 ^ 2)...
    + (32 * v__6 * v__4) + (16 * v__6 ^ 2) + 0.28e2 * (v__7 - 0.5e1 / 0.7e1 * v__1...
    - v__3 / 0.7e1 + 0.3e1 / 0.7e1 * v__5) * (v__7 + v__1 + v__3 + v__5)) * b__3 -...
    0.16e2 * ((v__2 ^ 2) + ((2 * v__6 + 2 * v__4) * v__2) + (v__4 ^ 2) +...
    (2 * v__6 * v__4) + (v__6 ^ 2) + 0.5e1 / 0.4e1 * (v__7 - 0.7e1 / 0.5e1 *...
    v__1 - 0.3e1 / 0.5e1 * v__3 + v__5 / 0.5e1) * (v__7 + v__1 + v__3 + v__5))...
    * r__2) * r__1 + (((12 * v__7 - 12 * v__1 - 4 * v__3 + 4 * v__5) * v__2)...
    + ((20 * v__7 - 4 * v__1 + 4 * v__3 + 12 * v__5) * v__4) + 0.28e2 *...
    (v__7 + v__1 / 0.7e1 + 0.3e1 / 0.7e1 * v__3 + 0.5e1 / 0.7e1 * v__5) *...
    v__6) * b__3 ^ 2 - 0.40e2 * r__2 * ((v__7 / 0.5e1 - v__1 - 0.3e1 / 0.5e1...
    * v__3 - v__5 / 0.5e1) * v__2 + (0.3e1 / 0.5e1 * v__7 - 0.3e1 / 0.5e1 *...
    v__1 - v__3 / 0.5e1 + v__5 / 0.5e1) * v__4 + (v__7 - v__1 / 0.5e1 + ...
    v__3 / 0.5e1 + 0.3e1 / 0.5e1 * v__5) * v__6) * b__3 + (((-4 * v__7 -...
    28 * v__1 - 20 * v__3 - 12 * v__5) * v__2) + ((4 * v__7 - 20 * v__1 -...
    12 * v__3 - 4 * v__5) * v__4) + 0.12e2 * v__6 * (v__7 - v__1 - v__3 / 0.3e1...
    + v__5 / 0.3e1)) * r__2 ^ 2 - 0.28e2 * b__5 ^ 2 * ((-v__3 / 0.7e1 - ...
    0.3e1 / 0.7e1 * v__1 + v__5 / 0.7e1 + 0.3e1 / 0.7e1 * v__7) * v__2 +...
    (-v__1 / 0.7e1 + v__3 / 0.7e1 + 0.5e1 / 0.7e1 * v__7 + 0.3e1 / 0.7e1 * v__5)...
    * v__4 + (v__7 + v__1 / 0.7e1 + 0.3e1 / 0.7e1 * v__3 + 0.5e1 / 0.7e1 * v__5)...
    * v__6 + (0.5e1 / 0.7e1 * w__3 + 0.3e1 / 0.7e1 * w__5 + w__7 / 0.7e1 -...
    w__9 / 0.7e1 + w__1) * w__2 + (-0.3e1 / 0.7e1 * w__9 + 0.5e1 / 0.7e1 * w__1...
    + 0.3e1 / 0.7e1 * w__3 + w__5 / 0.7e1 - w__7 / 0.7e1) * w__4 + ...
    (-0.3e1 / 0.7e1 * w__7 - 0.5e1 / 0.7e1 * w__9 + 0.3e1 / 0.7e1 * w__1 +...
    w__3 / 0.7e1 - w__5 / 0.7e1) * w__6 + w__8 * (-0.5e1 * w__7 - 0.7e1 *...
    w__9 + w__1 - w__3 - 0.3e1 * w__5) / 0.7e1) * s__r4 ^ 2;

e_4 = -0.24e2 * (v__1 ^ 2 / 0.6e1 + (-v__5 / 0.3e1 - v__3 / 0.6e1 -...
    v__7 / 0.6e1) * v__1 + 0.7e1 / 0.6e1 * v__7 ^ 2 + (v__3 / 0.3e1 +...
    0.7e1 / 0.6e1 * v__5) * v__7 - v__3 ^ 2 / 0.6e1 - v__3 * v__5 / 0.6e1...
    + v__5 ^ 2 / 0.6e1 + v__6 ^ 2 + (0.2e1 / 0.3e1 * v__2 + 0.4e1 / 0.3e1 * v__4)...
    * v__6 - v__2 ^ 2 / 0.3e1 + v__4 ^ 2 / 0.3e1 - 0.7e1 / 0.6e1 * w__1 ^ 2 ...
    + (w__9 / 0.3e1 - 0.7e1 / 0.6e1 * w__3 - w__5 / 0.3e1 + w__7 / 0.6e1) * w__1 ...
    - w__3 ^ 2 / 0.6e1 + (w__7 / 0.3e1 + w__5 / 0.6e1 + w__9 / 0.6e1) * w__3 + ...
    w__5 ^ 2 / 0.6e1 + (w__7 / 0.6e1 - w__9 / 0.3e1) * w__5 - w__7 ^ 2 / 0.6e1 -...
    0.7e1 / 0.6e1 * w__7 * w__9 - 0.7e1 / 0.6e1 * w__9 ^ 2 + (w__2 + w__4 + w__6 + w__8) ...
    * (w__2 + w__4 / 0.3e1 - w__6 / 0.3e1 - w__8)) * b__5 ^ 2 * s__r4 ^ 2 + ...
    (0.4e1 * v__1 ^ 2 + (-0.4e1 * v__7 - 0.4e1 * v__3 - 0.8e1 * v__5) * v__1 + ...
    0.28e2 * v__7 ^ 2 + (0.8e1 * v__3 + 0.28e2 * v__5) * v__7 - 0.4e1 * v__3 ^ 2 ...
    - 0.4e1 * v__3 * v__5 + 0.4e1 * v__5 ^ 2 + 0.24e2 * (v__6 - v__2 / 0.3e1 + ...
    v__4 / 0.3e1) * (v__6 + v__2 + v__4)) * b__3 ^ 2 + ((-0.28e2 * v__1 ^ 2 + ...
    (0.16e2 * v__7 - 0.16e2 * v__3 + 0.8e1 * v__5) * v__1 - 0.28e2 * v__7 ^ 2 + ...
    (0.8e1 * v__3 - 0.16e2 * v__5) * v__7 + 0.4e1 * v__3 ^ 2 + 0.16e2 * v__3 * ...
    v__5 + 0.4e1 * v__5 ^ 2 - 0.32e2 * (v__6 - v__2) * (v__6 + v__2 + v__4)) * ...
    r__2 + 0.96e2 * ((-0.2e1 / 0.3e1 * v__2 - v__4 / 0.3e1) * v__1 + (v__6 + ...
    v__2 / 0.3e1 + 0.2e1 / 0.3e1 * v__4) * v__7 + (v__6 / 0.3e1 - v__2 / 0.3e1) ...
    * v__3 + 0.2e1 / 0.3e1 * (v__6 + v__4 / 0.2e1) * v__5) * r__1) * b__3 + ...
    (0.28e2 * v__1 ^ 2 + (-0.4e1 * v__7 + 0.28e2 * v__3 + 0.8e1 * v__5) * v__1 + ...
    0.4e1 * v__7 ^ 2 + (-0.8e1 * v__3 - 0.4e1 * v__5) * v__7 + 0.4e1 * v__3 ^ 2 -...
    0.4e1 * v__3 * v__5 - 0.4e1 * v__5 ^ 2 + 0.8e1 * (v__6 + v__2 + v__4) * (v__6 -...
    0.3e1 * v__2 - v__4)) * r__2 ^ 2 - 0.64e2 * r__1 * ((-v__6 / 0.2e1 - ...
    0.3e1 / 0.2e1 * v__2 - v__4) * v__1 + (v__6 + v__4 / 0.2e1) * v__7 + ...
    (-v__2 - v__4 / 0.2e1) * v__3 + v__5 * (v__6 - v__2) / 0.2e1) * r__2 + ...
    0.16e2 * (-0.3e1 / 0.2e1 * v__1 ^ 2 + (-0.2e1 * v__3 - v__5) * v__1 + ...
    0.3e1 / 0.2e1 * v__7 ^ 2 + (v__3 + 0.2e1 * v__5) * v__7 - v__3 ^ 2 / 0.2e1 + ...
    v__5 ^ 2 / 0.2e1 + (v__6 + v__2 + v__4) ^ 2) * r__1 ^ 2;

e_5 = (((16 * v__7 - 80 * v__1 - 48 * v__3 - 16 * v__5) * v__2) + ...
    ((48 * v__7 - 48 * v__1 - 16 * v__3 + 16 * v__5) * v__4) + ...
    0.80e2 * (v__7 - v__1 / 0.5e1 + v__3 / 0.5e1 + 0.3e1 / 0.5e1 * v__5) *...
    v__6) * r__1 ^ 2 + ((-(48 * v__2 ^ 2) + (0.32e2 * v__6 - (32 * v__4)) *...
    v__2 + (16 * v__4 ^ 2) + 0.96e2 * v__6 * v__4 + 0.80e2 * v__6 ^ 2 + ...
    (36 * v__1 ^ 2) + ((-24 * v__7 + 8 * v__3 - 24 * v__5) * v__1) - ...
    (12 * v__3 ^ 2) + ((8 * v__7 - 24 * v__5) * v__3) + (84 * v__7 ^ 2) + ...
    (72 * v__5 * v__7) + (4 * v__5 ^ 2)) * b__3 - 0.48e2 * r__2 * ...
    (-0.5e1 / 0.3e1 * (v__2 ^ 2) + (-0.2e1 / 0.3e1 * v__6 - (2 * v__4)) * ...
    v__2 - (v__4 ^ 2) / 0.3e1 + 0.2e1 / 0.3e1 * v__6 * v__4 + v__6 ^ 2 + ...
    0.7e1 / 0.4e1 * (v__1 ^ 2) + (-v__7 / 0.2e1 + 0.3e1 / 0.2e1 * v__3 + ...
    v__5 / 0.6e1) * v__1 + (v__3 ^ 2) / 0.12e2 + (-v__7 / 0.2e1 - v__5 / ...
    0.2e1) * v__3 + 0.3e1 / 0.4e1 * (v__7 ^ 2) + (v__5 * v__7) / 0.6e1 - ...
    (v__5 ^ 2) / 0.4e1)) * r__1 + (((4 * v__7 + 4 * v__1 - 12 * v__3 - ...
    12 * v__5) * v__2) + ((36 * v__7 - 12 * v__1 - 12 * v__3 + 4 * v__5) *...
    v__4) + 0.84e2 * (v__7 - v__1 / 0.7e1 + v__3 / 0.21e2 + 0.3e1 / 0.7e1 *...
    v__5) * v__6) * b__3 ^ 2 - 0.72e2 * ((-v__7 / 0.3e1 + v__1 + v__3 / ...
    0.9e1 - v__5 / 0.3e1) * v__2 + (v__7 / 0.9e1 + v__1 / 0.9e1 - v__3 / ...
    0.3e1 - v__5 / 0.3e1) * v__4 + v__6 * (v__7 - v__1 / 0.3e1 - v__3 / ...
    0.3e1 + v__5 / 0.9e1)) * r__2 * b__3 + (((-12 * v__7 + 84 * v__1 + ...
    36 * v__3 + 4 * v__5) * v__2) + ((-12 * v__7 + 36 * v__1 + 4 * v__3 - ...
    12 * v__5) * v__4) + 0.4e1 * v__6 * (v__7 + v__1 - 3 * v__3 - 3 * v__5))...
    * r__2 ^ 2 - 0.84e2 * ((-v__3 / 0.7e1 + v__1 / 0.21e2 - v__5 / 0.7e1 + ...
    v__7 / 0.21e2) * v__2 + (-v__1 / 0.7e1 - v__3 / 0.7e1 + 0.3e1 / 0.7e1 *...
    v__7 + v__5 / 0.21e2) * v__4 + (v__7 - v__1 / 0.7e1 + v__3 / 0.21e2 + ...
    0.3e1 / 0.7e1 * v__5) * v__6 + (-0.3e1 / 0.7e1 * w__3 - w__5 / 0.21e2 +...
    w__7 / 0.7e1 + w__9 / 0.7e1 - w__1) * w__2 + (-w__9 / 0.21e2 - 0.3e1 / ...
    0.7e1 * w__1 - w__3 / 0.21e2 + w__5 / 0.7e1 + w__7 / 0.7e1) * w__4 + ...
    (-w__7 / 0.21e2 - 0.3e1 / 0.7e1 * w__9 - w__1 / 0.21e2 + w__3 / 0.7e1 +...
    w__5 / 0.7e1) * w__6 + w__8 * (-0.3e1 * w__7 - 0.7e1 * w__9 + w__1 + ...
    w__3 - w__5 / 0.3e1) / 0.7e1) * b__5 ^ 2 * s__r4 ^ 2;

e_6 = ((56 * v__7 ^ 2 + (-12 * v__1 - 8 * v__3 + 28 * v__5) * v__7 + ...
    4 * v__1 ^ 2 + 12 * v__1 * v__3 - 4 * v__2 ^ 2 + (-8 * v__6 - 24 * ...
    v__4) * v__2 + 60 * v__6 ^ 2 + 40 * v__6 * v__4 - 12 * v__3 * v__5 ...
    - 4 * v__4 ^ 2 - 4 * v__5 ^ 2) * b__3 ^ 2) + (((-28 * v__7 ^ 2 + ...
    (24 * v__3 + 16 * v__5) * v__7 + 28 * v__1 ^ 2 + (-16 * v__3 - ...
    24 * v__5) * v__1 - 40 * v__2 ^ 2 + (48 * v__6 + 16 * v__4) * v__2 - ...
    40 * v__6 ^ 2 + 16 * v__6 * v__4 - 12 * v__3 ^ 2 + 24 * v__4 ^ 2 + 12 ...
    * v__5 ^ 2) * r__2) + 0.240e3 * ((v__6 - v__2 / 0.15e2 + v__4 / 0.3e1)...
    * v__7 + (-v__6 / 0.5e1 + v__2 / 0.3e1 - v__4 / 0.15e2) * v__1 + ...
    (-v__3 / 0.15e2 - v__5 / 0.5e1) * v__2 + (-v__6 / 0.15e2 - v__4 / 0.5e1) ...
    * v__3 + (v__6 - v__4 / 0.5e1) * v__5 / 0.3e1) * r__1) * b__3 + ...
    ((-4 * v__7 ^ 2 + (12 * v__1 - 12 * v__5) * v__7 - 56 * v__1 ^ 2 + ...
    (-28 * v__3 + 8 * v__5) * v__1 + 60 * v__2 ^ 2 + (-8 * v__6 + 40 * ...
    v__4) * v__2 - 4 * v__6 ^ 2 - 24 * v__6 * v__4 + 4 * v__3 ^ 2 + 12 * ...
    v__3 * v__5 - 4 * v__4 ^ 2) * r__2 ^ 2) - 0.80e2 * r__1 * ((v__6 - ...
    0.3e1 / 0.5e1 * v__2 - v__4 / 0.5e1) * v__7 + (-v__6 / 0.5e1 + ...
    (3 * v__2) + v__4) * v__1 + (v__3 - v__5 / 0.5e1) * v__2 + ...
    (-0.3e1 / 0.5e1 * v__6 - v__4 / 0.5e1) * v__3 - (v__5 * (v__6 + ...
    3 * v__4)) / 0.5e1) * r__2 + (60 * v__7 ^ 2 + (-24 * v__1 - 8 * ...
    v__3 + 40 * v__5) * v__7 + 60 * v__1 ^ 2 + (40 * v__3 - 8 * v__5) ...
    * v__1 + 64 * v__6 ^ 2 + 64 * v__6 * v__4 - 64 * v__2 ^ 2 - ...
    64 * v__2 * v__4 - 4 * v__3 ^ 2 - 24 * v__3 * v__5 - 4 * v__5 ^ 2)...
    * r__1 ^ 2 - 0.60e2 * b__5 ^ 2 * ((v__1 * v__3) / 0.5e1 + ...
    (v__1 ^ 2) / 0.15e2 - (v__2 ^ 2) / 0.15e2 + (v__6 ^ 2) - ...
    w__8 ^ 2 + (0.2e1 / 0.5e1 * w__6 + 0.2e1 / 0.15e2 * w__8) * w__4 + ...
    (w__7 / 0.5e1 + 0.2e1 / 0.15e2 * w__9) * w__5 + (-0.2e1 / 0.3e1 * w__4 + ...
    0.2e1 / 0.15e2 * w__6 + 0.2e1 / 0.5e1 * w__8) * w__2 + ...
    (-w__5 / 0.5e1 + w__9 / 0.5e1) * w__3 + (0.7e1 / 0.15e2 * w__3 - ...
    0.2e1 / 0.15e2 * w__5 - w__7 / 0.5e1) * w__1 + ...
    (-0.2e1 / 0.15e2 * v__6 - 0.2e1 / 0.5e1 * v__4) * v__2 + ...
    (-0.2e1 / 0.15e2 * v__3 - v__1 / 0.5e1 + 0.7e1 / 0.15e2 * v__5) * ...
    v__7 - (v__3 * v__5) / 0.5e1 + w__4 ^ 2 / 0.15e2 + w__6 ^ 2 / 0.15e2 - ...
    (v__4 ^ 2) / 0.15e2 - w__3 ^ 2 / 0.15e2 + w__7 ^ 2 / 0.15e2 -...
    0.14e2 / 0.15e2 * w__9 ^ 2 - (v__5 ^ 2) / 0.15e2 + 0.14e2 / 0.15e2...
    * (v__7 ^ 2) + 0.14e2 / 0.15e2 * w__1 ^ 2 - w__2 ^ 2 - 0.2e1 / 0.3e1 ...
    * w__6 * w__8 + 0.2e1 / 0.3e1 * v__6 * v__4 - 0.7e1 / 0.15e2 * w__7 * w__9) * s__r4 ^ 2;

e_7 = (((-32 * v__7 + 160 * v__1 + 32 * v__3 - 32 * v__5) * v__2) + ...
    ((32 * v__7 + 32 * v__1 - 32 * v__3 - 32 * v__5) * v__4) + ...
    0.160e3 * (v__7 - v__1 / 0.5e1 - v__3 / 0.5e1 + v__5 / 0.5e1) * v__6) * r__1 ^ 2 + ...
    (((32 * v__2 ^ 2) + (-0.64e2 * v__6 - (64 * v__4)) * v__2 - ...
    (32 * v__4 ^ 2) + 0.64e2 * v__6 * v__4 + 0.160e3 * v__6 ^ 2 - ...
    (20 * v__1 ^ 2) + ((-24 * v__7 + 40 * v__3 + 24 * v__5) * v__1) + ...
    (12 * v__3 ^ 2) + ((-40 * v__7 - 24 * v__5) * v__3) + (140 * v__7 ^ 2) ...
    + (40 * v__5 * v__7) - (20 * v__5 ^ 2)) * b__3 - 0.32e2 * ((5 * v__2 ^ 2) ...
    + (-0.2e1 * v__6 + (2 * v__4)) * v__2 - (v__4 ^ 2) - 0.2e1 * v__6 * v__4 ...
    + v__6 ^ 2 - 0.35e2 / 0.8e1 * (v__1 ^ 2) + (0.3e1 / 0.4e1 * v__7 - ...
    0.5e1 / 0.4e1 * v__3 + 0.5e1 / 0.4e1 * v__5) * v__1 + 0.5e1 / 0.8e1 * ...
    (v__3 ^ 2) + (-0.3e1 / 0.4e1 * v__7 + 0.3e1 / 0.4e1 * v__5) * v__3 + ...
    0.5e1 / 0.8e1 * (v__7 ^ 2) - 0.5e1 / 0.4e1 * v__5 * v__7 - ...
    0.3e1 / 0.8e1 * (v__5 ^ 2)) * r__2) * r__1 + (((-20 * v__7 + 20 * v__1 ...
    + 12 * v__3 - 12 * v__5) * v__2) + ((20 * v__7 + 12 * v__1 - 12 * v__3 - 20 * v__5) * v__4) ...
    + 0.140e3 * (v__7 - 0.3e1 / 0.35e2 * v__1 - v__3 / 0.7e1 + ...
    v__5 / 0.7e1) * v__6) * b__3 ^ 2 - 0.40e2 * ((-0.3e1 / 0.5e1 * v__7 - ...
    v__1 + v__3 + 0.3e1 / 0.5e1 * v__5) * v__2 + (-v__7 + v__1 + ...
    0.3e1 / 0.5e1 * v__3 - 0.3e1 / 0.5e1 * v__5) * v__4 + v__6 * (v__7 ...
    + 0.3e1 / 0.5e1 * v__1 - 0.3e1 / 0.5e1 * v__3 - v__5)) * r__2 * b__3 + ...
    (((12 * v__7 - 140 * v__1 - 20 * v__3 + 20 * v__5) * v__2) + ((-12 * v__7 - ...
    20 * v__1 + 20 * v__3 + 12 * v__5) * v__4) - 0.20e2 * v__6 * (v__7 - v__1 - ...
    0.3e1 / 0.5e1 * v__3 + 0.3e1 / 0.5e1 * v__5)) * r__2 ^ 2 - ...
    0.140e3 * b__5 ^ 2 * s__r4 ^ 2 * ((0.3e1 / 0.35e2 * v__3 + v__1 / 0.7e1 - ...
    0.3e1 / 0.35e2 * v__5 - v__7 / 0.7e1) * v__2 + (0.3e1 / 0.35e2 * v__1 - ...
    0.3e1 / 0.35e2 * v__3 + v__7 / 0.7e1 - v__5 / 0.7e1) * v__4 + (v__7 - 0.3e1 / 0.35e2 * v__1 -...
    v__3 / 0.7e1 + v__5 / 0.7e1) * v__6 + (w__3 / 0.7e1 - w__5 / 0.7e1 - 0.3e1 / 0.35e2 * w__7 +...
    0.3e1 / 0.35e2 * w__9 + w__1) * w__2 + (w__9 / 0.7e1 + w__1 / 0.7e1 - w__3 / 0.7e1 - ...
    0.3e1 / 0.35e2 * w__5 + 0.3e1 / 0.35e2 * w__7) * w__4 + (w__7 / 0.7e1 - w__9 / 0.7e1 - ...
    w__1 / 0.7e1 - 0.3e1 / 0.35e2 * w__3 + 0.3e1 / 0.35e2 * w__5) * w__6 - ...
    0.3e1 / 0.35e2 * w__8 * (0.5e1 / 0.3e1 * w__7 + 0.35e2 / 0.3e1 * w__9 + ...
    w__1 - w__3 - 0.5e1 / 0.3e1 * w__5));

e_8 = -0.80e2 * b__5 ^ 2 * (-v__1 ^ 2 / 0.8e1 + 0.3e1 / 0.20e2 * v__1 * v__5 + ...
    v__2 ^ 2 / 0.5e1 - 0.2e1 / 0.5e1 * v__2 * v__6 + 0.3e1 / 0.40e2 * v__3 ^ 2 - ...
    v__3 * v__7 / 0.4e1 - v__5 ^ 2 / 0.8e1 + v__6 ^ 2 + 0.7e1 / 0.8e1 * ...
    v__7 ^ 2 - v__4 ^ 2 / 0.5e1 - 0.7e1 / 0.8e1 * w__1 ^ 2 + (-0.3e1 / 0.20e2 * w__9 + ...
    w__5 / 0.4e1) * w__1 - 0.3e1 / 0.40e2 * w__5 ^ 2 - 0.7e1 / 0.8e1 * w__9 ^ 2 + ...
    w__6 ^ 2 / 0.5e1 + w__3 ^ 2 / 0.8e1 + w__2 ^ 2 - 0.3e1 / 0.20e2 * w__3 * w__7 - ...
    0.2e1 / 0.5e1 * w__2 * w__6 + 0.2e1 / 0.5e1 * w__4 * w__8 + w__5 * w__9 / 0.4e1 + ...
    w__7 ^ 2 / 0.8e1 - w__8 ^ 2 - w__4 ^ 2 / 0.5e1) * s__r4 ^ 2 + (-0.10e2 * v__1 ^ 2 + ...
    0.12e2 * v__1 * v__5 + 0.16e2 * v__2 ^ 2 - 0.32e2 * v__2 * v__6 + 0.6e1 * v__3 ^ 2 -...
    0.20e2 * v__3 * v__7 - 0.16e2 * v__4 ^ 2 - 0.10e2 * v__5 ^ 2 + 0.80e2 * v__6 ^ 2 + ...
    0.70e2 * v__7 ^ 2) * b__3 ^ 2 + ((0.64e2 * v__1 * v__4 + (-0.64e2 * v__7 + ...
    0.64e2 * v__3) * v__2 + 0.320e3 * v__7 * v__6 - 0.64e2 * v__3 * v__6 - ...
    0.64e2 * v__4 * v__5) * r__1 + 0.64e2 * ((-0.3e1 / 0.8e1 * v__7 + ...
    0.5e1 / 0.8e1 * v__3) * v__1 + v__6 * v__4 + 0.5e1 / 0.8e1 * v__5 * v__7 - ...
    v__2 * v__4 - 0.3e1 / 0.8e1 * v__3 * v__5) * r__2) * b__3 + (-0.80e2 * v__1 ^ 2 + ...
    0.32e2 * v__1 * v__5 + 0.96e2 * v__2 ^ 2 - 0.64e2 * v__2 * v__6 + ...
    0.16e2 * v__3 ^ 2 - 0.32e2 * v__3 * v__7 - 0.32e2 * v__4 ^ 2 - 0.16e2 * v__5 ^ 2 + ...
    0.96e2 * v__6 ^ 2 + 0.80e2 * v__7 ^ 2) * r__1 ^ 2 - ...
    0.64e2 * ((v__6 - 0.5e1 * v__2) * v__1 - v__5 * v__6 - v__4 * v__7 + ...
    v__2 * v__5 + v__3 * v__4) * r__2 * r__1 - 0.16e2 * (v__6 ^ 2 - ...
    0.2e1 * v__2 * v__6 + 0.5e1 / 0.8e1 * v__7 ^ 2 - ...
    0.3e1 / 0.4e1 * v__3 * v__7 - 0.35e2 / 0.8e1 * v__1 ^ 2 + ...
    0.5e1 / 0.4e1 * v__1 * v__5 + 0.5e1 * v__2 ^ 2 + 0.5e1 / 0.8e1 * v__3 ^ 2 - ...
    v__4 ^ 2 - 0.3e1 / 0.8e1 * v__5 ^ 2) * r__2 ^ 2;

e_9 = (((-32 * v__7 - 160 * v__1 + 32 * v__3 + 32 * v__5) * v__2) + ...
    ((-32 * v__7 + 32 * v__1 + 32 * v__3 - 32 * v__5) * v__4) + ...
    0.160e3 * v__6 * (v__7 + v__1 / 0.5e1 - v__3 / 0.5e1 - v__5 / 0.5e1)) * r__1 ^ 2 + ...
    (((32 * v__2 ^ 2) + (-0.64e2 * v__6 + (64 * v__4)) * v__2 - (32 * v__4 ^ 2) - ...
    0.64e2 * v__6 * v__4 + 0.160e3 * v__6 ^ 2 - (20 * v__1 ^ 2) + ...
    ((24 * v__7 - 40 * v__3 + 24 * v__5) * v__1) + (12 * v__3 ^ 2) + ...
    ((-40 * v__7 + 24 * v__5) * v__3) + (140 * v__7 ^ 2) - (40 * v__5 * v__7) - ...
    (20 * v__5 ^ 2)) * b__3 + 0.32e2 * r__2 * ((5 * v__2 ^ 2) + (-0.2e1 * v__6 - ...
    (2 * v__4)) * v__2 - (v__4 ^ 2) + 0.2e1 * v__6 * v__4 + v__6 ^ 2 - ...
    0.35e2 / 0.8e1 * (v__1 ^ 2) + (-0.3e1 / 0.4e1 * v__7 + 0.5e1 / 0.4e1 * v__3 + ...
    0.5e1 / 0.4e1 * v__5) * v__1 + 0.5e1 / 0.8e1 * (v__3 ^ 2) + (-0.3e1 / 0.4e1 * v__7 - ...
    0.3e1 / 0.4e1 * v__5) * v__3 + 0.5e1 / 0.8e1 * (v__7 ^ 2) + 0.5e1 / 0.4e1 * v__5 * v__7 - ...
    0.3e1 / 0.8e1 * (v__5 ^ 2))) * r__1 + (((-20 * v__7 - 20 * v__1 + 12 * v__3 + 12 * v__5) *...
    v__2) + ((-20 * v__7 + 12 * v__1 + 12 * v__3 - 20 * v__5) * v__4) + ...
    0.140e3 * v__6 * (v__7 + 0.3e1 / 0.35e2 * v__1 - v__3 / 0.7e1 - ...
    v__5 / 0.7e1)) * b__3 ^ 2 + 0.40e2 * ((-0.3e1 / 0.5e1 * v__7 + v__1 + ...
    v__3 - 0.3e1 / 0.5e1 * v__5) * v__2 + (v__7 + v__1 - 0.3e1 / 0.5e1 * ...
    v__3 - 0.3e1 / 0.5e1 * v__5) * v__4 + v__6 * (v__7 - 0.3e1 / 0.5e1 * ...
    v__1 - 0.3e1 / 0.5e1 * v__3 + v__5)) * r__2 * b__3 + (((12 * v__7 + ...
    140 * v__1 - 20 * v__3 - 20 * v__5) * v__2) + ((12 * v__7 - 20 * v__1 -...
    20 * v__3 + 12 * v__5) * v__4) - 0.20e2 * v__6 * (v__7 + v__1 - 0.3e1 /...
    0.5e1 * v__3 - 0.3e1 / 0.5e1 * v__5)) * r__2 ^ 2 - 0.140e3 * b__5 ^ 2 *...
    ((0.3e1 / 0.35e2 * v__3 - v__1 / 0.7e1 + 0.3e1 / 0.35e2 * v__5 - v__7 /...
    0.7e1) * v__2 + (0.3e1 / 0.35e2 * v__1 + 0.3e1 / 0.35e2 * v__3 - v__7 /...
    0.7e1 - v__5 / 0.7e1) * v__4 + v__6 * (v__7 + 0.3e1 / 0.35e2 * v__1 - ...
    v__3 / 0.7e1 - v__5 / 0.7e1) + (w__3 / 0.7e1 + w__5 / 0.7e1 - 0.3e1 / ...
    0.35e2 * w__7 - 0.3e1 / 0.35e2 * w__9 - w__1) * w__2 + (w__9 / 0.7e1 + ...
    w__1 / 0.7e1 + w__3 / 0.7e1 - 0.3e1 / 0.35e2 * w__5 - 0.3e1 / 0.35e2 * ...
    w__7) * w__4 + (w__7 / 0.7e1 + w__9 / 0.7e1 + w__1 / 0.7e1 - 0.3e1 / ...
    0.35e2 * w__3 - 0.3e1 / 0.35e2 * w__5) * w__6 - 0.3e1 / 0.35e2 * w__8 * ...
    (-0.5e1 / 0.3e1 * w__7 + 0.35e2 / 0.3e1 * w__9 + w__1 + w__3 - ...
    0.5e1 / 0.3e1 * w__5)) * s__r4 ^ 2;

e_10 = ((56 * v__7 ^ 2 + (12 * v__1 - 8 * v__3 - 28 * v__5) * v__7 + ...
    4 * v__1 ^ 2 - 12 * v__1 * v__3 - 4 * v__2 ^ 2 + (-8 * v__6 + 24 * v__4)...
    * v__2 + 60 * v__6 ^ 2 - 40 * v__6 * v__4 + 12 * v__3 * v__5 - 4 * ...
    v__4 ^ 2 - 4 * v__5 ^ 2) * b__3 ^ 2) + (((28 * v__7 ^ 2 + ...
    (-24 * v__3 + 16 * v__5) * v__7 - 28 * v__1 ^ 2 + (-16 * v__3 + ...
    24 * v__5) * v__1 + 40 * v__2 ^ 2 + (-48 * v__6 + 16 * v__4) * ...
    v__2 + 40 * v__6 ^ 2 + 16 * v__6 * v__4 + 12 * v__3 ^ 2 - 24 * ...
    v__4 ^ 2 - 12 * v__5 ^ 2) * r__2) + 0.240e3 * ((v__6 - v__2 / 0.15e2 -...
    v__4 / 0.3e1) * v__7 + (v__6 / 0.5e1 - v__2 / 0.3e1 - v__4 / 0.15e2) *...
    v__1 + (-v__3 / 0.15e2 + v__5 / 0.5e1) * v__2 + (-v__6 / 0.15e2 + v__4 / 0.5e1)...
    * v__3 - (v__6 + v__4 / 0.5e1) * v__5 / 0.3e1) * r__1) * b__3 + ...
    ((-4 * v__7 ^ 2 + (-12 * v__1 + 12 * v__5) * v__7 - 56 * v__1 ^ 2 + ...
    (28 * v__3 + 8 * v__5) * v__1 + 60 * v__2 ^ 2 + (-8 * v__6 - 40 * v__4) *...
    v__2 - 4 * v__6 ^ 2 + 24 * v__6 * v__4 + 4 * v__3 ^ 2 - 12 * v__3 * v__5 - ...
    4 * v__4 ^ 2) * r__2 ^ 2) + 0.80e2 * ((v__6 - 0.3e1 / 0.5e1 * v__2 + ...
    v__4 / 0.5e1) * v__7 + (v__6 / 0.5e1 - (3 * v__2) + v__4) * v__1 + ...
    (v__3 + v__5 / 0.5e1) * v__2 + (-0.3e1 / 0.5e1 * v__6 + v__4 / 0.5e1) * ...
    v__3 + (v__5 * (v__6 - 3 * v__4)) / 0.5e1) * r__1 * r__2 + (60 * v__7 ^ ...
    2 + (24 * v__1 - 8 * v__3 - 40 * v__5) * v__7 + 60 * v__1 ^ 2 + (-40 * ...
    v__3 - 8 * v__5) * v__1 + 64 * v__6 ^ 2 - 64 * v__6 * v__4 - 64 * v__2 ^ 2 ...
    + 64 * v__2 * v__4 - 4 * v__3 ^ 2 + 24 * v__3 * v__5 - 4 * v__5 ^ 2) * r__1 ^ 2 ...
    - 0.60e2 * b__5 ^ 2 * s__r4 ^ 2 * (-(v__1 * v__3) / 0.5e1 + (v__1 ^ 2) / 0.15e2 - ...
    (v__2 ^ 2) / 0.15e2 + (v__6 ^ 2) - w__8 ^ 2 + (v__3 * v__5) / 0.5e1 + w__4 ^ 2 / 0.15e2 +...
    w__6 ^ 2 / 0.15e2 - (v__4 ^ 2) / 0.15e2 - w__3 ^ 2 / 0.15e2 + w__7 ^ 2 / 0.15e2 - ...
    0.14e2 / 0.15e2 * w__9 ^ 2 - (v__5 ^ 2) / 0.15e2 + 0.14e2 / 0.15e2 * (v__7 ^ 2) + ...
    0.14e2 / 0.15e2 * w__1 ^ 2 - w__2 ^ 2 + (w__5 / 0.5e1 - w__9 / 0.5e1) * w__3 + ...
    (-0.2e1 / 0.5e1 * w__6 + 0.2e1 / 0.15e2 * w__8) * w__4 + (-w__7 / 0.5e1 + ...
    0.2e1 / 0.15e2 * w__9) * w__5 + (-0.7e1 / 0.15e2 * w__3 - 0.2e1 / 0.15e2 * w__5 + ...
    w__7 / 0.5e1) * w__1 + (0.2e1 / 0.3e1 * w__4 + 0.2e1 / 0.15e2 * w__6 - ...
    0.2e1 / 0.5e1 * w__8) * w__2 + (-0.2e1 / 0.15e2 * v__6 + 0.2e1 / 0.5e1 * v__4)...
    * v__2 + (-0.2e1 / 0.15e2 * v__3 + v__1 / 0.5e1 - 0.7e1 / 0.15e2 * v__5) * v__7 +...
    0.2e1 / 0.3e1 * w__6 * w__8 - 0.2e1 / 0.3e1 * v__6 * v__4 + 0.7e1 / 0.15e2 * w__7 * w__9);

e_11 = (((16 * v__7 + 80 * v__1 - 48 * v__3 + 16 * v__5) * v__2) + ...
    ((-48 * v__7 - 48 * v__1 + 16 * v__3 + 16 * v__5) * v__4) + ...
    0.80e2 * v__6 * (v__7 + v__1 / 0.5e1 + v__3 / 0.5e1 - ...
    0.3e1 / 0.5e1 * v__5)) * r__1 ^ 2 + ((-(48 * v__2 ^ 2) + ...
    (0.32e2 * v__6 + (32 * v__4)) * v__2 + (16 * v__4 ^ 2) - ...
    0.96e2 * v__6 * v__4 + 0.80e2 * v__6 ^ 2 + (36 * v__1 ^ 2) + ...
    ((24 * v__7 - 8 * v__3 - 24 * v__5) * v__1) - (12 * v__3 ^ 2) + ...
    ((8 * v__7 + 24 * v__5) * v__3) + (84 * v__7 ^ 2) - (72 * v__5 * v__7) ...
    + (4 * v__5 ^ 2)) * b__3 + 0.48e2 * (-0.5e1 / 0.3e1 * (v__2 ^ 2) + ...
    (-0.2e1 / 0.3e1 * v__6 + (2 * v__4)) * v__2 - (v__4 ^ 2) / 0.3e1 - ...
    0.2e1 / 0.3e1 * v__6 * v__4 + v__6 ^ 2 + 0.7e1 / 0.4e1 * (v__1 ^ 2) + ...
    (v__7 / 0.2e1 - 0.3e1 / 0.2e1 * v__3 + v__5 / 0.6e1) * v__1 + ...
    (v__3 ^ 2) / 0.12e2 + (-v__7 / 0.2e1 + v__5 / 0.2e1) * v__3 + ...
    0.3e1 / 0.4e1 * (v__7 ^ 2) - (v__5 * v__7) / 0.6e1 - ...
    (v__5 ^ 2) / 0.4e1) * r__2) * r__1 + (((4 * v__7 - 4 * v__1 - ...
    12 * v__3 + 12 * v__5) * v__2) + ((-36 * v__7 - 12 * v__1 + ...
    12 * v__3 + 4 * v__5) * v__4) + 0.84e2 * v__6 * (v__7 + v__1 / 0.7e1 + ...
    v__3 / 0.21e2 - 0.3e1 / 0.7e1 * v__5)) * b__3 ^ 2 + 0.72e2 * r__2 * ...
    ((-v__7 / 0.3e1 - v__1 + v__3 / 0.9e1 + v__5 / 0.3e1) * v__2 + ...
    (-v__7 / 0.9e1 + v__1 / 0.9e1 + v__3 / 0.3e1 - v__5 / 0.3e1) * v__4 + ...
    v__6 * (v__7 + v__1 / 0.3e1 - v__3 / 0.3e1 - v__5 / 0.9e1)) * b__3 + ...
    (((-12 * v__7 - 84 * v__1 + 36 * v__3 - 4 * v__5) * v__2) + ((12 * v__7 + ...
    36 * v__1 - 4 * v__3 - 12 * v__5) * v__4) + 0.4e1 * v__6 * (v__7 - v__1 - ...
    3 * v__3 + 3 * v__5)) * r__2 ^ 2 - 0.84e2 * b__5 ^ 2 * s__r4 ^ 2 * ...
    ((-v__3 / 0.7e1 - v__1 / 0.21e2 + v__5 / 0.7e1 + v__7 / 0.21e2) * v__2 + ...
    (-v__1 / 0.7e1 + v__3 / 0.7e1 - 0.3e1 / 0.7e1 * v__7 + v__5 / 0.21e2) * v__4 + ...
    v__6 * (v__7 + v__1 / 0.7e1 + v__3 / 0.21e2 - 0.3e1 / 0.7e1 * v__5) + ...
    (-0.3e1 / 0.7e1 * w__3 + w__5 / 0.21e2 + w__7 / 0.7e1 - w__9 / 0.7e1 + w__1) ...
    * w__2 + (-w__9 / 0.21e2 - 0.3e1 / 0.7e1 * w__1 + w__3 / 0.21e2 + w__5 / 0.7e1 -...
    w__7 / 0.7e1) * w__4 + (-w__7 / 0.21e2 + 0.3e1 / 0.7e1 * w__9 + w__1 / 0.21e2 + ...
    w__3 / 0.7e1 - w__5 / 0.7e1) * w__6 + w__8 * (0.3e1 * w__7 - 0.7e1 * w__9 + ...
    w__1 - w__3 - w__5 / 0.3e1) / 0.7e1);

e_12 = -0.24e2 * (v__1 ^ 2 / 0.6e1 + (-v__5 / 0.3e1 + v__3 / 0.6e1 + ...
    v__7 / 0.6e1) * v__1 + 0.7e1 / 0.6e1 * v__7 ^ 2 + (v__3 / 0.3e1 - ...
    0.7e1 / 0.6e1 * v__5) * v__7 - v__3 ^ 2 / 0.6e1 + v__3 * v__5 / 0.6e1 + ...
    v__5 ^ 2 / 0.6e1 + v__6 ^ 2 + (0.2e1 / 0.3e1 * v__2 - 0.4e1 / 0.3e1 * v__4) *...
    v__6 - v__2 ^ 2 / 0.3e1 + v__4 ^ 2 / 0.3e1 - 0.7e1 / 0.6e1 * w__1 ^ 2 + ...
    (w__9 / 0.3e1 + 0.7e1 / 0.6e1 * w__3 - w__5 / 0.3e1 - w__7 / 0.6e1) * w__1 -...
    w__3 ^ 2 / 0.6e1 + (w__7 / 0.3e1 - w__5 / 0.6e1 - w__9 / 0.6e1) * w__3 +...
    w__5 ^ 2 / 0.6e1 + (-w__7 / 0.6e1 - w__9 / 0.3e1) * w__5 - w__7 ^ 2 / ...
    0.6e1 + 0.7e1 / 0.6e1 * w__7 * w__9 - 0.7e1 / 0.6e1 * w__9 ^ 2 + (w__2 - ...
    w__4 / 0.3e1 - w__6 / 0.3e1 + w__8) * (w__2 - w__4 + w__6 - w__8)) * ...
    b__5 ^ 2 * s__r4 ^ 2 + (0.4e1 * v__1 ^ 2 + (0.4e1 * v__7 + 0.4e1 * v__3 ...
    - 0.8e1 * v__5) * v__1 + 0.28e2 * v__7 ^ 2 + (0.8e1 * v__3 - 0.28e2 * v__5) ...
    * v__7 - 0.4e1 * v__3 ^ 2 + 0.4e1 * v__3 * v__5 + 0.4e1 * v__5 ^ 2 + 0.24e2 *...
    (v__6 + v__2 - v__4) * (v__6 - v__2 / 0.3e1 - v__4 / 0.3e1)) * b__3 ^ 2 + ...
    ((0.28e2 * v__1 ^ 2 + (0.16e2 * v__7 - 0.16e2 * v__3 - 0.8e1 * v__5) * v__1...
    + 0.28e2 * v__7 ^ 2 + (-0.8e1 * v__3 - 0.16e2 * v__5) * v__7 - 0.4e1 * ...
    v__3 ^ 2 + 0.16e2 * v__3 * v__5 - 0.4e1 * v__5 ^ 2 + 0.32e2 * (v__6 - ...
    v__2) * (v__6 + v__2 - v__4)) * r__2 + 0.96e2 * ((0.2e1 / 0.3e1 * v__2 -...
    v__4 / 0.3e1) * v__1 + (v__6 + v__2 / 0.3e1 - 0.2e1 / 0.3e1 * v__4) * ...
    v__7 + (v__6 / 0.3e1 - v__2 / 0.3e1) * v__3 - 0.2e1 / 0.3e1 * (v__6 - ...
    v__4 / 0.2e1) * v__5) * r__1) * b__3 + (0.28e2 * v__1 ^ 2 + (0.4e1 * ...
    v__7 - 0.28e2 * v__3 + 0.8e1 * v__5) * v__1 + 0.4e1 * v__7 ^ 2 + ...
    (-0.8e1 * v__3 + 0.4e1 * v__5) * v__7 + 0.4e1 * v__3 ^ 2 + 0.4e1 * ...
    v__3 * v__5 - 0.4e1 * v__5 ^ 2 + 0.8e1 * (v__6 + v__2 - v__4) * ...
    (v__6 - 0.3e1 * v__2 + v__4)) * r__2 ^ 2 + 0.64e2 * r__1 * ...
    ((v__6 / 0.2e1 + 0.3e1 / 0.2e1 * v__2 - v__4) * v__1 + (v__6 ...
    - v__4 / 0.2e1) * v__7 + (-v__2 + v__4 / 0.2e1) * v__3 - v__5 *...
    (v__6 - v__2) / 0.2e1) * r__2 + 0.16e2 * (-0.3e1 / 0.2e1 * v__1 ^ 2 ...
    + (0.2e1 * v__3 - v__5) * v__1 + 0.3e1 / 0.2e1 * v__7 ^ 2 + (v__3 - ...
    0.2e1 * v__5) * v__7 - v__3 ^ 2 / 0.2e1 + v__5 ^ 2 / 0.2e1 + (v__6 + ...
    v__2 - v__4) ^ 2) * r__1 ^ 2;

e_13 = (16 * (v__7 - v__1 + v__3 - v__5) * (v__6 + v__2 - v__4) * r__1 ^ 2)...
    + (((16 * v__2 ^ 2) + ((32 * v__6 - 32 * v__4) * v__2) + (16 * v__4 ^ 2)...
    - (32 * v__6 * v__4) + (16 * v__6 ^ 2) + 0.28e2 * (v__7 - v__1 + v__3 - ...
    v__5) * (v__7 + 0.5e1 / 0.7e1 * v__1 - v__3 / 0.7e1 - 0.3e1 / 0.7e1 * v__5))...
    * b__3 + 0.16e2 * ((v__2 ^ 2) + ((2 * v__6 - 2 * v__4) * v__2) + (v__4 ^ 2) ...
    - (2 * v__6 * v__4) + (v__6 ^ 2) + 0.5e1 / 0.4e1 * (v__7 - v__1 + v__3 - v__5)...
    * (v__7 + 0.7e1 / 0.5e1 * v__1 - 0.3e1 / 0.5e1 * v__3 - v__5 / 0.5e1)) * r__2)...
    * r__1 + (((12 * v__7 + 12 * v__1 - 4 * v__3 - 4 * v__5) * v__2) + ((-20 * v__7 ...
    - 4 * v__1 - 4 * v__3 + 12 * v__5) * v__4) + 0.28e2 * v__6 * (v__7 - v__1 / 0.7e1...
    + 0.3e1 / 0.7e1 * v__3 - 0.5e1 / 0.7e1 * v__5)) * b__3 ^ 2 + 0.40e2 * r__2 * ...
    ((v__7 / 0.5e1 + v__1 - 0.3e1 / 0.5e1 * v__3 + v__5 / 0.5e1) * v__2 + (-0.3e1 /...
    0.5e1 * v__7 - 0.3e1 / 0.5e1 * v__1 + v__3 / 0.5e1 + v__5 / 0.5e1) * v__4 + v__6 ...
    * (v__7 + v__1 / 0.5e1 + v__3 / 0.5e1 - 0.3e1 / 0.5e1 * v__5)) * b__3 + (((-4 * ...
    v__7 + 28 * v__1 - 20 * v__3 + 12 * v__5) * v__2) + ((-4 * v__7 - 20 * v__1 + ...
    12 * v__3 - 4 * v__5) * v__4) + 0.12e2 * v__6 * (v__7 + v__1 - v__3 / 0.3e1 - ...
    v__5 / 0.3e1)) * r__2 ^ 2 - 0.28e2 * b__5 ^ 2 * ((-v__3 / 0.7e1 + 0.3e1 / ...
    0.7e1 * v__1 - v__5 / 0.7e1 + 0.3e1 / 0.7e1 * v__7) * v__2 + (-v__1 / 0.7e1...
    - v__3 / 0.7e1 - 0.5e1 / 0.7e1 * v__7 + 0.3e1 / 0.7e1 * v__5) * v__4 + v__6 ...
    * (v__7 - v__1 / 0.7e1 + 0.3e1 / 0.7e1 * v__3 - 0.5e1 / 0.7e1 * v__5) + ...
    (0.5e1 / 0.7e1 * w__3 - 0.3e1 / 0.7e1 * w__5 + w__7 / 0.7e1 + w__9 / 0.7e1 -...
    w__1) * w__2 + (-0.3e1 / 0.7e1 * w__9 + 0.5e1 / 0.7e1 * w__1 - 0.3e1 / ...
    0.7e1 * w__3 + w__5 / 0.7e1 + w__7 / 0.7e1) * w__4 + (-0.3e1 / 0.7e1 * ...
    w__7 + 0.5e1 / 0.7e1 * w__9 - 0.3e1 / 0.7e1 * w__1 + w__3 / 0.7e1 + ...
    w__5 / 0.7e1) * w__6 + w__8 * (0.5e1 * w__7 - 0.7e1 * w__9 + w__1 + ...
    w__3 - 0.3e1 * w__5) / 0.7e1) * s__r4 ^ 2;

e_14 = (8 * v__7 ^ 2 + (-4 * v__1 + 8 * v__3 - 12 * v__5) * v__7 - ...
    4 * v__1 ^ 2 + 4 * v__1 * v__3 - 4 * v__3 * v__5 + 4 * v__5 ^ 2 +...
    4 * (v__6 + v__2 - v__4) ^ 2) * b__3 ^ 2 + ((12 * v__7 ^ 2 + ...
    (8 * v__3 - 16 * v__5) * v__7 - 12 * v__1 ^ 2 + (16 * v__3 - ...
    8 * v__5) * v__1 - 4 * v__3 ^ 2 + 4 * v__5 ^ 2 + 8 * (v__6 + ...
    v__2 - v__4) ^ 2) * r__2 + 16 * r__1 * (v__7 - v__1 + v__3 - ...
    v__5) * (v__6 + v__2 - v__4)) * b__3 + (4 * v__7 ^ 2 + (4 * ...
    v__1 - 4 * v__5) * v__7 - 8 * v__1 ^ 2 + (12 * v__3 - 8 * v__5) ...
    * v__1 - 4 * v__3 ^ 2 + 4 * v__3 * v__5 + 4 * (v__6 + v__2 - v__4)...
    ^ 2) * r__2 ^ 2 + 16 * r__1 * (v__7 - v__1 + v__3 - v__5) * (v__6 ...
    + v__2 - v__4) * r__2 - 4 * (v__1 * v__3 - v__1 ^ 2 + v__2 ^ 2 + ...
    v__6 ^ 2 - w__8 ^ 2 - v__3 * v__5 - w__4 ^ 2 - w__6 ^ 2 + v__4 ^ 2 + ...
    w__3 ^ 2 - w__7 ^ 2 - 2 * w__9 ^ 2 + v__5 ^ 2 + 2 * v__7 ^ 2 + 2 * ...
    w__1 ^ 2 - w__2 ^ 2 + (-w__5 + w__9) * w__3 + (2 * w__6 - 2 * w__8) *...
    w__4 + (w__7 - 2 * w__9) * w__5 + 2 * w__6 * w__8 + (-3 * w__3 + 2 * ...
    w__5 - w__7) * w__1 + (2 * w__4 - 2 * w__6 + 2 * w__8) * w__2 + (2 * ...
    v__6 - 2 * v__4) * v__2 + (-v__1 + 2 * v__3 - 3 * v__5) * v__7 - 2 * ...
    v__6 * v__4 + 3 * w__7 * w__9) * b__5 ^ 2 * s__r4 ^ 2 + 4 * r__1 ^ 2 *...
    (v__7 - v__1 + v__3 - v__5) ^ 2;

e_15 = (4 * (v__7 - v__1 + v__3 - v__5) * (v__6 + v__2 - v__4) * b__3 ^ 2) +...
    0.8e1 * (v__7 - v__1 + v__3 - v__5) * (((v__6 + v__2 - v__4) * r__2) +...
    (r__1 * (v__7 - v__1 + v__3 - v__5)) / 0.2e1) * b__3 + (4 * (v__7 - v__1 +...
    v__3 - v__5) * (v__6 + v__2 - v__4) * r__2 ^ 2) + (4 * r__1 * (v__7 - v__1 + ...
    v__3 - v__5) ^ 2 * r__2) - (4 * ((-v__6 - v__2 + v__4) * v__1 + (v__6 + v__2 ...
    - v__4) * v__3 + (-v__6 - v__2 + v__4) * v__5 + (v__6 + v__2 - v__4) * v__7 +...
    (w__2 - w__4 + w__6 - w__8) * (w__1 - w__3 + w__5 - w__7 + w__9)) * b__5 ^ 2 * s__r4 ^ 2);

e_16 = b__5 ^ 2 * (w__5 - w__7 + w__9 - v__1 + v__3 - v__5 + v__7 + w__1 - ...
    w__3) * (w__5 - w__7 + w__9 + v__1 - v__3 + v__5 - v__7 + w__1 - ...
    w__3) * s__r4 ^ 2 + (v__1 - v__3 + v__5 - v__7) ^ 2 * (b__3 + r__2) ^ 2;

T=roots([e_16,e_15,e_14,e_13,e_12,e_11,e_10,e_9,e_8,e_7,e_6,e_5,e_4,e_3,e_2,e_1,e_0]);

%% Obtaining joint angles back substitution
% Finding theta_1 fron eqn 26.
% T = tan(theta_1/2)
% The 0.001 value is se to neglect the imaginary parts of a number when is
% below it (test). 
thetas1 = 2*atan( real(T( imag(T)<0.001 & imag(T)>-0.001) ));
 if(isempty(thetas1))
  thetas1=0.1;
 end
s__1 = sin(thetas1);
c__1 = cos(thetas1);

% Finding theta_4 from eqn (22) and (23)
c__4 = 1/(b__5*s__r4)*(r__1*s__1-r__2*c__1+b__3);
V = v__1*c__1.^3 + v__2*(c__1.^2).*s__1 + v__3*c__1.^2 + v__4*(c__1.*s__1) + v__5*c__1 + ...
    v__6*s__1+v__7;
if(V==0)
   error('V is equal to zero') 
end

W = w__1*c__1.^4 + w__2*(c__1.^3).*s__1 + w__3*c__1.^3 + w__4*(c__1.^2).*s__1 +...
    w__5*c__1.^2 + w__6*c__1.*s__1 + w__7*c__1 + w__8*s__1 + w__9;
s__4 = -W./V;
thetas4 = atan2(s__4,c__4);

% Finding theta3_2 from eqn (18) and (19)

B__1 = 2*(r__3 - b__1)* b__5*s__r4*s__4 - ...
    2*(r__1*c__1 + r__2*s__1)*(b__5*c__r4 + b__4);
B__2 = -2*(b__5*c__r4 + b__4)*(r__3 - b__1) - ...
    (2*(r__1*c__1 + r__2*s__1)*b__5*s__r4).*s__4;
B__3 = (r__3 - b__1)^2 + (r__1*c__1+r__2*s__1).^ 2 +...
    (b__5*c__r4 + b__4)^2 + (b__5^2)*(s__r4^2)*(s__4.^2) - a__2^2;

A__1 = (c__1 * q__13 + q__23 * s__1) * c__r4 - q__33 * s__r4 * s__4;
A__2 = q__33 * c__r4 + ((c__1 * q__13 + q__23 * s__1) * s__r4).*s__4;
A__3 = c__r5 + ((-c__1 * q__23 + q__13 * s__1) * s__r4).*c__4;

nSol = length(thetas1);
c__32 = zeros(nSol,1);
s__32 = zeros(nSol,1);

for n=1:nSol
    
x = ([A__1(n,1),A__2(n,1);B__1(n,1),B__2(n,1)])\([-A__3(n,1);-B__3(n,1)]);
s__32(n,1) = x(1);
c__32(n,1) = x(2);
end

thetas32 = atan2(s__32,c__32);

% Finding theta_5 from eqn (15) and (14)
c__5 = ( q__13*c__1.*s__32 + q__23*s__1.*s__32 + q__33*c__32 + ...
    c__r4*c__r5 )/(s__r4*s__r5);

s__5 = (q__13*s__1 - q__23*c__1 + c__r4*s__r5*c__4.*c__5 + s__r4*c__r5*c__4)...
    ./(s__r5*s__4);

thetas5 = atan2(s__5,c__5);

% Finding theta_2 from equations (9) and (10)
c__2 = (r__1*c__1 + r__2*s__1 - b__5*s__r4*c__32.*s__4 - ...
    (b__4 + b__5*c__r4)*s__32)/a__2;
s__2 = (r__3 - b__1 + b__5*s__r5*s__32.*s__4 -...
    (b__4 + b__5*c__r4)*c__32)/a__2;

thetas2 = atan2(s__2,c__2);

%Finding theta3 theta32 = theta3 - theta2
thetas3 = thetas32+thetas2;


%Finding theta_6 from equation (12), components (3,1) and (3,2)
% Equation (32) and (33) solve system of equations

y1 = q__11*c__1.*s__32 + q__21*s__1.*s__32 + q__31*c__32;
y2 = q__12*c__1.*s__32 + q__22*s__1.*s__32 + q__32*c__32;
a1 = s__r4*s__5;
a2 = s__r4*c__r5*c__5 + c__r4*s__r5;
a3 = -(s__r4*c__r5*c__5 + c__r4*s__r5);
a4 = s__r4*s__5;

c__6 = zeros(nSol,1);
s__6 = zeros(nSol,1);

for n=1:nSol
    
x = ([a1(n,1),a2(n,1);a3(n,1),a4(n,1)])\([y1(n,1);y2(n,1)]);
s__6(n,1) = x(2);
c__6(n,1) = x(1);
end

thetas6 = atan2(s__6,c__6);
%t=1;
q1 = thetas1(t);
q2 = thetas2(t);
q3 = thetas3(t);
q4 = thetas4(t);
q5 = thetas5(t);
q6 = thetas6(t);


end
